simulink model "ABB_1010"  (R2024a)
settings: Solver=VariableStepAuto  StartTime=0.0  StopTime=200  RelTol=1e-3
model workspace: external: MATLAB File C:\Users\lucas\OneDrive\Documents\MATLAB\projeto final\ABB_1010_DataFile.m (data not in the file)
values from neighbouring files (symbols this model uses):
  g = 9.81    [inicializacaoAntropomorfico.m]
  I1 = [ 0.00243841  0.00000307  0.00007261    [inicializacaoAntropomorfico.m]
  I2 = [ 0.01633569  0.00000387 -0.00034405    [inicializacaoAntropomorfico.m]
  I3 = [ 0.00244760 -0.00000208  0.00000538    [inicializacaoAntropomorfico.m]
  I4 = [ 0.00245792 -0.00000008  0.00003121    [inicializacaoAntropomorfico.m]
  I5 = [ 0.00062165 -0.00000206 -0.00000303    [inicializacaoAntropomorfico.m]
  I6 = [ 0.00000357  0.00000000  0.00000000    [inicializacaoAntropomorfico.m]
  I7 = [(m7*L7^2)/12 0.00000000  0.00000000    [inicializacaoAntropomorfico.m]
  L = [L1, L2, L3, L4, L5, L6, L7]    [inicializacaoAntropomorfico.m]
  Lcm1 = [-0.00258308  0.00024508 -0.01434968]    [inicializacaoAntropomorfico.m]
  Lcm2 = [-0.02078894  0.00020016 -0.10516734]    [inicializacaoAntropomorfico.m]
  Lcm3 = [ 0.00021912  0.00015355 -0.06228290]    [inicializacaoAntropomorfico.m]
  Lcm4 = [-0.00172658 -0.00124140 -0.07369196]    [inicializacaoAntropomorfico.m]
  Lcm5 = [-0.00014110  0.00085992 -0.03825278]    [inicializacaoAntropomorfico.m]
  Lcm6 = [ 0.00002478  0.00000000 -0.00042157]    [inicializacaoAntropomorfico.m]
  Lcm7 = [ 0           0          -0.05000000]    [inicializacaoAntropomorfico.m]
  m = [m1, m2, m3, m4, m5, m6, m7]    [inicializacaoAntropomorfico.m]
  Pf = [  0.05    [inicializacaoAntropomorfico.m]
  Pi = [  0.2    [inicializacaoAntropomorfico.m]
  Raio = [0]    [inicializacaoAntropomorfico.m]
  Sentido = [0]    [inicializacaoAntropomorfico.m]
  Tipo = [1]    [inicializacaoAntropomorfico.m]
undefined symbols (not defined in the file or in its folder): smiData, X, Y, Z
libraries: sm_lib x35, nesl_utility x7
(part 8 of 16)

== matlab function ABB_1010/Dinamica/MATLAB Function3 ==
  data: Q input; I1 parameter; I2 parameter; L parameter; dQ input; Lcm1 parameter; Lcm2 parameter; Lcm3 parameter; Lcm4 parameter; Lcm5 parameter; Lcm6 parameter; I5 parameter; I4 parameter; I3 parameter; C output; I6 parameter; m parameter
function C = func_C(Q, I1, I2, L, dQ, Lcm1, Lcm2, Lcm3, Lcm4, Lcm5, Lcm6, I5, I4, I3, I6, m)
%func_C
%    OUT1 = func_C(Ixx2,Ixx3,Ixx4,Ixx5,Ixx6,Ixy3,Ixy4,Ixy5,Ixy6,Ixz2,Ixz3,Ixz4,Ixz5,Ixz6,Iyx3,Iyx4,Iyx5,Iyx6,Iyy4,Iyy5,Iyy6,Iyz3,Iyz4,Iyz5,Iyz6,Izx2,Izx3,Izx4,Izx5,Izx6,Izy3,Izy4,Izy5,Izy6,Izz2,Izz3,Izz4,Izz5,Izz6,Lx2,Lx3,Lxcm2,Lxcm3,Lxcm4,Lxcm5,Lxcm6,Lycm3,Lycm4,Lycm5,Lycm6,Lz4,Lz5,Lzcm2,Lzcm3,Lzcm4,Lzcm5,Lzcm6,Q2,Q3,Q4,Q5,Q6,dQ1,dQ2,dQ3,dQ4,dQ5,dQ6,M2,M3,M4,M5,M6)

%    This function was generated by the Symbolic Math Toolbox version 24.1.
%    30-Apr-2025 06:24:11

m1  = m(1);
m2  = m(2);
m3  = m(3);
m4  = m(4);
m5  = m(5);
m6  = m(6);

Q1  = Q(1);
Q2  = Q(2);
Q3  = Q(3);
Q4  = Q(4);
Q5  = Q(5);
Q6  = Q(6);

dQ1 = dQ(1);
dQ2 = dQ(2);
dQ3 = dQ(3);
dQ4 = dQ(4);
dQ5 = dQ(5);
dQ6 = dQ(6);

Lz1 = L(1);
Lx2 = L(2);
Lx3 = L(3);
Lz4 = L(4);
Lz5 = L(5);
Lz6 = L(6);

Lxcm1 = Lcm1(1);
Lycm1 = Lcm1(2);
Lzcm1 = Lcm1(3);

Lxcm2 = Lcm2(1);
Lycm2 = Lcm2(2);
Lzcm2 = Lcm2(3);

Lxcm3 = Lcm3(1);
Lycm3 = Lcm3(2);
Lzcm3 = Lcm3(3);

Lxcm4 = Lcm4(1);
Lycm4 = Lcm4(2);
Lzcm4 = Lcm4(3);

Lxcm5 = Lcm5(1);
Lycm5 = Lcm5(2);
Lzcm5 = Lcm5(3);

Lxcm6 = Lcm6(1);
Lycm6 = Lcm6(2);
Lzcm6 = Lcm6(3);

Ixx1 = I1(1,1);
Ixy1 = I1(1,2);
Ixz1 = I1(1,3);
Iyx1 = I1(2,1);
Iyy1 = I1(2,2);
Iyz1 = I1(2,3);
Izx1 = I1(3,1);
Izy1 = I1(3,2);
Izz1 = I1(3,3);

Ixx2 = I2(1,1);
Ixy2 = I2(1,2);
Ixz2 = I2(1,3);
Iyx2 = I2(2,1);
Iyy2 = I2(2,2);
Iyz2 = I2(2,3);
Izx2 = I2(3,1);
Izy2 = I2(3,2);
Izz2 = I2(3,3);

Ixx3 = I3(1,1);
Ixy3 = I3(1,2);
Ixz3 = I3(1,3);
Iyx3 = I3(2,1);
Iyy3 = I3(2,2);
Iyz3 = I3(2,3);
Izx3 = I3(3,1);
Izy3 = I3(3,2);
Izz3 = I3(3,3);

Ixx4 = I4(1,1);
Ixy4 = I4(1,2);
Ixz4 = I4(1,3);
Iyx4 = I4(2,1);
Iyy4 = I4(2,2);
Iyz4 = I4(2,3);
Izx4 = I4(3,1);
Izy4 = I4(3,2);
Izz4 = I4(3,3);

Ixx5 = I5(1,1);
Ixy5 = I5(1,2);
Ixz5 = I5(1,3);
Iyx5 = I5(2,1);
Iyy5 = I5(2,2);
Iyz5 = I5(2,3);
Izx5 = I5(3,1);
Izy5 = I5(3,2);
Izz5 = I5(3,3);

Ixx6 = I6(1,1);
Ixy6 = I6(1,2);
Ixz6 = I6(1,3);
Iyx6 = I6(2,1);
Iyy6 = I6(2,2);
Iyz6 = I6(2,3);
Izx6 = I6(3,1);
Izy6 = I6(3,2);
Izz6 = I6(3,3);

t2 = cos(Q2);
t3 = cos(Q3);
t4 = cos(Q4);
t5 = cos(Q5);
t6 = cos(Q6);
t7 = sin(Q2);
t8 = sin(Q3);
t9 = sin(Q4);
t10 = sin(Q5);
t11 = sin(Q6);
t12 = Lx2.^2;
t13 = Lx3.^2;
t14 = Lxcm3.^2;
t15 = Lxcm4.^2;
t16 = Lxcm5.^2;
t17 = Lxcm6.^2;
t18 = Lycm4.^2;
t19 = Lycm5.^2;
t20 = Lycm6.^2;
t21 = Lz4.^2;
t22 = Lz5.^2;
t23 = Lzcm3.^2;
t24 = Lzcm4.^2;
t25 = Lzcm5.^2;
t26 = Lzcm6.^2;
t27 = Q2.*2.0;
t28 = Q3.*2.0;
t29 = Q4.*2.0;
t30 = Q5.*2.0;
t31 = Q6.*2.0;
t42 = Ixy4.*dQ2.*dQ4;
t43 = Ixy4.*dQ3.*dQ4;
t44 = Ixz5.*dQ2.*dQ5;
t45 = Ixz5.*dQ3.*dQ5;
t46 = Iyx4.*dQ2.*dQ4;
t47 = Iyx4.*dQ3.*dQ4;
t48 = Izx5.*dQ2.*dQ5;
t49 = Izx5.*dQ3.*dQ5;
t78 = Lxcm4.*Lycm4.*dQ2.*dQ4.*m4.*2.0;
t79 = Lxcm4.*Lycm4.*dQ3.*dQ4.*m4.*2.0;
t80 = Lxcm5.*Lzcm5.*dQ2.*dQ5.*m5.*2.0;
t81 = Lxcm5.*Lzcm5.*dQ3.*dQ5.*m5.*2.0;
t32 = t2.^2;
t33 = t3.^2;
t34 = t4.^2;
t35 = t5.^2;
t36 = t6.^2;
t37 = sin(t27);
t38 = sin(t28);
t39 = sin(t29);
t40 = sin(t30);
t41 = sin(t31);
t50 = Ixy5.*dQ2.*dQ4.*t5;
t51 = Ixy5.*dQ3.*dQ4.*t5;
t52 = Ixy6.*dQ2.*dQ4.*t5;
t53 = Ixy6.*dQ3.*dQ4.*t5;
t54 = Ixy6.*dQ5.*dQ6.*t4;
t55 = Ixz6.*dQ2.*dQ5.*t6;
t56 = Ixz6.*dQ3.*dQ5.*t6;
t57 = Iyx5.*dQ2.*dQ4.*t5;
t58 = Iyx5.*dQ3.*dQ4.*t5;
t59 = Iyx6.*dQ2.*dQ4.*t5;
t60 = Iyx6.*dQ3.*dQ4.*t5;
t61 = Iyx6.*dQ5.*dQ6.*t4;
t62 = Izx6.*dQ2.*dQ5.*t6;
t63 = Izx6.*dQ3.*dQ5.*t6;
t64 = Ixx5.*dQ4.*dQ5.*t9;
t65 = Ixx6.*dQ4.*dQ5.*t9;
t66 = Iyy5.*dQ4.*dQ5.*t9;
t67 = Iyy6.*dQ4.*dQ5.*t9;
t68 = Iyz5.*dQ2.*dQ4.*t10;
t69 = Iyz5.*dQ3.*dQ4.*t10;
t70 = Iyz6.*dQ2.*dQ5.*t11;
t71 = Iyz6.*dQ3.*dQ5.*t11;
t72 = Izy5.*dQ2.*dQ4.*t10;
t73 = Izy5.*dQ3.*dQ4.*t10;
t74 = Izy6.*dQ2.*dQ5.*t11;
t75 = Izy6.*dQ3.*dQ5.*t11;
t76 = Izz5.*dQ4.*dQ5.*t9;
t77 = Izz6.*dQ4.*dQ5.*t9;
t126 = Ixx4.*dQ1.*dQ4.*t2.*t8;
t127 = Ixx4.*dQ1.*dQ4.*t3.*t7;
t128 = Ixx5.*dQ1.*dQ4.*t2.*t8;
t129 = Ixx5.*dQ1.*dQ4.*t3.*t7;
t130 = Ixx6.*dQ1.*dQ4.*t2.*t8;
t131 = Ixx6.*dQ1.*dQ4.*t3.*t7;
t132 = Ixx6.*dQ4.*dQ6.*t4.*t10;
t133 = Ixx6.*dQ5.*dQ6.*t5.*t9;
t134 = Iyy4.*dQ1.*dQ4.*t2.*t8;
t135 = Iyy4.*dQ1.*dQ4.*t3.*t7;
t136 = Iyy5.*dQ1.*dQ4.*t2.*t8;
t137 = Iyy5.*dQ1.*dQ4.*t3.*t7;
t138 = Iyy6.*dQ1.*dQ4.*t2.*t8;
t139 = Iyy6.*dQ1.*dQ4.*t3.*t7;
t140 = Iyy6.*dQ4.*dQ6.*t4.*t10;
t141 = Iyy6.*dQ5.*dQ6.*t5.*t9;
t142 = Iyz6.*dQ2.*dQ4.*t6.*t10;
t143 = Iyz6.*dQ3.*dQ4.*t6.*t10;
t144 = Izy6.*dQ2.*dQ4.*t6.*t10;
t145 = Izy6.*dQ3.*dQ4.*t6.*t10;
t146 = Izz4.*dQ1.*dQ4.*t2.*t8;
t147 = Izz4.*dQ1.*dQ4.*t3.*t7;
t148 = Izz5.*dQ1.*dQ4.*t2.*t8;
t149 = Izz5.*dQ1.*dQ4.*t3.*t7;
t150 = Izz6.*dQ1.*dQ4.*t2.*t8;
t151 = Izz6.*dQ1.*dQ4.*t3.*t7;
t152 = Izz6.*dQ4.*dQ6.*t4.*t10;
t153 = Izz6.*dQ5.*dQ6.*t5.*t9;
t154 = Ixz6.*dQ2.*dQ4.*t10.*t11;
t155 = Ixz6.*dQ3.*dQ4.*t10.*t11;
t156 = Izx6.*dQ2.*dQ4.*t10.*t11;
t157 = Izx6.*dQ3.*dQ4.*t10.*t11;
t166 = Lx3.*Lycm4.*dQ2.*dQ4.*m4.*t4.*2.0;
t167 = Lx3.*Lycm4.*dQ3.*dQ4.*m4.*t4.*2.0;
t168 = Lx3.*Lycm5.*dQ2.*dQ4.*m5.*t4.*2.0;
t169 = Lx3.*Lycm5.*dQ3.*dQ4.*m5.*t4.*2.0;
t170 = Lxcm5.*Lycm5.*dQ2.*dQ4.*m5.*t5.*2.0;
t171 = Lxcm5.*Lycm5.*dQ3.*dQ4.*m5.*t5.*2.0;
t172 = Lxcm6.*Lycm6.*dQ2.*dQ4.*m6.*t5.*2.0;
t173 = Lxcm6.*Lycm6.*dQ3.*dQ4.*m6.*t5.*2.0;
t174 = Lxcm6.*Lycm6.*dQ5.*dQ6.*m6.*t4.*2.0;
t175 = Lxcm5.*Lz4.*dQ2.*dQ5.*m5.*t5.*2.0;
t176 = Lxcm5.*Lz4.*dQ3.*dQ5.*m5.*t5.*2.0;
t177 = Lxcm6.*Lz5.*dQ2.*dQ5.*m6.*t6.*2.0;
t178 = Lxcm6.*Lz5.*dQ3.*dQ5.*m6.*t6.*2.0;
t179 = Lxcm6.*Lzcm6.*dQ2.*dQ5.*m6.*t6.*2.0;
t180 = Lxcm6.*Lzcm6.*dQ3.*dQ5.*m6.*t6.*2.0;
t181 = Lx3.*Lxcm4.*dQ2.*dQ4.*m4.*t9.*2.0;
t182 = Lx3.*Lxcm4.*dQ3.*dQ4.*m4.*t9.*2.0;
t183 = Lycm6.*Lz5.*dQ2.*dQ5.*m6.*t11.*2.0;
t184 = Lycm6.*Lz5.*dQ3.*dQ5.*m6.*t11.*2.0;
t185 = Lycm5.*Lzcm5.*dQ2.*dQ4.*m5.*t10.*2.0;
t186 = Lycm5.*Lzcm5.*dQ3.*dQ4.*m5.*t10.*2.0;
t187 = Lycm6.*Lzcm6.*dQ2.*dQ5.*m6.*t11.*2.0;
t188 = Lycm6.*Lzcm6.*dQ3.*dQ5.*m6.*t11.*2.0;
t189 = Lz4.*Lz5.*dQ2.*dQ5.*m6.*t10.*2.0;
t190 = Lz4.*Lz5.*dQ3.*dQ5.*m6.*t10.*2.0;
t191 = Lz4.*Lzcm5.*dQ2.*dQ5.*m5.*t10.*2.0;
t192 = Lz4.*Lzcm5.*dQ3.*dQ5.*m5.*t10.*2.0;
t193 = Lz4.*Lzcm6.*dQ2.*dQ5.*m6.*t10.*2.0;
t194 = Lz4.*Lzcm6.*dQ3.*dQ5.*m6.*t10.*2.0;
t195 = dQ4.*dQ5.*m5.*t9.*t16.*2.0;
t196 = dQ4.*dQ5.*m6.*t9.*t20.*2.0;
t221 = Ixz4.*dQ1.*dQ4.*t2.*t3.*t4;
t222 = Ixz5.*dQ1.*dQ4.*t2.*t3.*t4;
t223 = Ixz6.*dQ4.*dQ6.*t4.*t5.*t6;
t224 = Izx4.*dQ1.*dQ4.*t2.*t3.*t4;
t225 = Izx5.*dQ1.*dQ4.*t2.*t3.*t4;
t226 = Izx6.*dQ4.*dQ6.*t4.*t5.*t6;
t237 = Ixx5.*dQ1.*dQ5.*t2.*t3.*t9;
t238 = Ixx6.*dQ1.*dQ5.*t2.*t3.*t9;
t239 = Ixx6.*dQ1.*dQ6.*t2.*t5.*t8;
t240 = Ixx6.*dQ1.*dQ6.*t3.*t5.*t7;
t241 = Iyy5.*dQ1.*dQ5.*t2.*t3.*t9;
t242 = Iyy6.*dQ1.*dQ5.*t2.*t3.*t9;
t243 = Iyy6.*dQ1.*dQ6.*t2.*t5.*t8;
t244 = Iyy6.*dQ1.*dQ6.*t3.*t5.*t7;
t245 = Iyz4.*dQ1.*dQ4.*t2.*t3.*t9;
t246 = Iyz5.*dQ1.*dQ5.*t2.*t5.*t8;
t247 = Iyz5.*dQ1.*dQ5.*t3.*t5.*t7;
t248 = Iyz5.*dQ2.*dQ5.*t4.*t5.*t9;
t249 = Iyz5.*dQ3.*dQ5.*t4.*t5.*t9;
t250 = Iyz6.*dQ2.*dQ6.*t5.*t6.*t10;
t251 = Iyz6.*dQ3.*dQ6.*t5.*t6.*t10;
t252 = Iyz6.*dQ4.*dQ6.*t4.*t5.*t11;
t253 = Izy4.*dQ1.*dQ4.*t2.*t3.*t9;
t254 = Izy5.*dQ1.*dQ5.*t2.*t5.*t8;
t255 = Izy5.*dQ1.*dQ5.*t3.*t5.*t7;
t256 = Izy5.*dQ2.*dQ5.*t4.*t5.*t9;
t257 = Izy5.*dQ3.*dQ5.*t4.*t5.*t9;
t258 = Izy6.*dQ2.*dQ6.*t5.*t6.*t10;
t259 = Izy6.*dQ3.*dQ6.*t5.*t6.*t10;
t260 = Izy6.*dQ4.*dQ6.*t4.*t5.*t11;
t261 = Izz5.*dQ1.*dQ5.*t2.*t3.*t9;
t262 = Izz6.*dQ1.*dQ5.*t2.*t3.*t9;
t263 = Izz6.*dQ1.*dQ6.*t2.*t5.*t8;
t264 = Izz6.*dQ1.*dQ6.*t3.*t5.*t7;
t265 = Ixy5.*dQ1.*dQ5.*t2.*t8.*t10;
t266 = Ixy5.*dQ1.*dQ5.*t3.*t7.*t10;
t267 = Ixy6.*dQ1.*dQ5.*t2.*t8.*t10;
t268 = Ixy6.*dQ1.*dQ5.*t3.*t7.*t10;
t269 = Ixy5.*dQ2.*dQ5.*t4.*t9.*t10;
t270 = Ixy5.*dQ3.*dQ5.*t4.*t9.*t10;
t271 = Ixy6.*dQ2.*dQ5.*t4.*t9.*t10;
t272 = Ixy6.*dQ3.*dQ5.*t4.*t9.*t10;
t273 = Ixy6.*dQ4.*dQ6.*t5.*t9.*t10;
t274 = Ixz4.*dQ1.*dQ4.*t4.*t7.*t8;
t275 = Ixz5.*dQ1.*dQ4.*t4.*t7.*t8;
t276 = Ixz6.*dQ2.*dQ6.*t5.*t10.*t11;
t277 = Ixz6.*dQ3.*dQ6.*t5.*t10.*t11;
t278 = Iyx5.*dQ1.*dQ5.*t2.*t8.*t10;
t279 = Iyx5.*dQ1.*dQ5.*t3.*t7.*t10;
t280 = Iyx6.*dQ1.*dQ5.*t2.*t8.*t10;
t281 = Iyx6.*dQ1.*dQ5.*t3.*t7.*t10;
t282 = Iyx5.*dQ2.*dQ5.*t4.*t9.*t10;
t283 = Iyx5.*dQ3.*dQ5.*t4.*t9.*t10;
t284 = Iyx6.*dQ2.*dQ5.*t4.*t9.*t10;
t285 = Iyx6.*dQ3.*dQ5.*t4.*t9.*t10;
t286 = Iyx6.*dQ4.*dQ6.*t5.*t9.*t10;
t287 = Izx4.*dQ1.*dQ4.*t4.*t7.*t8;
t288 = Izx5.*dQ1.*dQ4.*t4.*t7.*t8;
t289 = Izx6.*dQ2.*dQ6.*t5.*t10.*t11;
t290 = Izx6.*dQ3.*dQ6.*t5.*t10.*t11;
t291 = Ixx5.*dQ1.*dQ5.*t7.*t8.*t9;
t292 = Ixx6.*dQ1.*dQ5.*t7.*t8.*t9;
t293 = Iyy5.*dQ1.*dQ5.*t7.*t8.*t9;
t294 = Iyy6.*dQ1.*dQ5.*t7.*t8.*t9;
t295 = Iyz4.*dQ1.*dQ4.*t7.*t8.*t9;
t296 = Izy4.*dQ1.*dQ4.*t7.*t8.*t9;
t297 = Izz5.*dQ1.*dQ5.*t7.*t8.*t9;
t298 = Izz6.*dQ1.*dQ5.*t7.*t8.*t9;
t399 = Lx3.*Lycm6.*dQ2.*dQ4.*m6.*t4.*t6.*2.0;
t400 = Lx3.*Lycm6.*dQ3.*dQ4.*m6.*t4.*t6.*2.0;
t401 = Lx3.*Lycm6.*dQ5.*dQ6.*m6.*t5.*t6.*2.0;
t402 = Lx3.*Lz5.*dQ2.*dQ5.*m6.*t4.*t5.*2.0;
t403 = Lx3.*Lz5.*dQ3.*dQ5.*m6.*t4.*t5.*2.0;
t404 = Lx3.*Lzcm5.*dQ2.*dQ5.*m5.*t4.*t5.*2.0;
t405 = Lx3.*Lzcm5.*dQ3.*dQ5.*m5.*t4.*t5.*2.0;
t406 = Lx3.*Lzcm6.*dQ2.*dQ5.*m6.*t4.*t5.*2.0;
t407 = Lx3.*Lzcm6.*dQ3.*dQ5.*m6.*t4.*t5.*2.0;
t408 = Lxcm6.*Lz4.*dQ2.*dQ5.*m6.*t5.*t6.*2.0;
t409 = Lxcm6.*Lz4.*dQ3.*dQ5.*m6.*t5.*t6.*2.0;
t410 = Lxcm6.*Lz4.*dQ4.*dQ6.*m6.*t4.*t6.*2.0;
t411 = Ixx6.*dQ2.*dQ6.*t4.*t5.*t9.*2.0;
t412 = Ixx6.*dQ3.*dQ6.*t4.*t5.*t9.*2.0;
t413 = Ixx6.*dQ2.*dQ4.*t5.*t6.*t11.*2.0;
t414 = Ixx6.*dQ3.*dQ4.*t5.*t6.*t11.*2.0;
t415 = Ixx6.*dQ5.*dQ6.*t4.*t6.*t11.*2.0;
t416 = Iyy6.*dQ2.*dQ6.*t4.*t5.*t9.*2.0;
t417 = Iyy6.*dQ3.*dQ6.*t4.*t5.*t9.*2.0;
t418 = Iyy6.*dQ2.*dQ4.*t5.*t6.*t11.*2.0;
t419 = Iyy6.*dQ3.*dQ4.*t5.*t6.*t11.*2.0;
t420 = Iyy6.*dQ5.*dQ6.*t4.*t6.*t11.*2.0;
t421 = Lx3.*Lxcm5.*dQ2.*dQ4.*m5.*t5.*t9.*2.0;
t422 = Lx3.*Lxcm5.*dQ2.*dQ5.*m5.*t4.*t10.*2.0;
t423 = Lx3.*Lxcm5.*dQ3.*dQ4.*m5.*t5.*t9.*2.0;
t424 = Lx3.*Lxcm5.*dQ3.*dQ5.*m5.*t4.*t10.*2.0;
t425 = Lx3.*Lxcm6.*dQ2.*dQ4.*m6.*t4.*t11.*2.0;
t426 = Lx3.*Lxcm6.*dQ3.*dQ4.*m6.*t4.*t11.*2.0;
t427 = Lx3.*Lxcm6.*dQ2.*dQ6.*m6.*t6.*t9.*2.0;
t428 = Lx3.*Lxcm6.*dQ3.*dQ6.*m6.*t6.*t9.*2.0;
t429 = Lx3.*Lxcm6.*dQ5.*dQ6.*m6.*t5.*t11.*2.0;
t430 = Lycm6.*Lz4.*dQ2.*dQ5.*m6.*t5.*t11.*2.0;
t431 = Lycm6.*Lz5.*dQ2.*dQ4.*m6.*t6.*t10.*2.0;
t432 = Lycm6.*Lz4.*dQ2.*dQ6.*m6.*t6.*t10.*2.0;
t433 = Lycm6.*Lz4.*dQ3.*dQ5.*m6.*t5.*t11.*2.0;
t434 = Lycm6.*Lz5.*dQ3.*dQ4.*m6.*t6.*t10.*2.0;
t435 = Lycm6.*Lz4.*dQ3.*dQ6.*m6.*t6.*t10.*2.0;
t436 = Lycm6.*Lz4.*dQ4.*dQ6.*m6.*t4.*t11.*2.0;
t437 = Lycm6.*Lzcm6.*dQ2.*dQ4.*m6.*t6.*t10.*2.0;
t438 = Lycm6.*Lzcm6.*dQ3.*dQ4.*m6.*t6.*t10.*2.0;
t439 = Lz4.*Lz5.*dQ4.*dQ5.*m6.*t5.*t9.*2.0;
t440 = Lz4.*Lzcm5.*dQ4.*dQ5.*m5.*t5.*t9.*2.0;
t441 = Lz4.*Lzcm6.*dQ4.*dQ5.*m6.*t5.*t9.*2.0;
t442 = Ixy6.*dQ4.*dQ5.*t6.*t9.*t11.*2.0;
t443 = Ixz5.*dQ4.*dQ5.*t5.*t9.*t10.*2.0;
t444 = Iyx6.*dQ4.*dQ5.*t6.*t9.*t11.*2.0;
t445 = Izx5.*dQ4.*dQ5.*t5.*t9.*t10.*2.0;
t446 = Lx3.*Lycm6.*dQ2.*dQ6.*m6.*t9.*t11.*2.0;
t447 = Lx3.*Lycm6.*dQ3.*dQ6.*m6.*t9.*t11.*2.0;
t448 = Lx3.*Lz5.*dQ2.*dQ4.*m6.*t9.*t10.*2.0;
t449 = Lx3.*Lz5.*dQ3.*dQ4.*m6.*t9.*t10.*2.0;
t450 = Lx3.*Lzcm5.*dQ2.*dQ4.*m5.*t9.*t10.*2.0;
t451 = Lx3.*Lzcm5.*dQ3.*dQ4.*m5.*t9.*t10.*2.0;
t452 = Lx3.*Lzcm6.*dQ2.*dQ4.*m6.*t9.*t10.*2.0;
t453 = Lx3.*Lzcm6.*dQ3.*dQ4.*m6.*t9.*t10.*2.0;
t454 = Lxcm5.*Lz4.*dQ4.*dQ5.*m5.*t9.*t10.*2.0;
t455 = Lxcm6.*Lz5.*dQ2.*dQ4.*m6.*t10.*t11.*2.0;
t456 = Lxcm6.*Lz4.*dQ2.*dQ6.*m6.*t10.*t11.*2.0;
t457 = Lxcm6.*Lz5.*dQ3.*dQ4.*m6.*t10.*t11.*2.0;
t458 = Lxcm6.*Lz4.*dQ3.*dQ6.*m6.*t10.*t11.*2.0;
t459 = Lxcm6.*Lzcm6.*dQ2.*dQ4.*m6.*t10.*t11.*2.0;
t460 = Lxcm6.*Lzcm6.*dQ3.*dQ4.*m6.*t10.*t11.*2.0;
t485 = Ixz6.*dQ1.*dQ4.*t2.*t3.*t4.*t6;
t486 = Izx6.*dQ1.*dQ4.*t2.*t3.*t4.*t6;
t498 = Ixx6.*dQ1.*dQ6.*t2.*t3.*t4.*t10;
t499 = Iyy6.*dQ1.*dQ6.*t2.*t3.*t4.*t10;
t500 = Iyz5.*dQ1.*dQ4.*t2.*t3.*t5.*t9;
t501 = Iyz6.*dQ1.*dQ4.*t2.*t3.*t4.*t11;
t502 = Iyz6.*dQ1.*dQ5.*t2.*t5.*t6.*t8;
t503 = Iyz6.*dQ1.*dQ5.*t3.*t5.*t6.*t7;
t504 = Iyz6.*dQ2.*dQ5.*t4.*t5.*t6.*t9;
t505 = Iyz6.*dQ3.*dQ5.*t4.*t5.*t6.*t9;
t506 = Izy5.*dQ1.*dQ4.*t2.*t3.*t5.*t9;
t507 = Izy6.*dQ1.*dQ4.*t2.*t3.*t4.*t11;
t508 = Izy6.*dQ1.*dQ5.*t2.*t5.*t6.*t8;
t509 = Izy6.*dQ1.*dQ5.*t3.*t5.*t6.*t7;
t510 = Izy6.*dQ2.*dQ5.*t4.*t5.*t6.*t9;
t511 = Izy6.*dQ3.*dQ5.*t4.*t5.*t6.*t9;
t512 = Izz6.*dQ1.*dQ6.*t2.*t3.*t4.*t10;
t513 = Ixy5.*dQ1.*dQ4.*t2.*t3.*t9.*t10;
t514 = Ixy6.*dQ1.*dQ4.*t2.*t3.*t9.*t10;
t515 = Ixy6.*dQ1.*dQ6.*t2.*t4.*t8.*t9;
t516 = Ixy6.*dQ1.*dQ6.*t3.*t4.*t7.*t9;
t517 = Ixz5.*dQ1.*dQ5.*t2.*t4.*t8.*t9;
t518 = Ixz5.*dQ1.*dQ5.*t3.*t4.*t7.*t9;
t519 = Ixz6.*dQ1.*dQ4.*t4.*t6.*t7.*t8;
t520 = Ixz6.*dQ1.*dQ5.*t2.*t5.*t8.*t11;
t521 = Ixz6.*dQ1.*dQ5.*t3.*t5.*t7.*t11;
t522 = Ixz6.*dQ2.*dQ5.*t4.*t5.*t9.*t11;
t523 = Ixz6.*dQ2.*dQ6.*t4.*t6.*t9.*t10;
t524 = Ixz6.*dQ3.*dQ5.*t4.*t5.*t9.*t11;
t525 = Ixz6.*dQ3.*dQ6.*t4.*t6.*t9.*t10;
t526 = Iyx5.*dQ1.*dQ4.*t2.*t3.*t9.*t10;
t527 = Iyx6.*dQ1.*dQ4.*t2.*t3.*t9.*t10;
t528 = Iyx6.*dQ1.*dQ6.*t2.*t4.*t8.*t9;
t529 = Iyx6.*dQ1.*dQ6.*t3.*t4.*t7.*t9;
t530 = Izx5.*dQ1.*dQ5.*t2.*t4.*t8.*t9;
t531 = Izx5.*dQ1.*dQ5.*t3.*t4.*t7.*t9;
t532 = Izx6.*dQ1.*dQ4.*t4.*t6.*t7.*t8;
t533 = Izx6.*dQ1.*dQ5.*t2.*t5.*t8.*t11;
t534 = Izx6.*dQ1.*dQ5.*t3.*t5.*t7.*t11;
t535 = Izx6.*dQ2.*dQ5.*t4.*t5.*t9.*t11;
t536 = Izx6.*dQ2.*dQ6.*t4.*t6.*t9.*t10;
t537 = Izx6.*dQ3.*dQ5.*t4.*t5.*t9.*t11;
t538 = Izx6.*dQ3.*dQ6.*t4.*t6.*t9.*t10;
t539 = Ixx6.*dQ1.*dQ6.*t4.*t7.*t8.*t10;
t540 = Iyy6.*dQ1.*dQ6.*t4.*t7.*t8.*t10;
t541 = Iyz5.*dQ1.*dQ4.*t5.*t7.*t8.*t9;
t542 = Iyz6.*dQ1.*dQ4.*t4.*t7.*t8.*t11;
t543 = Iyz6.*dQ2.*dQ6.*t4.*t9.*t10.*t11;
t544 = Iyz6.*dQ3.*dQ6.*t4.*t9.*t10.*t11;
t545 = Izy5.*dQ1.*dQ4.*t5.*t7.*t8.*t9;
t546 = Izy6.*dQ1.*dQ4.*t4.*t7.*t8.*t11;
t547 = Izy6.*dQ2.*dQ6.*t4.*t9.*t10.*t11;
t548 = Izy6.*dQ3.*dQ6.*t4.*t9.*t10.*t11;
t549 = Izz6.*dQ1.*dQ6.*t4.*t7.*t8.*t10;
t550 = Ixy5.*dQ1.*dQ4.*t7.*t8.*t9.*t10;
t551 = Ixy6.*dQ1.*dQ4.*t7.*t8.*t9.*t10;
t552 = Iyx5.*dQ1.*dQ4.*t7.*t8.*t9.*t10;
t553 = Iyx6.*dQ1.*dQ4.*t7.*t8.*t9.*t10;
t615 = dQ1.*dQ4.*m6.*t2.*t8.*t17.*2.0;
t616 = dQ1.*dQ4.*m6.*t3.*t7.*t17.*2.0;
t617 = dQ5.*dQ6.*m6.*t5.*t9.*t17.*2.0;
t618 = dQ1.*dQ4.*m4.*t2.*t8.*t18.*2.0;
t619 = dQ1.*dQ4.*m4.*t3.*t7.*t18.*2.0;
t620 = dQ1.*dQ4.*m5.*t2.*t8.*t19.*2.0;
t621 = dQ1.*dQ4.*m5.*t3.*t7.*t19.*2.0;
t622 = dQ4.*dQ6.*m6.*t4.*t10.*t20.*2.0;
t644 = Lx3.*Lycm6.*dQ2.*dQ6.*m6.*t4.*t5.*t6.*2.0;
t645 = Lx3.*Lycm6.*dQ3.*dQ6.*m6.*t4.*t5.*t6.*2.0;
t646 = Lxcm6.*Lz5.*dQ4.*dQ6.*m6.*t4.*t5.*t6.*2.0;
t647 = Lxcm4.*Lzcm4.*dQ1.*dQ4.*m4.*t2.*t3.*t4.*2.0;
t648 = Lxcm5.*Lzcm5.*dQ1.*dQ4.*m5.*t2.*t3.*t4.*2.0;
t649 = Lxcm6.*Lzcm6.*dQ4.*dQ6.*m6.*t4.*t5.*t6.*2.0;
t650 = Lx3.*Lxcm4.*dQ1.*dQ4.*m4.*t2.*t4.*t8.*2.0;
t651 = Lx3.*Lxcm4.*dQ1.*dQ4.*m4.*t3.*t4.*t7.*2.0;
t652 = Lx3.*Lxcm6.*dQ2.*dQ4.*m6.*t5.*t6.*t9.*2.0;
t653 = Lx3.*Lxcm6.*dQ2.*dQ5.*m6.*t4.*t6.*t10.*2.0;
t654 = Lx3.*Lxcm6.*dQ3.*dQ4.*m6.*t5.*t6.*t9.*2.0;
t655 = Lx3.*Lxcm6.*dQ2.*dQ6.*m6.*t4.*t5.*t11.*2.0;
t656 = Lx3.*Lxcm6.*dQ3.*dQ5.*m6.*t4.*t6.*t10.*2.0;
t657 = Lx3.*Lxcm6.*dQ3.*dQ6.*m6.*t4.*t5.*t11.*2.0;
t658 = Lycm5.*Lz4.*dQ1.*dQ4.*m5.*t2.*t3.*t9.*2.0;
t659 = Lycm6.*Lz4.*dQ4.*dQ6.*m6.*t5.*t6.*t9.*2.0;
t660 = Lycm6.*Lz5.*dQ2.*dQ6.*m6.*t5.*t6.*t10.*2.0;
t661 = Lycm6.*Lz4.*dQ5.*dQ6.*m6.*t4.*t6.*t10.*2.0;
t662 = Lycm6.*Lz5.*dQ3.*dQ6.*m6.*t5.*t6.*t10.*2.0;
t663 = Lycm6.*Lz5.*dQ4.*dQ6.*m6.*t4.*t5.*t11.*2.0;
t664 = Lycm4.*Lzcm4.*dQ1.*dQ4.*m4.*t2.*t3.*t9.*2.0;
t665 = Lycm5.*Lzcm5.*dQ1.*dQ5.*m5.*t2.*t5.*t8.*2.0;
t666 = Lycm5.*Lzcm5.*dQ1.*dQ5.*m5.*t3.*t5.*t7.*2.0;
t667 = Lycm5.*Lzcm5.*dQ2.*dQ5.*m5.*t4.*t5.*t9.*2.0;
t668 = Lycm5.*Lzcm5.*dQ3.*dQ5.*m5.*t4.*t5.*t9.*2.0;
t669 = Lycm6.*Lzcm6.*dQ2.*dQ6.*m6.*t5.*t6.*t10.*2.0;
t670 = Lycm6.*Lzcm6.*dQ3.*dQ6.*m6.*t5.*t6.*t10.*2.0;
t671 = Lycm6.*Lzcm6.*dQ4.*dQ6.*m6.*t4.*t5.*t11.*2.0;
t672 = Ixy4.*dQ1.*dQ4.*t2.*t4.*t8.*t9.*2.0;
t673 = Ixy4.*dQ1.*dQ4.*t3.*t4.*t7.*t9.*2.0;
t674 = Ixy6.*dQ1.*dQ4.*t2.*t6.*t8.*t11.*2.0;
t675 = Ixy6.*dQ1.*dQ4.*t3.*t6.*t7.*t11.*2.0;
t676 = Ixy6.*dQ2.*dQ4.*t4.*t6.*t9.*t11.*2.0;
t677 = Ixy6.*dQ3.*dQ4.*t4.*t6.*t9.*t11.*2.0;
t678 = Ixy6.*dQ2.*dQ5.*t5.*t6.*t10.*t11.*2.0;
t679 = Ixy6.*dQ3.*dQ5.*t5.*t6.*t10.*t11.*2.0;
t680 = Ixy6.*dQ4.*dQ6.*t4.*t6.*t10.*t11.*2.0;
t681 = Ixy6.*dQ5.*dQ6.*t5.*t6.*t9.*t11.*2.0;
t682 = Ixz5.*dQ2.*dQ4.*t4.*t5.*t9.*t10.*2.0;
t683 = Ixz5.*dQ3.*dQ4.*t4.*t5.*t9.*t10.*2.0;
t684 = Ixz6.*dQ4.*dQ5.*t5.*t6.*t9.*t10.*2.0;
t685 = Iyx4.*dQ1.*dQ4.*t2.*t4.*t8.*t9.*2.0;
t686 = Iyx4.*dQ1.*dQ4.*t3.*t4.*t7.*t9.*2.0;
t687 = Iyx6.*dQ1.*dQ4.*t2.*t6.*t8.*t11.*2.0;
t688 = Iyx6.*dQ1.*dQ4.*t3.*t6.*t7.*t11.*2.0;
t689 = Iyx6.*dQ2.*dQ4.*t4.*t6.*t9.*t11.*2.0;
t690 = Iyx6.*dQ3.*dQ4.*t4.*t6.*t9.*t11.*2.0;
t691 = Iyx6.*dQ2.*dQ5.*t5.*t6.*t10.*t11.*2.0;
t692 = Iyx6.*dQ3.*dQ5.*t5.*t6.*t10.*t11.*2.0;
t693 = Iyx6.*dQ4.*dQ6.*t4.*t6.*t10.*t11.*2.0;
t694 = Iyx6.*dQ5.*dQ6.*t5.*t6.*t9.*t11.*2.0;
t695 = Izx5.*dQ2.*dQ4.*t4.*t5.*t9.*t10.*2.0;
t696 = Izx5.*dQ3.*dQ4.*t4.*t5.*t9.*t10.*2.0;
t697 = Izx6.*dQ4.*dQ5.*t5.*t6.*t9.*t10.*2.0;
t712 = Lx3.*Lycm4.*dQ1.*dQ4.*m4.*t2.*t8.*t9.*2.0;
t713 = Lx3.*Lycm4.*dQ1.*dQ4.*m4.*t3.*t7.*t9.*2.0;
t714 = Lx3.*Lycm5.*dQ1.*dQ4.*m5.*t2.*t8.*t9.*2.0;
t715 = Lx3.*Lycm5.*dQ1.*dQ4.*m5.*t3.*t7.*t9.*2.0;
t716 = Lx3.*Lycm6.*dQ2.*dQ4.*m6.*t5.*t9.*t11.*2.0;
t717 = Lx3.*Lycm6.*dQ2.*dQ5.*m6.*t4.*t10.*t11.*2.0;
t718 = Lx3.*Lycm6.*dQ3.*dQ4.*m6.*t5.*t9.*t11.*2.0;
t719 = Lx3.*Lycm6.*dQ3.*dQ5.*m6.*t4.*t10.*t11.*2.0;
t720 = Lxcm5.*Lycm5.*dQ1.*dQ5.*m5.*t2.*t8.*t10.*2.0;
t721 = Lxcm5.*Lycm5.*dQ1.*dQ5.*m5.*t3.*t7.*t10.*2.0;
t722 = Lxcm6.*Lycm6.*dQ1.*dQ5.*m6.*t2.*t8.*t10.*2.0;
t723 = Lxcm6.*Lycm6.*dQ1.*dQ5.*m6.*t3.*t7.*t10.*2.0;
t724 = Lxcm5.*Lycm5.*dQ2.*dQ5.*m5.*t4.*t9.*t10.*2.0;
t725 = Lxcm5.*Lycm5.*dQ3.*dQ5.*m5.*t4.*t9.*t10.*2.0;
t726 = Lxcm6.*Lycm6.*dQ2.*dQ5.*m6.*t4.*t9.*t10.*2.0;
t727 = Lxcm6.*Lycm6.*dQ3.*dQ5.*m6.*t4.*t9.*t10.*2.0;
t728 = Lxcm6.*Lycm6.*dQ4.*dQ6.*m6.*t5.*t9.*t10.*2.0;
t729 = Lxcm6.*Lycm6.*dQ4.*dQ5.*m6.*t6.*t9.*t11.*4.0;
t730 = Lxcm6.*Lz4.*dQ4.*dQ5.*m6.*t6.*t9.*t10.*2.0;
t731 = Lxcm6.*Lz4.*dQ4.*dQ6.*m6.*t5.*t9.*t11.*2.0;
t732 = Lxcm6.*Lz5.*dQ2.*dQ6.*m6.*t5.*t10.*t11.*2.0;
t733 = Lxcm6.*Lz4.*dQ5.*dQ6.*m6.*t4.*t10.*t11.*2.0;
t734 = Lxcm6.*Lz5.*dQ3.*dQ6.*m6.*t5.*t10.*t11.*2.0;
t735 = Lxcm4.*Lzcm4.*dQ1.*dQ4.*m4.*t4.*t7.*t8.*2.0;
t736 = Lxcm5.*Lzcm5.*dQ1.*dQ4.*m5.*t4.*t7.*t8.*2.0;
t737 = Lxcm5.*Lzcm5.*dQ4.*dQ5.*m5.*t5.*t9.*t10.*4.0;
t738 = Lxcm6.*Lzcm6.*dQ2.*dQ6.*m6.*t5.*t10.*t11.*2.0;
t739 = Lxcm6.*Lzcm6.*dQ3.*dQ6.*m6.*t5.*t10.*t11.*2.0;
t740 = Iyz6.*dQ4.*dQ5.*t5.*t9.*t10.*t11.*2.0;
t741 = Izy6.*dQ4.*dQ5.*t5.*t9.*t10.*t11.*2.0;
t742 = Lycm5.*Lz4.*dQ1.*dQ4.*m5.*t7.*t8.*t9.*2.0;
t743 = Lycm6.*Lz4.*dQ4.*dQ5.*m6.*t9.*t10.*t11.*2.0;
t744 = Lycm4.*Lzcm4.*dQ1.*dQ4.*m4.*t7.*t8.*t9.*2.0;
t831 = Iyz6.*dQ1.*dQ4.*t2.*t3.*t5.*t6.*t9;
t832 = Iyz6.*dQ1.*dQ6.*t2.*t3.*t4.*t5.*t11;
t833 = Izy6.*dQ1.*dQ4.*t2.*t3.*t5.*t6.*t9;
t834 = Izy6.*dQ1.*dQ6.*t2.*t3.*t4.*t5.*t11;
t839 = Ixy6.*dQ1.*dQ6.*t2.*t3.*t5.*t9.*t10;
t840 = Ixz6.*dQ1.*dQ4.*t2.*t3.*t5.*t9.*t11;
t841 = Ixz6.*dQ1.*dQ5.*t2.*t4.*t6.*t8.*t9;
t842 = Ixz6.*dQ1.*dQ5.*t3.*t4.*t6.*t7.*t9;
t843 = Ixz6.*dQ1.*dQ6.*t4.*t5.*t6.*t7.*t8;
t844 = Iyx6.*dQ1.*dQ6.*t2.*t3.*t5.*t9.*t10;
t845 = Izx6.*dQ1.*dQ4.*t2.*t3.*t5.*t9.*t11;
t846 = Izx6.*dQ1.*dQ5.*t2.*t4.*t6.*t8.*t9;
t847 = Izx6.*dQ1.*dQ5.*t3.*t4.*t6.*t7.*t9;
t848 = Izx6.*dQ1.*dQ6.*t4.*t5.*t6.*t7.*t8;
t856 = Iyz6.*dQ1.*dQ4.*t5.*t6.*t7.*t8.*t9;
t857 = Iyz6.*dQ1.*dQ5.*t2.*t4.*t8.*t9.*t11;
t858 = Iyz6.*dQ1.*dQ5.*t3.*t4.*t7.*t9.*t11;
t859 = Iyz6.*dQ1.*dQ6.*t4.*t5.*t7.*t8.*t11;
t860 = Izy6.*dQ1.*dQ4.*t5.*t6.*t7.*t8.*t9;
t861 = Izy6.*dQ1.*dQ5.*t2.*t4.*t8.*t9.*t11;
t862 = Izy6.*dQ1.*dQ5.*t3.*t4.*t7.*t9.*t11;
t863 = Izy6.*dQ1.*dQ6.*t4.*t5.*t7.*t8.*t11;
t864 = Ixy6.*dQ1.*dQ6.*t5.*t7.*t8.*t9.*t10;
t865 = Ixz6.*dQ1.*dQ4.*t5.*t7.*t8.*t9.*t11;
t866 = Iyx6.*dQ1.*dQ6.*t5.*t7.*t8.*t9.*t10;
t867 = Izx6.*dQ1.*dQ4.*t5.*t7.*t8.*t9.*t11;
t937 = dQ1.*dQ5.*m5.*t2.*t3.*t9.*t16.*2.0;
t938 = dQ1.*dQ6.*m6.*t2.*t5.*t8.*t17.*2.0;
t939 = dQ1.*dQ6.*m6.*t3.*t5.*t7.*t17.*2.0;
t940 = dQ2.*dQ6.*m6.*t4.*t5.*t9.*t17.*2.0;
t941 = dQ3.*dQ6.*m6.*t4.*t5.*t9.*t17.*2.0;
t942 = dQ2.*dQ4.*m6.*t5.*t6.*t11.*t17.*2.0;
t943 = dQ3.*dQ4.*m6.*t5.*t6.*t11.*t17.*2.0;
t944 = dQ5.*dQ6.*m6.*t4.*t6.*t11.*t17.*2.0;
t945 = dQ1.*dQ5.*m6.*t2.*t3.*t9.*t20.*2.0;
t946 = dQ2.*dQ6.*m6.*t4.*t5.*t9.*t20.*2.0;
t947 = dQ3.*dQ6.*m6.*t4.*t5.*t9.*t20.*2.0;
t948 = dQ2.*dQ4.*m6.*t5.*t6.*t11.*t20.*2.0;
t949 = dQ3.*dQ4.*m6.*t5.*t6.*t11.*t20.*2.0;
t950 = dQ5.*dQ6.*m6.*t4.*t6.*t11.*t20.*2.0;
t962 = dQ1.*dQ5.*m5.*t7.*t8.*t9.*t16.*2.0;
t963 = dQ1.*dQ5.*m6.*t7.*t8.*t9.*t20.*2.0;
t999 = Ixz6.*dQ1.*dQ6.*t2.*t3.*t4.*t5.*t6;
t1000 = Izx6.*dQ1.*dQ6.*t2.*t3.*t4.*t5.*t6;
t1031 = Ixx5.*dQ1.*dQ4.*t2.*t3.*t4.*t5.*t10.*2.0;
t1032 = Iyy6.*dQ1.*dQ4.*t2.*t3.*t4.*t5.*t10.*2.0;
t1033 = Izz5.*dQ1.*dQ4.*t2.*t3.*t4.*t5.*t10.*2.0;
t1034 = Izz6.*dQ1.*dQ4.*t2.*t3.*t4.*t5.*t10.*2.0;
t1035 = Lx3.*Lxcm5.*dQ1.*dQ4.*m5.*t2.*t4.*t5.*t8.*2.0;
t1036 = Lx3.*Lxcm5.*dQ1.*dQ4.*m5.*t3.*t4.*t5.*t7.*2.0;
t1037 = Lx3.*Lxcm6.*dQ1.*dQ6.*m6.*t2.*t4.*t6.*t8.*2.0;
t1038 = Lx3.*Lxcm6.*dQ1.*dQ6.*m6.*t3.*t4.*t6.*t7.*2.0;
t1039 = Lycm6.*Lz4.*dQ1.*dQ4.*m6.*t2.*t3.*t6.*t9.*2.0;
t1040 = Lycm6.*Lz5.*dQ1.*dQ4.*m6.*t2.*t3.*t4.*t11.*2.0;
t1041 = Lycm6.*Lz4.*dQ1.*dQ6.*m6.*t2.*t3.*t4.*t11.*2.0;
t1042 = Lycm6.*Lz5.*dQ1.*dQ5.*m6.*t2.*t5.*t6.*t8.*2.0;
t1043 = Lycm6.*Lz5.*dQ1.*dQ5.*m6.*t3.*t5.*t6.*t7.*2.0;
t1044 = Lycm6.*Lz5.*dQ2.*dQ5.*m6.*t4.*t5.*t6.*t9.*2.0;
t1045 = Lycm6.*Lz5.*dQ3.*dQ5.*m6.*t4.*t5.*t6.*t9.*2.0;
t1046 = Lycm5.*Lzcm5.*dQ1.*dQ4.*m5.*t2.*t3.*t5.*t9.*2.0;
t1047 = Lycm6.*Lzcm6.*dQ1.*dQ4.*m6.*t2.*t3.*t4.*t11.*2.0;
t1048 = Lycm6.*Lzcm6.*dQ1.*dQ5.*m6.*t2.*t5.*t6.*t8.*2.0;
t1049 = Lycm6.*Lzcm6.*dQ1.*dQ5.*m6.*t3.*t5.*t6.*t7.*2.0;
t1050 = Lycm6.*Lzcm6.*dQ2.*dQ5.*m6.*t4.*t5.*t6.*t9.*2.0;
t1051 = Lycm6.*Lzcm6.*dQ3.*dQ5.*m6.*t4.*t5.*t6.*t9.*2.0;
t1052 = Lz4.*Lz5.*dQ1.*dQ4.*m6.*t2.*t3.*t4.*t10.*2.0;
t1053 = Lz4.*Lz5.*dQ1.*dQ5.*m6.*t2.*t3.*t5.*t9.*2.0;
t1054 = Lz4.*Lzcm5.*dQ1.*dQ4.*m5.*t2.*t3.*t4.*t10.*2.0;
t1055 = Lz4.*Lzcm5.*dQ1.*dQ5.*m5.*t2.*t3.*t5.*t9.*2.0;
t1056 = Lz4.*Lzcm6.*dQ1.*dQ4.*m6.*t2.*t3.*t4.*t10.*2.0;
t1057 = Lz4.*Lzcm6.*dQ1.*dQ5.*m6.*t2.*t3.*t5.*t9.*2.0;
t1058 = Ixy5.*dQ1.*dQ4.*t2.*t4.*t5.*t8.*t9.*2.0;
t1059 = Ixy5.*dQ1.*dQ4.*t3.*t4.*t5.*t7.*t9.*2.0;
t1060 = Ixy6.*dQ1.*dQ4.*t2.*t4.*t5.*t8.*t9.*2.0;
C = ft_1({Ixx2,Ixx3,Ixx4,Ixx5,Ixx6,Ixy3,Ixy4,Ixy5,Ixy6,Ixz2,Ixz3,Ixz4,Ixz5,Ixz6,Iyx3,Iyx4,Iyx5,Iyx6,Iyy4,Iyy5,Iyy6,Iyz3,Iyz4,Iyz5,Iyz6,Izx2,Izx3,Izx4,Izx5,Izx6,Izy3,Izy4,Izy5,Izy6,Izz2,Izz3,Izz4,Izz5,Izz6,Lx2,Lx3,Lxcm2,Lxcm3,Lxcm4,Lxcm5,Lxcm6,Lycm3,Lycm4,Lycm5,Lycm6,Lz4,Lz5,Lzcm2,Lzcm3,Lzcm4,Lzcm5,Lzcm6,dQ1,dQ2,dQ3,dQ4,dQ5,dQ6,m2,m3,m4,m5,m6,t10,t1000,t1031,t1032,t1033,t1034,t1035,t1036,t1037,t1038,t1039,t1040,t1041,t1042,t1043,t1044,t1045,t1046,t1047,t1048,t1049,t1050,t1051,t1052,t1053,t1054,t1055,t1056,t1057,t1058,t1059,t1060,t11,t12,t126,t127,t128,t129,t13,t130,t131,t132,t133,t134,t135,t136,t137,t138,t139,t14,t140,t141,t142,t143,t144,t145,t146,t147,t148,t149,t15,t150,t151,t152,t153,t154,t155,t156,t157,t16,t166,t167,t168,t169,t17,t170,t171,t172,t173,t174,t175,t176,t177,t178,t179,t18,t180,t181,t182,t183,t184,t185,t186,t187,t188,t189,t19,t190,t191,t192,t193,t194,t195,t196,t2,t20,t21,t22,t221,t222,t223,t224,t225,t226,t23,t237,t238,t239,t24,t240,t241,t242,t243,t244,t245,t246,t247,t248,t249,t25,t250,t251,t252,t253,t254,t255,t256,t257,t258,t259,t26,t260,t261,t262,t263,t264,t265,t266,t267,t268,t269,t270,t271,t272,t273,t274,t275,t276,t277,t278,t279,t280,t281,t282,t283,t284,t285,t286,t287,t288,t289,t290,t291,t292,t293,t294,t295,t296,t297,t298,t3,t32,t33,t34,t35,t36,t37,t38,t39,t399,t4,t40,t400,t401,t402,t403,t404,t405,t406,t407,t408,t409,t41,t410,t411,t412,t413,t414,t415,t416,t417,t418,t419,t42,t420,t421,t422,t423,t424,t425,t426,t427,t428,t429,t43,t430,t431,t432,t433,t434,t435,t436,t437,t438,t439,t44,t440,t441,t442,t443,t444,t445,t446,t447,t448,t449,t45,t450,t451,t452,t453,t454,t455,t456,t457,t458,t459,t46,t460,t47,t48,t485,t486,t49,t498,t499,t5,t50,t500,t501,t502,t503,t504,t505,t506,t507,t508,t509,t51,t510,t511,t512,t513,t514,t515,t516,t517,t518,t519,t52,t520,t521,t522,t523,t524,t525,t526,t527,t528,t529,t53,t530,t531,t532,t533,t534,t535,t536,t537,t538,t539,t54,t540,t541,t542,t543,t544,t545,t546,t547,t548,t549,t55,t550,t551,t552,t553,t56,t57,t58,t59,t6,t60,t61,t615,t616,t617,t618,t619,t62,t620,t621,t622,t63,t64,t644,t645,t646,t647,t648,t649,t65,t650,t651,t652,t653,t654,t655,t656,t657,t658,t659,t66,t660,t661,t662,t663,t664,t665,t666,t667,t668,t669,t67,t670,t671,t672,t673,t674,t675,t676,t677,t678,t679,t68,t680,t681,t682,t683,t684,t685,t686,t687,t688,t689,t69,t690,t691,t692,t693,t694,t695,t696,t697,t7,t70,t71,t712,t713,t714,t715,t716,t717,t718,t719,t72,t720,t721,t722,t723,t724,t725,t726,t727,t728,t729,t73,t730,t731,t732,t733,t734,t735,t736,t737,t738,t739,t74,t740,t741,t742,t743,t744,t75,t76,t77,t78,t79,t8,t80,t81,t831,t832,t833,t834,t839,t840,t841,t842,t843,t844,t845,t846,t847,t848,t856,t857,t858,t859,t860,t861,t862,t863,t864,t865,t866,t867,t9,t937,t938,t939,t940,t941,t942,t943,t944,t945,t946,t947,t948,t949,t950,t962,t963,t999});
end
function out1 = ft_1(ct)
[Ixx2,Ixx3,Ixx4,Ixx5,Ixx6,Ixy3,Ixy4,Ixy5,Ixy6,Ixz2,Ixz3,Ixz4,Ixz5,Ixz6,Iyx3,Iyx4,Iyx5,Iyx6,Iyy4,Iyy5,Iyy6,Iyz3,Iyz4,Iyz5,Iyz6,Izx2,Izx3,Izx4,Izx5,Izx6,Izy3,Izy4,Izy5,Izy6,Izz2,Izz3,Izz4,Izz5,Izz6,Lx2,Lx3,Lxcm2,Lxcm3,Lxcm4,Lxcm5,Lxcm6,Lycm3,Lycm4,Lycm5,Lycm6,Lz4,Lz5,Lzcm2,Lzcm3,Lzcm4,Lzcm5,Lzcm6,dQ1,dQ2,dQ3,dQ4,dQ5,dQ6,m2,m3,m4,m5,m6,t10,t1000,t1031,t1032,t1033,t1034,t1035,t1036,t1037,t1038,t1039,t1040,t1041,t1042,t1043,t1044,t1045,t1046,t1047,t1048,t1049,t1050,t1051,t1052,t1053,t1054,t1055,t1056,t1057,t1058,t1059,t1060,t11,t12,t126,t127,t128,t129,t13,t130,t131,t132,t133,t134,t135,t136,t137,t138,t139,t14,t140,t141,t142,t143,t144,t145,t146,t147,t148,t149,t15,t150,t151,t152,t153,t154,t155,t156,t157,t16,t166,t167,t168,t169,t17,t170,t171,t172,t173,t174,t175,t176,t177,t178,t179,t18,t180,t181,t182,t183,t184,t185,t186,t187,t188,t189,t19,t190,t191,t192,t193,t194,t195,t196,t2,t20,t21,t22,t221,t222,t223,t224,t225,t226,t23,t237,t238,t239,t24,t240,t241,t242,t243,t244,t245,t246,t247,t248,t249,t25,t250,t251,t252,t253,t254,t255,t256,t257,t258,t259,t26,t260,t261,t262,t263,t264,t265,t266,t267,t268,t269,t270,t271,t272,t273,t274,t275,t276,t277,t278,t279,t280,t281,t282,t283,t284,t285,t286,t287,t288,t289,t290,t291,t292,t293,t294,t295,t296,t297,t298,t3,t32,t33,t34,t35,t36,t37,t38,t39,t399,t4,t40,t400,t401,t402,t403,t404,t405,t406,t407,t408,t409,t41,t410,t411,t412,t413,t414,t415,t416,t417,t418,t419,t42,t420,t421,t422,t423,t424,t425,t426,t427,t428,t429,t43,t430,t431,t432,t433,t434,t435,t436,t437,t438,t439,t44,t440,t441,t442,t443,t444,t445,t446,t447,t448,t449,t45,t450,t451,t452,t453,t454,t455,t456,t457,t458,t459,t46,t460,t47,t48,t485,t486,t49,t498,t499,t5,t50,t500,t501,t502,t503,t504,t505,t506,t507,t508,t509,t51,t510,t511,t512,t513,t514,t515,t516,t517,t518,t519,t52,t520,t521,t522,t523,t524,t525,t526,t527,t528,t529,t53,t530,t531,t532,t533,t534,t535,t536,t537,t538,t539,t54,t540,t541,t542,t543,t544,t545,t546,t547,t548,t549,t55,t550,t551,t552,t553,t56,t57,t58,t59,t6,t60,t61,t615,t616,t617,t618,t619,t62,t620,t621,t622,t63,t64,t644,t645,t646,t647,t648,t649,t65,t650,t651,t652,t653,t654,t655,t656,t657,t658,t659,t66,t660,t661,t662,t663,t664,t665,t666,t667,t668,t669,t67,t670,t671,t672,t673,t674,t675,t676,t677,t678,t679,t68,t680,t681,t682,t683,t684,t685,t686,t687,t688,t689,t69,t690,t691,t692,t693,t694,t695,t696,t697,t7,t70,t71,t712,t713,t714,t715,t716,t717,t718,t719,t72,t720,t721,t722,t723,t724,t725,t726,t727,t728,t729,t73,t730,t731,t732,t733,t734,t735,t736,t737,t738,t739,t74,t740,t741,t742,t743,t744,t75,t76,t77,t78,t79,t8,t80,t81,t831,t832,t833,t834,t839,t840,t841,t842,t843,t844,t845,t846,t847,t848,t856,t857,t858,t859,t860,t861,t862,t863,t864,t865,t866,t867,t9,t937,t938,t939,t940,t941,t942,t943,t944,t945,t946,t947,t948,t949,t950,t962,t963,t999] = ct{:};
t1061 = Ixy6.*dQ1.*dQ4.*t3.*t4.*t5.*t7.*t9.*2.0;
t1062 = Ixy6.*dQ1.*dQ5.*t2.*t3.*t6.*t9.*t11.*2.0;
t1063 = Ixy6.*dQ1.*dQ6.*t2.*t5.*t6.*t8.*t11.*2.0;
t1064 = Ixy6.*dQ1.*dQ6.*t3.*t5.*t6.*t7.*t11.*2.0;
t1065 = Ixy6.*dQ2.*dQ6.*t4.*t5.*t6.*t9.*t11.*4.0;
t1066 = Ixy6.*dQ3.*dQ6.*t4.*t5.*t6.*t9.*t11.*4.0;
t1067 = Ixz5.*dQ1.*dQ5.*t2.*t3.*t5.*t9.*t10.*2.0;
t1068 = Ixz6.*dQ2.*dQ4.*t4.*t5.*t6.*t9.*t10.*2.0;
t1069 = Ixz6.*dQ3.*dQ4.*t4.*t5.*t6.*t9.*t10.*2.0;
t1070 = Iyx5.*dQ1.*dQ4.*t2.*t4.*t5.*t8.*t9.*2.0;
t1071 = Iyx5.*dQ1.*dQ4.*t3.*t4.*t5.*t7.*t9.*2.0;
t1072 = Iyx6.*dQ1.*dQ4.*t2.*t4.*t5.*t8.*t9.*2.0;
t1073 = Iyx6.*dQ1.*dQ4.*t3.*t4.*t5.*t7.*t9.*2.0;
t1074 = Iyx6.*dQ1.*dQ5.*t2.*t3.*t6.*t9.*t11.*2.0;
t1075 = Iyx6.*dQ1.*dQ6.*t2.*t5.*t6.*t8.*t11.*2.0;
t1076 = Iyx6.*dQ1.*dQ6.*t3.*t5.*t6.*t7.*t11.*2.0;
t1077 = Iyx6.*dQ2.*dQ6.*t4.*t5.*t6.*t9.*t11.*4.0;
t1078 = Iyx6.*dQ3.*dQ6.*t4.*t5.*t6.*t9.*t11.*4.0;
t1079 = Izx5.*dQ1.*dQ5.*t2.*t3.*t5.*t9.*t10.*2.0;
t1080 = Izx6.*dQ2.*dQ4.*t4.*t5.*t6.*t9.*t10.*2.0;
t1081 = Izx6.*dQ3.*dQ4.*t4.*t5.*t6.*t9.*t10.*2.0;
t1086 = Lx3.*Lycm6.*dQ1.*dQ4.*m6.*t2.*t6.*t8.*t9.*2.0;
t1087 = Lx3.*Lycm6.*dQ1.*dQ4.*m6.*t3.*t6.*t7.*t9.*2.0;
t1088 = Lx3.*Lycm6.*dQ1.*dQ6.*m6.*t2.*t4.*t8.*t11.*2.0;
t1089 = Lx3.*Lycm6.*dQ1.*dQ6.*m6.*t3.*t4.*t7.*t11.*2.0;
t1090 = Lxcm4.*Lycm4.*dQ1.*dQ4.*m4.*t2.*t4.*t8.*t9.*4.0;
t1091 = Lxcm4.*Lycm4.*dQ1.*dQ4.*m4.*t3.*t4.*t7.*t9.*4.0;
t1092 = Lxcm5.*Lycm5.*dQ1.*dQ4.*m5.*t2.*t3.*t9.*t10.*2.0;
t1093 = Lxcm6.*Lycm6.*dQ1.*dQ4.*m6.*t2.*t3.*t9.*t10.*2.0;
t1094 = Lxcm6.*Lycm6.*dQ1.*dQ6.*m6.*t2.*t4.*t8.*t9.*2.0;
t1095 = Lxcm6.*Lycm6.*dQ1.*dQ6.*m6.*t3.*t4.*t7.*t9.*2.0;
t1096 = Lxcm6.*Lycm6.*dQ1.*dQ4.*m6.*t2.*t6.*t8.*t11.*4.0;
t1097 = Lxcm6.*Lycm6.*dQ1.*dQ4.*m6.*t3.*t6.*t7.*t11.*4.0;
t1098 = Lxcm6.*Lycm6.*dQ2.*dQ4.*m6.*t4.*t6.*t9.*t11.*4.0;
t1099 = Lxcm6.*Lycm6.*dQ3.*dQ4.*m6.*t4.*t6.*t9.*t11.*4.0;
t1100 = Lxcm6.*Lycm6.*dQ2.*dQ5.*m6.*t5.*t6.*t10.*t11.*4.0;
t1101 = Lxcm6.*Lycm6.*dQ3.*dQ5.*m6.*t5.*t6.*t10.*t11.*4.0;
t1102 = Lxcm6.*Lycm6.*dQ4.*dQ6.*m6.*t4.*t6.*t10.*t11.*4.0;
t1103 = Lxcm6.*Lycm6.*dQ5.*dQ6.*m6.*t5.*t6.*t9.*t11.*4.0;
t1104 = Lx3.*Lz5.*dQ1.*dQ4.*m6.*t2.*t4.*t8.*t10.*2.0;
t1105 = Lx3.*Lz5.*dQ1.*dQ4.*m6.*t3.*t4.*t7.*t10.*2.0;
t1106 = Lx3.*Lz5.*dQ1.*dQ5.*m6.*t2.*t5.*t8.*t9.*2.0;
t1107 = Lx3.*Lz5.*dQ1.*dQ5.*m6.*t3.*t5.*t7.*t9.*2.0;
t1108 = Lx3.*Lzcm5.*dQ1.*dQ4.*m5.*t2.*t4.*t8.*t10.*2.0;
t1109 = Lx3.*Lzcm5.*dQ1.*dQ4.*m5.*t3.*t4.*t7.*t10.*2.0;
t1110 = Lx3.*Lzcm5.*dQ1.*dQ5.*m5.*t2.*t5.*t8.*t9.*2.0;
t1111 = Lx3.*Lzcm5.*dQ1.*dQ5.*m5.*t3.*t5.*t7.*t9.*2.0;
t1112 = Lxcm5.*Lz4.*dQ1.*dQ4.*m5.*t4.*t5.*t7.*t8.*2.0;
t1113 = Lx3.*Lzcm6.*dQ1.*dQ4.*m6.*t2.*t4.*t8.*t10.*2.0;
t1114 = Lx3.*Lzcm6.*dQ1.*dQ4.*m6.*t3.*t4.*t7.*t10.*2.0;
t1115 = Lxcm5.*Lz4.*dQ1.*dQ5.*m5.*t2.*t3.*t9.*t10.*2.0;
t1116 = Lx3.*Lzcm6.*dQ1.*dQ5.*m6.*t2.*t5.*t8.*t9.*2.0;
t1117 = Lx3.*Lzcm6.*dQ1.*dQ5.*m6.*t3.*t5.*t7.*t9.*2.0;
t1118 = Lxcm6.*Lz4.*dQ1.*dQ4.*m6.*t2.*t3.*t9.*t11.*2.0;
t1119 = Lxcm6.*Lz5.*dQ1.*dQ4.*m6.*t4.*t6.*t7.*t8.*2.0;
t1120 = Lxcm6.*Lz4.*dQ1.*dQ6.*m6.*t4.*t6.*t7.*t8.*2.0;
t1121 = Lxcm6.*Lz5.*dQ1.*dQ5.*m6.*t2.*t5.*t8.*t11.*2.0;
t1122 = Lxcm6.*Lz5.*dQ1.*dQ5.*m6.*t3.*t5.*t7.*t11.*2.0;
t1123 = Lxcm6.*Lz5.*dQ2.*dQ5.*m6.*t4.*t5.*t9.*t11.*2.0;
t1124 = Lxcm6.*Lz5.*dQ2.*dQ6.*m6.*t4.*t6.*t9.*t10.*2.0;
t1125 = Lxcm6.*Lz5.*dQ3.*dQ5.*m6.*t4.*t5.*t9.*t11.*2.0;
t1126 = Lxcm6.*Lz5.*dQ3.*dQ6.*m6.*t4.*t6.*t9.*t10.*2.0;
t1127 = Lxcm6.*Lz5.*dQ4.*dQ5.*m6.*t5.*t6.*t9.*t10.*4.0;
t1128 = Lxcm5.*Lzcm5.*dQ1.*dQ5.*m5.*t2.*t4.*t8.*t9.*2.0;
t1129 = Lxcm5.*Lzcm5.*dQ1.*dQ5.*m5.*t3.*t4.*t7.*t9.*2.0;
t1130 = Lxcm6.*Lzcm6.*dQ1.*dQ4.*m6.*t4.*t6.*t7.*t8.*2.0;
t1131 = Lxcm6.*Lzcm6.*dQ1.*dQ5.*m6.*t2.*t5.*t8.*t11.*2.0;
t1132 = Lxcm6.*Lzcm6.*dQ1.*dQ5.*m6.*t3.*t5.*t7.*t11.*2.0;
t1133 = Lxcm5.*Lzcm5.*dQ2.*dQ4.*m5.*t4.*t5.*t9.*t10.*4.0;
t1134 = Lxcm5.*Lzcm5.*dQ3.*dQ4.*m5.*t4.*t5.*t9.*t10.*4.0;
t1135 = Lxcm6.*Lzcm6.*dQ2.*dQ5.*m6.*t4.*t5.*t9.*t11.*2.0;
t1136 = Lxcm6.*Lzcm6.*dQ2.*dQ6.*m6.*t4.*t6.*t9.*t10.*2.0;
t1137 = Lxcm6.*Lzcm6.*dQ3.*dQ5.*m6.*t4.*t5.*t9.*t11.*2.0;
t1138 = Lxcm6.*Lzcm6.*dQ3.*dQ6.*m6.*t4.*t6.*t9.*t10.*2.0;
t1139 = Lxcm6.*Lzcm6.*dQ4.*dQ5.*m6.*t5.*t6.*t9.*t10.*4.0;
t1140 = Ixx5.*dQ1.*dQ4.*t4.*t5.*t7.*t8.*t10.*2.0;
t1141 = Ixx6.*dQ1.*dQ5.*t2.*t6.*t8.*t10.*t11.*2.0;
t1142 = Ixx6.*dQ1.*dQ5.*t3.*t6.*t7.*t10.*t11.*2.0;
t1143 = Ixx6.*dQ2.*dQ5.*t4.*t6.*t9.*t10.*t11.*2.0;
t1144 = Ixx6.*dQ3.*dQ5.*t4.*t6.*t9.*t10.*t11.*2.0;
t1145 = Ixx6.*dQ4.*dQ6.*t5.*t6.*t9.*t10.*t11.*2.0;
t1146 = Iyy6.*dQ1.*dQ4.*t4.*t5.*t7.*t8.*t10.*2.0;
t1147 = Iyy6.*dQ1.*dQ5.*t2.*t6.*t8.*t10.*t11.*2.0;
t1148 = Iyy6.*dQ1.*dQ5.*t3.*t6.*t7.*t10.*t11.*2.0;
t1149 = Iyy6.*dQ2.*dQ5.*t4.*t6.*t9.*t10.*t11.*2.0;
t1150 = Iyy6.*dQ3.*dQ5.*t4.*t6.*t9.*t10.*t11.*2.0;
t1151 = Iyy6.*dQ4.*dQ6.*t5.*t6.*t9.*t10.*t11.*2.0;
t1152 = Iyz5.*dQ1.*dQ4.*t2.*t4.*t8.*t9.*t10.*2.0;
t1153 = Iyz5.*dQ1.*dQ4.*t3.*t4.*t7.*t9.*t10.*2.0;
t1154 = Iyz6.*dQ2.*dQ4.*t4.*t5.*t9.*t10.*t11.*2.0;
t1155 = Iyz6.*dQ3.*dQ4.*t4.*t5.*t9.*t10.*t11.*2.0;
t1156 = Izy5.*dQ1.*dQ4.*t2.*t4.*t8.*t9.*t10.*2.0;
t1157 = Izy5.*dQ1.*dQ4.*t3.*t4.*t7.*t9.*t10.*2.0;
t1158 = Izy6.*dQ2.*dQ4.*t4.*t5.*t9.*t10.*t11.*2.0;
t1159 = Izy6.*dQ3.*dQ4.*t4.*t5.*t9.*t10.*t11.*2.0;
t1160 = Izz5.*dQ1.*dQ4.*t4.*t5.*t7.*t8.*t10.*2.0;
t1161 = Izz6.*dQ1.*dQ4.*t4.*t5.*t7.*t8.*t10.*2.0;
t1162 = Lx3.*Lxcm5.*dQ1.*dQ5.*m5.*t2.*t8.*t9.*t10.*2.0;
t1163 = Lx3.*Lxcm5.*dQ1.*dQ5.*m5.*t3.*t7.*t9.*t10.*2.0;
t1164 = Lx3.*Lxcm6.*dQ1.*dQ4.*m6.*t2.*t8.*t9.*t11.*2.0;
t1165 = Lx3.*Lxcm6.*dQ1.*dQ4.*m6.*t3.*t7.*t9.*t11.*2.0;
t1166 = Lycm6.*Lz4.*dQ1.*dQ4.*m6.*t6.*t7.*t8.*t9.*2.0;
t1167 = Lycm6.*Lz5.*dQ1.*dQ4.*m6.*t4.*t7.*t8.*t11.*2.0;
t1168 = Lycm6.*Lz4.*dQ1.*dQ6.*m6.*t4.*t7.*t8.*t11.*2.0;
t1169 = Lycm6.*Lz5.*dQ2.*dQ6.*m6.*t4.*t9.*t10.*t11.*2.0;
t1170 = Lycm6.*Lz5.*dQ3.*dQ6.*m6.*t4.*t9.*t10.*t11.*2.0;
t1171 = Lycm6.*Lz5.*dQ4.*dQ5.*m6.*t5.*t9.*t10.*t11.*4.0;
t1172 = Lycm5.*Lzcm5.*dQ1.*dQ4.*m5.*t5.*t7.*t8.*t9.*2.0;
t1173 = Lycm6.*Lzcm6.*dQ1.*dQ4.*m6.*t4.*t7.*t8.*t11.*2.0;
t1174 = Lycm6.*Lzcm6.*dQ2.*dQ6.*m6.*t4.*t9.*t10.*t11.*2.0;
t1175 = Lycm6.*Lzcm6.*dQ3.*dQ6.*m6.*t4.*t9.*t10.*t11.*2.0;
t1176 = Lycm6.*Lzcm6.*dQ4.*dQ5.*m6.*t5.*t9.*t10.*t11.*4.0;
t1177 = Lz4.*Lz5.*dQ1.*dQ4.*m6.*t4.*t7.*t8.*t10.*2.0;
t1178 = Lz4.*Lz5.*dQ1.*dQ5.*m6.*t5.*t7.*t8.*t9.*2.0;
t1179 = Lz4.*Lzcm5.*dQ1.*dQ4.*m5.*t4.*t7.*t8.*t10.*2.0;
t1180 = Lz4.*Lzcm5.*dQ1.*dQ5.*m5.*t5.*t7.*t8.*t9.*2.0;
t1181 = Lz4.*Lzcm6.*dQ1.*dQ4.*m6.*t4.*t7.*t8.*t10.*2.0;
t1182 = Lz4.*Lzcm6.*dQ1.*dQ5.*m6.*t5.*t7.*t8.*t9.*2.0;
t1183 = Ixy6.*dQ1.*dQ5.*t6.*t7.*t8.*t9.*t11.*2.0;
t1184 = Ixz5.*dQ1.*dQ5.*t5.*t7.*t8.*t9.*t10.*2.0;
t1185 = Iyx6.*dQ1.*dQ5.*t6.*t7.*t8.*t9.*t11.*2.0;
t1186 = Izx5.*dQ1.*dQ5.*t5.*t7.*t8.*t9.*t10.*2.0;
t1187 = Lxcm5.*Lycm5.*dQ1.*dQ4.*m5.*t7.*t8.*t9.*t10.*2.0;
t1188 = Lxcm6.*Lycm6.*dQ1.*dQ4.*m6.*t7.*t8.*t9.*t10.*2.0;
t1189 = Lxcm5.*Lz4.*dQ1.*dQ5.*m5.*t7.*t8.*t9.*t10.*2.0;
t1190 = Lxcm6.*Lz4.*dQ1.*dQ4.*m6.*t7.*t8.*t9.*t11.*2.0;
t1282 = Lxcm5.*Lz4.*dQ1.*dQ4.*m5.*t2.*t3.*t4.*t5.*2.0;
t1283 = Lxcm6.*Lz5.*dQ1.*dQ4.*m6.*t2.*t3.*t4.*t6.*2.0;
t1284 = Lxcm6.*Lz4.*dQ1.*dQ6.*m6.*t2.*t3.*t4.*t6.*2.0;
t1285 = Lxcm6.*Lzcm6.*dQ1.*dQ4.*m6.*t2.*t3.*t4.*t6.*2.0;
t1344 = dQ1.*dQ6.*m6.*t2.*t3.*t4.*t10.*t20.*2.0;
t1380 = dQ1.*dQ6.*m6.*t4.*t7.*t8.*t10.*t20.*2.0;
t1522 = Lycm6.*Lz4.*dQ1.*dQ5.*m6.*t7.*t8.*t9.*t10.*t11.*2.0;
t1624 = Lxcm6.*Lz4.*dQ1.*dQ4.*m6.*t2.*t3.*t4.*t5.*t6.*2.0;
t1625 = Lxcm6.*Lz5.*dQ1.*dQ6.*m6.*t2.*t3.*t4.*t5.*t6.*2.0;
t1626 = Lxcm6.*Lzcm6.*dQ1.*dQ6.*m6.*t2.*t3.*t4.*t5.*t6.*2.0;
t1627 = Lx3.*Lxcm6.*dQ1.*dQ4.*m6.*t2.*t4.*t5.*t6.*t8.*2.0;
t1628 = Lx3.*Lxcm6.*dQ1.*dQ4.*m6.*t3.*t4.*t5.*t6.*t7.*2.0;
t1629 = Lycm6.*Lz4.*dQ1.*dQ4.*m6.*t2.*t3.*t4.*t5.*t11.*2.0;
t1630 = Lycm6.*Lz5.*dQ1.*dQ4.*m6.*t2.*t3.*t5.*t6.*t9.*2.0;
t1631 = Lycm6.*Lz4.*dQ1.*dQ6.*m6.*t2.*t3.*t5.*t6.*t9.*2.0;
t1632 = Lycm6.*Lz5.*dQ1.*dQ6.*m6.*t2.*t3.*t4.*t5.*t11.*2.0;
t1633 = Lycm6.*Lzcm6.*dQ1.*dQ4.*m6.*t2.*t3.*t5.*t6.*t9.*2.0;
t1634 = Lycm6.*Lzcm6.*dQ1.*dQ6.*m6.*t2.*t3.*t4.*t5.*t11.*2.0;
t1635 = Lz5.*Lzcm6.*dQ1.*dQ4.*m6.*t2.*t3.*t4.*t5.*t10.*4.0;
t1636 = Ixy6.*dQ1.*dQ6.*t2.*t3.*t4.*t6.*t10.*t11.*2.0;
t1637 = Ixz6.*dQ1.*dQ5.*t2.*t3.*t5.*t6.*t9.*t10.*2.0;
t1638 = Iyx6.*dQ1.*dQ6.*t2.*t3.*t4.*t6.*t10.*t11.*2.0;
t1639 = Izx6.*dQ1.*dQ5.*t2.*t3.*t5.*t6.*t9.*t10.*2.0;
t1666 = Lx3.*Lycm6.*dQ1.*dQ4.*m6.*t2.*t4.*t5.*t8.*t11.*2.0;
t1667 = Lx3.*Lycm6.*dQ1.*dQ4.*m6.*t3.*t4.*t5.*t7.*t11.*2.0;
t1668 = Lx3.*Lycm6.*dQ1.*dQ6.*m6.*t2.*t5.*t6.*t8.*t9.*2.0;
t1669 = Lx3.*Lycm6.*dQ1.*dQ6.*m6.*t3.*t5.*t6.*t7.*t9.*2.0;
t1670 = Lxcm5.*Lycm5.*dQ1.*dQ4.*m5.*t2.*t4.*t5.*t8.*t9.*4.0;
t1671 = Lxcm5.*Lycm5.*dQ1.*dQ4.*m5.*t3.*t4.*t5.*t7.*t9.*4.0;
t1672 = Lxcm6.*Lycm6.*dQ1.*dQ4.*m6.*t2.*t4.*t5.*t8.*t9.*4.0;
t1673 = Lxcm6.*Lycm6.*dQ1.*dQ4.*m6.*t3.*t4.*t5.*t7.*t9.*4.0;
t1674 = Lxcm6.*Lycm6.*dQ1.*dQ6.*m6.*t2.*t3.*t5.*t9.*t10.*2.0;
t1675 = Lxcm6.*Lycm6.*dQ1.*dQ5.*m6.*t2.*t3.*t6.*t9.*t11.*4.0;
t1676 = Lxcm6.*Lycm6.*dQ1.*dQ6.*m6.*t2.*t5.*t6.*t8.*t11.*4.0;
t1677 = Lxcm6.*Lycm6.*dQ1.*dQ6.*m6.*t3.*t5.*t6.*t7.*t11.*4.0;
t1678 = Lxcm6.*Lz4.*dQ1.*dQ4.*m6.*t4.*t5.*t6.*t7.*t8.*2.0;
t1679 = Lxcm6.*Lz4.*dQ1.*dQ5.*m6.*t2.*t3.*t6.*t9.*t10.*2.0;
t1680 = Lxcm6.*Lz5.*dQ1.*dQ4.*m6.*t2.*t3.*t5.*t9.*t11.*2.0;
t1681 = Lxcm6.*Lz5.*dQ1.*dQ5.*m6.*t2.*t4.*t6.*t8.*t9.*2.0;
t1682 = Lxcm6.*Lz5.*dQ1.*dQ5.*m6.*t3.*t4.*t6.*t7.*t9.*2.0;
t1683 = Lxcm6.*Lz4.*dQ1.*dQ6.*m6.*t2.*t3.*t5.*t9.*t11.*2.0;
t1684 = Lxcm6.*Lz5.*dQ1.*dQ6.*m6.*t4.*t5.*t6.*t7.*t8.*2.0;
t1685 = Lxcm6.*Lz5.*dQ2.*dQ4.*m6.*t4.*t5.*t6.*t9.*t10.*4.0;
t1686 = Lxcm6.*Lz5.*dQ3.*dQ4.*m6.*t4.*t5.*t6.*t9.*t10.*4.0;
t1687 = Lxcm5.*Lzcm5.*dQ1.*dQ5.*m5.*t2.*t3.*t5.*t9.*t10.*4.0;
t1688 = Lxcm6.*Lzcm6.*dQ1.*dQ4.*m6.*t2.*t3.*t5.*t9.*t11.*2.0;
t1689 = Lxcm6.*Lzcm6.*dQ1.*dQ5.*m6.*t2.*t4.*t6.*t8.*t9.*2.0;
t1690 = Lxcm6.*Lzcm6.*dQ1.*dQ5.*m6.*t3.*t4.*t6.*t7.*t9.*2.0;
t1691 = Lxcm6.*Lzcm6.*dQ1.*dQ6.*m6.*t4.*t5.*t6.*t7.*t8.*2.0;
t1692 = Lxcm6.*Lzcm6.*dQ2.*dQ4.*m6.*t4.*t5.*t6.*t9.*t10.*4.0;
t1693 = Lxcm6.*Lzcm6.*dQ3.*dQ4.*m6.*t4.*t5.*t6.*t9.*t10.*4.0;
t1694 = Ixx5.*dQ1.*dQ5.*t2.*t4.*t5.*t8.*t9.*t10.*2.0;
t1695 = Ixx5.*dQ1.*dQ5.*t3.*t4.*t5.*t7.*t9.*t10.*2.0;
t1696 = Ixx6.*dQ1.*dQ4.*t2.*t3.*t6.*t9.*t10.*t11.*2.0;
t1697 = Ixx6.*dQ1.*dQ6.*t2.*t4.*t6.*t8.*t9.*t11.*2.0;
t1698 = Ixx6.*dQ1.*dQ6.*t3.*t4.*t6.*t7.*t9.*t11.*2.0;
t1699 = Iyy6.*dQ1.*dQ5.*t2.*t4.*t5.*t8.*t9.*t10.*2.0;
t1700 = Iyy6.*dQ1.*dQ5.*t3.*t4.*t5.*t7.*t9.*t10.*2.0;
t1701 = Iyy6.*dQ1.*dQ4.*t2.*t3.*t6.*t9.*t10.*t11.*2.0;
t1702 = Iyy6.*dQ1.*dQ6.*t2.*t4.*t6.*t8.*t9.*t11.*2.0;
t1703 = Iyy6.*dQ1.*dQ6.*t3.*t4.*t6.*t7.*t9.*t11.*2.0;
t1704 = Iyz6.*dQ1.*dQ4.*t2.*t4.*t6.*t8.*t9.*t10.*2.0;
t1705 = Iyz6.*dQ1.*dQ4.*t3.*t4.*t6.*t7.*t9.*t10.*2.0;
t1706 = Iyz6.*dQ1.*dQ5.*t2.*t3.*t5.*t9.*t10.*t11.*2.0;
t1707 = Izy6.*dQ1.*dQ4.*t2.*t4.*t6.*t8.*t9.*t10.*2.0;
t1708 = Izy6.*dQ1.*dQ4.*t3.*t4.*t6.*t7.*t9.*t10.*2.0;
t1709 = Izy6.*dQ1.*dQ5.*t2.*t3.*t5.*t9.*t10.*t11.*2.0;
t1710 = Izz5.*dQ1.*dQ5.*t2.*t4.*t5.*t8.*t9.*t10.*2.0;
t1711 = Izz5.*dQ1.*dQ5.*t3.*t4.*t5.*t7.*t9.*t10.*2.0;
t1712 = Izz6.*dQ1.*dQ5.*t2.*t4.*t5.*t8.*t9.*t10.*2.0;
t1713 = Izz6.*dQ1.*dQ5.*t3.*t4.*t5.*t7.*t9.*t10.*2.0;
t1714 = Lx3.*Lxcm6.*dQ1.*dQ5.*m6.*t2.*t6.*t8.*t9.*t10.*2.0;
t1715 = Lx3.*Lxcm6.*dQ1.*dQ5.*m6.*t3.*t6.*t7.*t9.*t10.*2.0;
t1716 = Lx3.*Lxcm6.*dQ1.*dQ6.*m6.*t2.*t5.*t8.*t9.*t11.*2.0;
t1717 = Lx3.*Lxcm6.*dQ1.*dQ6.*m6.*t3.*t5.*t7.*t9.*t11.*2.0;
t1718 = Lycm6.*Lz4.*dQ1.*dQ4.*m6.*t4.*t5.*t7.*t8.*t11.*2.0;
t1719 = Lycm6.*Lz4.*dQ1.*dQ5.*m6.*t2.*t3.*t9.*t10.*t11.*2.0;
t1720 = Lycm6.*Lz5.*dQ1.*dQ4.*m6.*t5.*t6.*t7.*t8.*t9.*2.0;
t1721 = Lycm6.*Lz5.*dQ1.*dQ5.*m6.*t2.*t4.*t8.*t9.*t11.*2.0;
t1722 = Lycm6.*Lz5.*dQ1.*dQ5.*m6.*t3.*t4.*t7.*t9.*t11.*2.0;
t1723 = Lycm6.*Lz4.*dQ1.*dQ6.*m6.*t5.*t6.*t7.*t8.*t9.*2.0;
t1724 = Lycm6.*Lz5.*dQ1.*dQ6.*m6.*t4.*t5.*t7.*t8.*t11.*2.0;
t1725 = Lycm6.*Lz5.*dQ2.*dQ4.*m6.*t4.*t5.*t9.*t10.*t11.*4.0;
t1726 = Lycm6.*Lz5.*dQ3.*dQ4.*m6.*t4.*t5.*t9.*t10.*t11.*4.0;
t1727 = Lycm5.*Lzcm5.*dQ1.*dQ4.*m5.*t2.*t4.*t8.*t9.*t10.*4.0;
t1728 = Lycm5.*Lzcm5.*dQ1.*dQ4.*m5.*t3.*t4.*t7.*t9.*t10.*4.0;
t1729 = Lycm6.*Lzcm6.*dQ1.*dQ4.*m6.*t5.*t6.*t7.*t8.*t9.*2.0;
t1730 = Lycm6.*Lzcm6.*dQ1.*dQ5.*m6.*t2.*t4.*t8.*t9.*t11.*2.0;
t1731 = Lycm6.*Lzcm6.*dQ1.*dQ5.*m6.*t3.*t4.*t7.*t9.*t11.*2.0;
t1732 = Lycm6.*Lzcm6.*dQ1.*dQ6.*m6.*t4.*t5.*t7.*t8.*t11.*2.0;
t1733 = Lycm6.*Lzcm6.*dQ2.*dQ4.*m6.*t4.*t5.*t9.*t10.*t11.*4.0;
t1734 = Lycm6.*Lzcm6.*dQ3.*dQ4.*m6.*t4.*t5.*t9.*t10.*t11.*4.0;
t1735 = Lz5.*Lzcm6.*dQ1.*dQ4.*m6.*t4.*t5.*t7.*t8.*t10.*4.0;
t1736 = Ixy6.*dQ1.*dQ6.*t4.*t6.*t7.*t8.*t10.*t11.*2.0;
t1737 = Ixz6.*dQ1.*dQ4.*t2.*t4.*t8.*t9.*t10.*t11.*2.0;
t1738 = Ixz6.*dQ1.*dQ4.*t3.*t4.*t7.*t9.*t10.*t11.*2.0;
t1739 = Ixz6.*dQ1.*dQ5.*t5.*t6.*t7.*t8.*t9.*t10.*2.0;
t1740 = Iyx6.*dQ1.*dQ6.*t4.*t6.*t7.*t8.*t10.*t11.*2.0;
t1741 = Izx6.*dQ1.*dQ4.*t2.*t4.*t8.*t9.*t10.*t11.*2.0;
t1742 = Izx6.*dQ1.*dQ4.*t3.*t4.*t7.*t9.*t10.*t11.*2.0;
t1743 = Izx6.*dQ1.*dQ5.*t5.*t6.*t7.*t8.*t9.*t10.*2.0;
t1744 = Lx3.*Lycm6.*dQ1.*dQ5.*m6.*t2.*t8.*t9.*t10.*t11.*2.0;
t1745 = Lx3.*Lycm6.*dQ1.*dQ5.*m6.*t3.*t7.*t9.*t10.*t11.*2.0;
t1746 = Lxcm6.*Lycm6.*dQ1.*dQ6.*m6.*t5.*t7.*t8.*t9.*t10.*2.0;
t1747 = Lxcm6.*Lycm6.*dQ1.*dQ5.*m6.*t6.*t7.*t8.*t9.*t11.*4.0;
t1748 = Lxcm6.*Lz4.*dQ1.*dQ5.*m6.*t6.*t7.*t8.*t9.*t10.*2.0;
t1749 = Lxcm6.*Lz5.*dQ1.*dQ4.*m6.*t5.*t7.*t8.*t9.*t11.*2.0;
t1750 = Lxcm6.*Lz4.*dQ1.*dQ6.*m6.*t5.*t7.*t8.*t9.*t11.*2.0;
t1751 = Lxcm5.*Lzcm5.*dQ1.*dQ5.*m5.*t5.*t7.*t8.*t9.*t10.*4.0;
t1752 = Lxcm6.*Lzcm6.*dQ1.*dQ4.*m6.*t5.*t7.*t8.*t9.*t11.*2.0;
t1753 = Ixx6.*dQ1.*dQ4.*t6.*t7.*t8.*t9.*t10.*t11.*2.0;
t1754 = Iyy6.*dQ1.*dQ4.*t6.*t7.*t8.*t9.*t10.*t11.*2.0;
t1755 = Iyz6.*dQ1.*dQ5.*t5.*t7.*t8.*t9.*t10.*t11.*2.0;
t1756 = Izy6.*dQ1.*dQ5.*t5.*t7.*t8.*t9.*t10.*t11.*2.0;
t1836 = Iyz6.*dQ1.*dQ6.*t2.*t4.*t5.*t6.*t8.*t9.*t10;
t1837 = Iyz6.*dQ1.*dQ6.*t3.*t4.*t5.*t6.*t7.*t9.*t10;
t1838 = Izy6.*dQ1.*dQ6.*t2.*t4.*t5.*t6.*t8.*t9.*t10;
t1839 = Izy6.*dQ1.*dQ6.*t3.*t4.*t5.*t6.*t7.*t9.*t10;
t1842 = Ixz6.*dQ1.*dQ6.*t2.*t4.*t5.*t8.*t9.*t10.*t11;
t1843 = Ixz6.*dQ1.*dQ6.*t3.*t4.*t5.*t7.*t9.*t10.*t11;
t1844 = Izx6.*dQ1.*dQ6.*t2.*t4.*t5.*t8.*t9.*t10.*t11;
t1845 = Izx6.*dQ1.*dQ6.*t3.*t4.*t5.*t7.*t9.*t10.*t11;
t1869 = Lxcm6.*Lycm6.*dQ2.*dQ6.*m6.*t4.*t5.*t6.*t9.*t11.*8.0;
t1870 = Lxcm6.*Lycm6.*dQ3.*dQ6.*m6.*t4.*t5.*t6.*t9.*t11.*8.0;
t1879 = dQ1.*dQ4.*m5.*t2.*t3.*t4.*t5.*t10.*t16.*2.0;
t1880 = dQ1.*dQ4.*m6.*t2.*t3.*t4.*t5.*t10.*t20.*2.0;
t1881 = dQ1.*dQ4.*m6.*t2.*t3.*t4.*t5.*t10.*t22.*2.0;
t1882 = dQ1.*dQ4.*m5.*t2.*t3.*t4.*t5.*t10.*t25.*2.0;
t1883 = dQ1.*dQ4.*m6.*t2.*t3.*t4.*t5.*t10.*t26.*2.0;
t1923 = dQ1.*dQ4.*m5.*t4.*t5.*t7.*t8.*t10.*t16.*2.0;
t1924 = dQ1.*dQ5.*m6.*t2.*t6.*t8.*t10.*t11.*t17.*2.0;
t1925 = dQ1.*dQ5.*m6.*t3.*t6.*t7.*t10.*t11.*t17.*2.0;
t1926 = dQ2.*dQ5.*m6.*t4.*t6.*t9.*t10.*t11.*t17.*2.0;
t1927 = dQ3.*dQ5.*m6.*t4.*t6.*t9.*t10.*t11.*t17.*2.0;
t1928 = dQ4.*dQ6.*m6.*t5.*t6.*t9.*t10.*t11.*t17.*2.0;
t1929 = dQ1.*dQ4.*m6.*t4.*t5.*t7.*t8.*t10.*t20.*2.0;
t1930 = dQ1.*dQ5.*m6.*t2.*t6.*t8.*t10.*t11.*t20.*2.0;
t1931 = dQ1.*dQ5.*m6.*t3.*t6.*t7.*t10.*t11.*t20.*2.0;
t1932 = dQ2.*dQ5.*m6.*t4.*t6.*t9.*t10.*t11.*t20.*2.0;
t1933 = dQ3.*dQ5.*m6.*t4.*t6.*t9.*t10.*t11.*t20.*2.0;
t1934 = dQ4.*dQ6.*m6.*t5.*t6.*t9.*t10.*t11.*t20.*2.0;
t1935 = dQ1.*dQ4.*m6.*t4.*t5.*t7.*t8.*t10.*t22.*2.0;
t1936 = dQ1.*dQ4.*m5.*t4.*t5.*t7.*t8.*t10.*t25.*2.0;
t1937 = dQ1.*dQ4.*m6.*t4.*t5.*t7.*t8.*t10.*t26.*2.0;
t2032 = Ixy6.*dQ1.*dQ4.*t2.*t3.*t4.*t5.*t6.*t10.*t11.*2.0;
t2033 = Iyx6.*dQ1.*dQ4.*t2.*t3.*t4.*t5.*t6.*t10.*t11.*2.0;
t2046 = Lxcm6.*Lycm6.*dQ1.*dQ6.*m6.*t2.*t3.*t4.*t6.*t10.*t11.*4.0;
t2047 = Lxcm6.*Lz5.*dQ1.*dQ5.*m6.*t2.*t3.*t5.*t6.*t9.*t10.*4.0;
t2048 = Lxcm6.*Lzcm6.*dQ1.*dQ5.*m6.*t2.*t3.*t5.*t6.*t9.*t10.*4.0;
t2051 = Ixx6.*dQ1.*dQ6.*t2.*t3.*t5.*t6.*t9.*t10.*t11.*2.0;
t2054 = Iyy6.*dQ1.*dQ6.*t2.*t3.*t5.*t6.*t9.*t10.*t11.*2.0;
t2055 = Lycm6.*Lz5.*dQ1.*dQ4.*m6.*t2.*t4.*t6.*t8.*t9.*t10.*4.0;
t2056 = Lycm6.*Lz5.*dQ1.*dQ4.*m6.*t3.*t4.*t6.*t7.*t9.*t10.*4.0;
t2057 = Lycm6.*Lz5.*dQ1.*dQ5.*m6.*t2.*t3.*t5.*t9.*t10.*t11.*4.0;
t2058 = Lycm6.*Lzcm6.*dQ1.*dQ4.*m6.*t2.*t4.*t6.*t8.*t9.*t10.*4.0;
t2059 = Lycm6.*Lzcm6.*dQ1.*dQ4.*m6.*t3.*t4.*t6.*t7.*t9.*t10.*4.0;
t2060 = Lycm6.*Lzcm6.*dQ1.*dQ5.*m6.*t2.*t3.*t5.*t9.*t10.*t11.*4.0;
t2061 = Lz5.*Lzcm6.*dQ1.*dQ5.*m6.*t2.*t4.*t5.*t8.*t9.*t10.*4.0;
t2062 = Lz5.*Lzcm6.*dQ1.*dQ5.*m6.*t3.*t4.*t5.*t7.*t9.*t10.*4.0;
t2063 = Ixy6.*dQ1.*dQ4.*t4.*t5.*t6.*t7.*t8.*t10.*t11.*2.0;
t2064 = Iyx6.*dQ1.*dQ4.*t4.*t5.*t6.*t7.*t8.*t10.*t11.*2.0;
t2068 = Lxcm6.*Lycm6.*dQ1.*dQ6.*m6.*t4.*t6.*t7.*t8.*t10.*t11.*4.0;
t2069 = Lxcm6.*Lz5.*dQ1.*dQ4.*m6.*t2.*t4.*t8.*t9.*t10.*t11.*4.0;
t2070 = Lxcm6.*Lz5.*dQ1.*dQ4.*m6.*t3.*t4.*t7.*t9.*t10.*t11.*4.0;
t2071 = Lxcm6.*Lz5.*dQ1.*dQ5.*m6.*t5.*t6.*t7.*t8.*t9.*t10.*4.0;
t2072 = Lxcm6.*Lzcm6.*dQ1.*dQ4.*m6.*t2.*t4.*t8.*t9.*t10.*t11.*4.0;
t2073 = Lxcm6.*Lzcm6.*dQ1.*dQ4.*m6.*t3.*t4.*t7.*t9.*t10.*t11.*4.0;
t2074 = Lxcm6.*Lzcm6.*dQ1.*dQ5.*m6.*t5.*t6.*t7.*t8.*t9.*t10.*4.0;
t2075 = Ixx6.*dQ1.*dQ6.*t5.*t6.*t7.*t8.*t9.*t10.*t11.*2.0;
t2076 = Iyy6.*dQ1.*dQ6.*t5.*t6.*t7.*t8.*t9.*t10.*t11.*2.0;
t2077 = Lycm6.*Lz5.*dQ1.*dQ5.*m6.*t5.*t7.*t8.*t9.*t10.*t11.*4.0;
t2078 = Lycm6.*Lzcm6.*dQ1.*dQ5.*m6.*t5.*t7.*t8.*t9.*t10.*t11.*4.0;
t2176 = dQ1.*dQ5.*m5.*t2.*t4.*t5.*t8.*t9.*t10.*t16.*2.0;
t2177 = dQ1.*dQ5.*m5.*t3.*t4.*t5.*t7.*t9.*t10.*t16.*2.0;
t2178 = dQ1.*dQ4.*m6.*t2.*t3.*t6.*t9.*t10.*t11.*t17.*2.0;
t2179 = dQ1.*dQ6.*m6.*t2.*t4.*t6.*t8.*t9.*t11.*t17.*2.0;
t2180 = dQ1.*dQ6.*m6.*t3.*t4.*t6.*t7.*t9.*t11.*t17.*2.0;
t2181 = dQ1.*dQ5.*m6.*t2.*t4.*t5.*t8.*t9.*t10.*t20.*2.0;
t2182 = dQ1.*dQ5.*m6.*t3.*t4.*t5.*t7.*t9.*t10.*t20.*2.0;
t2183 = dQ1.*dQ4.*m6.*t2.*t3.*t6.*t9.*t10.*t11.*t20.*2.0;
t2184 = dQ1.*dQ6.*m6.*t2.*t4.*t6.*t8.*t9.*t11.*t20.*2.0;
t2185 = dQ1.*dQ6.*m6.*t3.*t4.*t6.*t7.*t9.*t11.*t20.*2.0;
t2186 = dQ1.*dQ5.*m6.*t2.*t4.*t5.*t8.*t9.*t10.*t22.*2.0;
t2187 = dQ1.*dQ5.*m6.*t3.*t4.*t5.*t7.*t9.*t10.*t22.*2.0;
t2188 = dQ1.*dQ5.*m5.*t2.*t4.*t5.*t8.*t9.*t10.*t25.*2.0;
t2189 = dQ1.*dQ5.*m5.*t3.*t4.*t5.*t7.*t9.*t10.*t25.*2.0;
t2190 = dQ1.*dQ5.*m6.*t2.*t4.*t5.*t8.*t9.*t10.*t26.*2.0;
t2191 = dQ1.*dQ5.*m6.*t3.*t4.*t5.*t7.*t9.*t10.*t26.*2.0;
t2196 = dQ1.*dQ4.*m6.*t6.*t7.*t8.*t9.*t10.*t11.*t17.*2.0;
t2197 = dQ1.*dQ4.*m6.*t6.*t7.*t8.*t9.*t10.*t11.*t20.*2.0;
t2238 = Lxcm6.*Lycm6.*dQ1.*dQ4.*m6.*t2.*t3.*t4.*t5.*t6.*t10.*t11.*4.0;
t2239 = Lycm6.*Lz5.*dQ1.*dQ6.*m6.*t2.*t4.*t5.*t6.*t8.*t9.*t10.*2.0;
t2240 = Lycm6.*Lz5.*dQ1.*dQ6.*m6.*t3.*t4.*t5.*t6.*t7.*t9.*t10.*2.0;
t2241 = Lycm6.*Lzcm6.*dQ1.*dQ6.*m6.*t2.*t4.*t5.*t6.*t8.*t9.*t10.*2.0;
t2242 = Lycm6.*Lzcm6.*dQ1.*dQ6.*m6.*t3.*t4.*t5.*t6.*t7.*t9.*t10.*2.0;
t2248 = Lxcm6.*Lycm6.*dQ1.*dQ4.*m6.*t4.*t5.*t6.*t7.*t8.*t10.*t11.*4.0;
t2249 = Lxcm6.*Lz5.*dQ1.*dQ6.*m6.*t2.*t4.*t5.*t8.*t9.*t10.*t11.*2.0;
t2250 = Lxcm6.*Lz5.*dQ1.*dQ6.*m6.*t3.*t4.*t5.*t7.*t9.*t10.*t11.*2.0;
t2251 = Lxcm6.*Lzcm6.*dQ1.*dQ6.*m6.*t2.*t4.*t5.*t8.*t9.*t10.*t11.*2.0;
t2252 = Lxcm6.*Lzcm6.*dQ1.*dQ6.*m6.*t3.*t4.*t5.*t7.*t9.*t10.*t11.*2.0;
t2328 = dQ1.*dQ4.*m6.*t2.*t4.*t5.*t6.*t8.*t9.*t11.*t17.*4.0;
t2329 = dQ1.*dQ4.*m6.*t3.*t4.*t5.*t6.*t7.*t9.*t11.*t17.*4.0;
t2330 = dQ1.*dQ6.*m6.*t2.*t3.*t5.*t6.*t9.*t10.*t11.*t17.*2.0;
t2331 = dQ1.*dQ4.*m6.*t2.*t4.*t5.*t6.*t8.*t9.*t11.*t20.*4.0;
t2332 = dQ1.*dQ4.*m6.*t3.*t4.*t5.*t6.*t7.*t9.*t11.*t20.*4.0;
t2333 = dQ1.*dQ6.*m6.*t2.*t3.*t5.*t6.*t9.*t10.*t11.*t20.*2.0;
t2334 = dQ1.*dQ6.*m6.*t5.*t6.*t7.*t8.*t9.*t10.*t11.*t17.*2.0;
t2335 = dQ1.*dQ6.*m6.*t5.*t6.*t7.*t8.*t9.*t10.*t11.*t20.*2.0;
t2377 = Lxcm6.*Lycm6.*dQ1.*dQ5.*m6.*t2.*t4.*t5.*t6.*t8.*t9.*t10.*t11.*4.0;
t2378 = Lxcm6.*Lycm6.*dQ1.*dQ5.*m6.*t3.*t4.*t5.*t6.*t7.*t9.*t10.*t11.*4.0;
t82 = -t52;
t83 = -t53;
t84 = -t59;
t85 = -t60;
t86 = -t65;
t87 = -t66;
t88 = -t70;
t89 = -t71;
t90 = -t74;
t91 = -t75;
t92 = -t76;
t93 = -t77;
t94 = Ixy6.*dQ2.*dQ6.*t34;
t95 = Ixy6.*dQ2.*dQ6.*t35;
t96 = Ixy6.*dQ3.*dQ6.*t34;
t97 = Ixy6.*dQ3.*dQ6.*t35;
t98 = t34.*t44;
t99 = t34.*t45;
t100 = Iyx6.*dQ2.*dQ6.*t34;
t101 = Iyx6.*dQ2.*dQ6.*t35;
t102 = Iyx6.*dQ3.*dQ6.*t34;
t103 = Iyx6.*dQ3.*dQ6.*t35;
t104 = t34.*t48;
t105 = t34.*t49;
t106 = Ixx4.*dQ2.*dQ4.*t39;
t107 = Ixx4.*dQ3.*dQ4.*t39;
t108 = Ixx6.*dQ2.*dQ4.*t39;
t109 = Ixx5.*dQ2.*dQ5.*t40;
t110 = Ixx6.*dQ3.*dQ4.*t39;
t111 = Ixx5.*dQ3.*dQ5.*t40;
t112 = Iyy4.*dQ2.*dQ4.*t39;
t113 = Iyy4.*dQ3.*dQ4.*t39;
t114 = Iyy5.*dQ2.*dQ4.*t39;
t115 = Iyy5.*dQ3.*dQ4.*t39;
t116 = Iyy6.*dQ2.*dQ5.*t40;
t117 = Iyy6.*dQ3.*dQ5.*t40;
t118 = Izz5.*dQ2.*dQ4.*t39;
t119 = Izz5.*dQ3.*dQ4.*t39;
t120 = Izz6.*dQ2.*dQ4.*t39;
t121 = Izz5.*dQ2.*dQ5.*t40;
t122 = Izz6.*dQ3.*dQ4.*t39;
t123 = Izz5.*dQ3.*dQ5.*t40;
t124 = Izz6.*dQ2.*dQ5.*t40;
t125 = Izz6.*dQ3.*dQ5.*t40;
t158 = t34.*t42.*2.0;
t159 = t34.*t43.*2.0;
t160 = t35.*t44.*2.0;
t161 = t35.*t45.*2.0;
t162 = t34.*t46.*2.0;
t163 = t34.*t47.*2.0;
t164 = t35.*t48.*2.0;
t165 = t35.*t49.*2.0;
t197 = t34.*t55;
t198 = t34.*t56;
t199 = t34.*t62;
t200 = t34.*t63;
t201 = t34.*t70;
t202 = t34.*t71;
t203 = t34.*t74;
t204 = t34.*t75;
t299 = -t166;
t300 = -t167;
t301 = -t168;
t302 = -t169;
t303 = -t172;
t304 = -t173;
t305 = -t175;
t306 = -t176;
t307 = -t130;
t308 = -t131;
t309 = -t133;
t310 = -t134;
t311 = -t135;
t312 = -t136;
t313 = -t137;
t314 = -t140;
t315 = -t181;
t316 = -t182;
t317 = -t183;
t318 = -t184;
t319 = -t187;
t320 = -t188;
t321 = -t189;
t322 = -t190;
t323 = -t191;
t324 = -t192;
t325 = -t193;
t326 = -t194;
t327 = -t195;
t328 = -t196;
t329 = t34.*t50.*2.0;
t330 = t34.*t51.*2.0;
t331 = t34.*t52.*2.0;
t332 = t34.*t53.*2.0;
t333 = t36.*t52.*2.0;
t334 = t36.*t53.*2.0;
t335 = t36.*t54.*2.0;
t336 = t35.*t55.*2.0;
t337 = t35.*t56.*2.0;
t338 = t34.*t57.*2.0;
t339 = t34.*t58.*2.0;
t340 = t34.*t59.*2.0;
t341 = t34.*t60.*2.0;
t342 = t36.*t59.*2.0;
t343 = t36.*t60.*2.0;
t344 = t36.*t61.*2.0;
t345 = t35.*t62.*2.0;
t346 = t35.*t63.*2.0;
t347 = Lxcm4.*Lycm4.*dQ2.*dQ4.*m4.*t34.*4.0;
t348 = Lxcm4.*Lycm4.*dQ3.*dQ4.*m4.*t34.*4.0;
t349 = Lxcm6.*Lycm6.*dQ2.*dQ6.*m6.*t34.*2.0;
t350 = Lxcm6.*Lycm6.*dQ2.*dQ6.*m6.*t35.*2.0;
t351 = Lxcm6.*Lycm6.*dQ3.*dQ6.*m6.*t34.*2.0;
t352 = Lxcm6.*Lycm6.*dQ3.*dQ6.*m6.*t35.*2.0;
t355 = Lxcm5.*Lzcm5.*dQ2.*dQ5.*m5.*t35.*4.0;
t356 = Lxcm5.*Lzcm5.*dQ3.*dQ5.*m5.*t35.*4.0;
t357 = t35.*t64.*2.0;
t358 = t36.*t65.*2.0;
t359 = t35.*t67.*2.0;
t360 = t36.*t67.*2.0;
t361 = t34.*t68.*2.0;
t362 = t34.*t69.*2.0;
t363 = t35.*t70.*2.0;
t364 = t35.*t71.*2.0;
t365 = t34.*t72.*2.0;
t366 = t34.*t73.*2.0;
t367 = t35.*t74.*2.0;
t368 = t35.*t75.*2.0;
t369 = t35.*t76.*2.0;
t370 = t35.*t77.*2.0;
t371 = Lz5.*Lzcm6.*dQ2.*dQ4.*m6.*t39.*2.0;
t372 = Lz5.*Lzcm6.*dQ3.*dQ4.*m6.*t39.*2.0;
t373 = Lz5.*Lzcm6.*dQ2.*dQ5.*m6.*t40.*2.0;
t374 = Lz5.*Lzcm6.*dQ3.*dQ5.*m6.*t40.*2.0;
t375 = dQ2.*dQ4.*m4.*t15.*t39;
t376 = dQ3.*dQ4.*m4.*t15.*t39;
t377 = dQ2.*dQ5.*m5.*t16.*t40;
t378 = dQ2.*dQ4.*m6.*t17.*t39;
t379 = dQ3.*dQ5.*m5.*t16.*t40;
t380 = dQ3.*dQ4.*m6.*t17.*t39;
t381 = dQ2.*dQ4.*m4.*t18.*t39;
t382 = dQ3.*dQ4.*m4.*t18.*t39;
t383 = dQ2.*dQ4.*m5.*t19.*t39;
t384 = dQ3.*dQ4.*m5.*t19.*t39;
t385 = dQ2.*dQ5.*m6.*t20.*t40;
t386 = dQ3.*dQ5.*m6.*t20.*t40;
t387 = dQ2.*dQ4.*m6.*t22.*t39;
t388 = dQ3.*dQ4.*m6.*t22.*t39;
t389 = dQ2.*dQ5.*m6.*t22.*t40;
t390 = dQ3.*dQ5.*m6.*t22.*t40;
t391 = dQ2.*dQ4.*m5.*t25.*t39;
t392 = dQ3.*dQ4.*m5.*t25.*t39;
t393 = dQ2.*dQ5.*m5.*t25.*t40;
t394 = dQ2.*dQ4.*m6.*t26.*t39;
t395 = dQ3.*dQ5.*m5.*t25.*t40;
t396 = dQ3.*dQ4.*m6.*t26.*t39;
t397 = dQ2.*dQ5.*m6.*t26.*t40;
t398 = dQ3.*dQ5.*m6.*t26.*t40;
t461 = Ixz6.*dQ4.*dQ6.*t9.*t11.*t35;
t462 = Izx6.*dQ4.*dQ6.*t9.*t11.*t35;
t481 = Lxcm5.*Lzcm5.*dQ2.*dQ5.*m5.*t34.*-2.0;
t482 = Lxcm5.*Lzcm5.*dQ3.*dQ5.*m5.*t34.*-2.0;
t554 = -t221;
t555 = -t223;
out1 = ft_2({Ixx2,Ixx3,Ixx4,Ixx5,Ixx6,Ixy3,Ixy4,Ixy5,Ixy6,Ixz2,Ixz3,Ixz4,Ixz5,Ixz6,Iyx3,Iyx4,Iyx5,Iyx6,Iyy4,Iyy5,Iyy6,Iyz3,Iyz4,Iyz5,Iyz6,Izx2,Izx3,Izx4,Izx5,Izx6,Izy3,Izy4,Izy5,Izy6,Izz2,Izz3,Izz4,Izz5,Izz6,Lx2,Lx3,Lxcm2,Lxcm3,Lxcm4,Lxcm5,Lxcm6,Lycm3,Lycm4,Lycm5,Lycm6,Lz4,Lz5,Lzcm2,Lzcm3,Lzcm4,Lzcm5,Lzcm6,dQ1,dQ2,dQ3,dQ4,dQ5,dQ6,m2,m3,m4,m5,m6,t10,t100,t1000,t101,t102,t103,t1031,t1032,t1033,t1034,t1035,t1036,t1037,t1038,t1039,t104,t1040,t1041,t1042,t1043,t1044,t1045,t1046,t1047,t1048,t1049,t105,t1050,t1051,t1052,t1053,t1054,t1055,t1056,t1057,t1058,t1059,t106,t1060,t1061,t1062,t1063,t1064,t1065,t1066,t1067,t1068,t1069,t107,t1070,t1071,t1072,t1073,t1074,t1075,t1076,t1077,t1078,t1079,t108,t1080,t1081,t1086,t1087,t1088,t1089,t109,t1090,t1091,t1092,t1093,t1094,t1095,t1096,t1097,t1098,t1099,t11,t110,t1100,t1101,t1102,t1103,t1104,t1105,t1106,t1107,t1108,t1109,t111,t1110,t1111,t1112,t1113,t1114,t1115,t1116,t1117,t1118,t1119,t112,t1120,t1121,t1122,t1123,t1124,t1125,t1126,t1127,t1128,t1129,t113,t1130,t1131,t1132,t1133,t1134,t1135,t1136,t1137,t1138,t1139,t114,t1140,t1141,t1142,t1143,t1144,t1145,t1146,t1147,t1148,t1149,t115,t1150,t1151,t1152,t1153,t1154,t1155,t1156,t1157,t1158,t1159,t116,t1160,t1161,t1162,t1163,t1164,t1165,t1166,t1167,t1168,t1169,t117,t1170,t1171,t1172,t1173,t1174,t1175,t1176,t1177,t1178,t1179,t118,t1180,t1181,t1182,t1183,t1184,t1185,t1186,t1187,t1188,t1189,t119,t1190,t12,t120,t121,t122,t123,t124,t125,t126,t127,t128,t1282,t1283,t1284,t1285,t129,t13,t130,t131,t132,t133,t134,t1344,t135,t136,t137,t138,t1380,t139,t14,t140,t141,t142,t143,t144,t145,t146,t147,t148,t149,t15,t150,t151,t152,t1522,t153,t154,t155,t156,t157,t158,t159,t16,t160,t161,t162,t1624,t1625,t1626,t1627,t1628,t1629,t163,t1630,t1631,t1632,t1633,t1634,t1635,t1636,t1637,t1638,t1639,t164,t165,t1666,t1667,t1668,t1669,t1670,t1671,t1672,t1673,t1674,t1675,t1676,t1677,t1678,t1679,t1680,t1681,t1682,t1683,t1684,t1685,t1686,t1687,t1688,t1689,t1690,t1691,t1692,t1693,t1694,t1695,t1696,t1697,t1698,t1699,t17,t170,t1700,t1701,t1702,t1703,t1704,t1705,t1706,t1707,t1708,t1709,t171,t1710,t1711,t1712,t1713,t1714,t1715,t1716,t1717,t1718,t1719,t172,t1720,t1721,t1722,t1723,t1724,t1725,t1726,t1727,t1728,t1729,t173,t1730,t1731,t1732,t1733,t1734,t1735,t1736,t1737,t1738,t1739,t174,t1740,t1741,t1742,t1743,t1744,t1745,t1746,t1747,t1748,t1749,t1750,t1751,t1752,t1753,t1754,t1755,t1756,t177,t178,t179,t18,t180,t183,t1836,t1837,t1838,t1839,t184,t1842,t1843,t1844,t1845,t185,t186,t1869,t187,t1870,t1879,t188,t1880,t1881,t1882,t1883,t19,t1923,t1924,t1925,t1926,t1927,t1928,t1929,t1930,t1931,t1932,t1933,t1934,t1935,t1936,t1937,t195,t196,t197,t198,t199,t2,t20,t200,t201,t202,t203,t2032,t2033,t204,t2046,t2047,t2048,t2051,t2054,t2055,t2056,t2057,t2058,t2059,t2060,t2061,t2062,t2063,t2064,t2068,t2069,t2070,t2071,t2072,t2073,t2074,t2075,t2076,t2077,t2078,t21,t2176,t2177,t2178,t2179,t2180,t2181,t2182,t2183,t2184,t2185,t2186,t2187,t2188,t2189,t2190,t2191,t2196,t2197,t22,t222,t2238,t2239,t224,t2240,t2241,t2242,t2248,t2249,t225,t2250,t2251,t2252,t226,t23,t2328,t2329,t2330,t2331,t2332,t2333,t2334,t2335,t237,t2377,t2378,t238,t239,t24,t240,t241,t242,t243,t244,t245,t246,t247,t248,t249,t25,t250,t251,t252,t253,t254,t255,t256,t257,t258,t259,t26,t260,t261,t262,t263,t264,t265,t266,t267,t268,t269,t270,t271,t272,t273,t274,t275,t276,t277,t278,t279,t280,t281,t282,t283,t284,t285,t286,t287,t288,t289,t290,t291,t292,t293,t294,t295,t296,t297,t298,t299,t3,t300,t301,t302,t303,t304,t305,t306,t307,t308,t309,t310,t311,t312,t313,t314,t315,t316,t317,t318,t319,t32,t320,t321,t322,t323,t324,t325,t326,t327,t328,t329,t33,t330,t331,t332,t333,t334,t335,t336,t337,t338,t339,t34,t340,t341,t342,t343,t344,t345,t346,t347,t348,t349,t35,t350,t351,t352,t355,t356,t357,t358,t359,t36,t360,t361,t362,t363,t364,t365,t366,t367,t368,t369,t37,t370,t371,t372,t373,t374,t375,t376,t377,t378,t379,t38,t380,t381,t382,t383,t384,t385,t386,t387,t388,t389,t39,t390,t391,t392,t393,t394,t395,t396,t397,t398,t399,t4,t40,t400,t401,t402,t403,t404,t405,t406,t407,t408,t409,t41,t410,t411,t412,t413,t414,t415,t416,t417,t418,t419,t42,t420,t421,t422,t423,t424,t425,t426,t427,t428,t429,t43,t430,t431,t432,t433,t434,t435,t436,t437,t438,t439,t44,t440,t441,t442,t443,t444,t445,t446,t447,t448,t449,t45,t450,t451,t452,t453,t454,t455,t456,t457,t458,t459,t46,t460,t461,t462,t47,t48,t481,t482,t485,t486,t49,t498,t499,t5,t50,t500,t501,t502,t503,t504,t505,t506,t507,t508,t509,t51,t510,t511,t512,t513,t514,t515,t516,t517,t518,t519,t52,t520,t521,t522,t523,t524,t525,t526,t527,t528,t529,t53,t530,t531,t532,t533,t534,t535,t536,t537,t538,t539,t54,t540,t541,t542,t543,t544,t545,t546,t547,t548,t549,t55,t550,t551,t552,t553,t554,t555,t56,t57,t58,t59,t6,t60,t61,t615,t616,t617,t618,t619,t62,t620,t621,t622,t63,t64,t644,t645,t646,t647,t648,t649,t65,t650,t651,t652,t653,t654,t655,t656,t657,t658,t659,t660,t661,t662,t663,t664,t665,t666,t667,t668,t669,t67,t670,t671,t672,t673,t674,t675,t676,t677,t678,t679,t68,t680,t681,t682,t683,t684,t685,t686,t687,t688,t689,t69,t690,t691,t692,t693,t694,t695,t696,t697,t7,t70,t71,t712,t713,t714,t715,t716,t717,t718,t719,t72,t720,t721,t722,t723,t724,t725,t726,t727,t728,t729,t73,t730,t731,t732,t733,t734,t735,t736,t737,t738,t739,t74,t740,t741,t742,t743,t744,t75,t78,t79,t8,t80,t81,t82,t83,t831,t832,t833,t834,t839,t84,t840,t841,t842,t843,t844,t845,t846,t847,t848,t85,t856,t857,t858,t859,t86,t860,t861,t862,t863,t864,t865,t866,t867,t87,t88,t89,t9,t90,t91,t92,t93,t937,t938,t939,t94,t940,t941,t942,t943,t944,t945,t946,t947,t948,t949,t95,t950,t96,t962,t963,t97,t98,t99,t999});
end
function out1 = ft_2(ct)
[Ixx2,Ixx3,Ixx4,Ixx5,Ixx6,Ixy3,Ixy4,Ixy5,Ixy6,Ixz2,Ixz3,Ixz4,Ixz5,Ixz6,Iyx3,Iyx4,Iyx5,Iyx6,Iyy4,Iyy5,Iyy6,Iyz3,Iyz4,Iyz5,Iyz6,Izx2,Izx3,Izx4,Izx5,Izx6,Izy3,Izy4,Izy5,Izy6,Izz2,Izz3,Izz4,Izz5,Izz6,Lx2,Lx3,Lxcm2,Lxcm3,Lxcm4,Lxcm5,Lxcm6,Lycm3,Lycm4,Lycm5,Lycm6,Lz4,Lz5,Lzcm2,Lzcm3,Lzcm4,Lzcm5,Lzcm6,dQ1,dQ2,dQ3,dQ4,dQ5,dQ6,m2,m3,m4,m5,m6,t10,t100,t1000,t101,t102,t103,t1031,t1032,t1033,t1034,t1035,t1036,t1037,t1038,t1039,t104,t1040,t1041,t1042,t1043,t1044,t1045,t1046,t1047,t1048,t1049,t105,t1050,t1051,t1052,t1053,t1054,t1055,t1056,t1057,t1058,t1059,t106,t1060,t1061,t1062,t1063,t1064,t1065,t1066,t1067,t1068,t1069,t107,t1070,t1071,t1072,t1073,t1074,t1075,t1076,t1077,t1078,t1079,t108,t1080,t1081,t1086,t1087,t1088,t1089,t109,t1090,t1091,t1092,t1093,t1094,t1095,t1096,t1097,t1098,t1099,t11,t110,t1100,t1101,t1102,t1103,t1104,t1105,t1106,t1107,t1108,t1109,t111,t1110,t1111,t1112,t1113,t1114,t1115,t1116,t1117,t1118,t1119,t112,t1120,t1121,t1122,t1123,t1124,t1125,t1126,t1127,t1128,t1129,t113,t1130,t1131,t1132,t1133,t1134,t1135,t1136,t1137,t1138,t1139,t114,t1140,t1141,t1142,t1143,t1144,t1145,t1146,t1147,t1148,t1149,t115,t1150,t1151,t1152,t1153,t1154,t1155,t1156,t1157,t1158,t1159,t116,t1160,t1161,t1162,t1163,t1164,t1165,t1166,t1167,t1168,t1169,t117,t1170,t1171,t1172,t1173,t1174,t1175,t1176,t1177,t1178,t1179,t118,t1180,t1181,t1182,t1183,t1184,t1185,t1186,t1187,t1188,t1189,t119,t1190,t12,t120,t121,t122,t123,t124,t125,t126,t127,t128,t1282,t1283,t1284,t1285,t129,t13,t130,t131,t132,t133,t134,t1344,t135,t136,t137,t138,t1380,t139,t14,t140,t141,t142,t143,t144,t145,t146,t147,t148,t149,t15,t150,t151,t152,t1522,t153,t154,t155,t156,t157,t158,t159,t16,t160,t161,t162,t1624,t1625,t1626,t1627,t1628,t1629,t163,t1630,t1631,t1632,t1633,t1634,t1635,t1636,t1637,t1638,t1639,t164,t165,t1666,t1667,t1668,t1669,t1670,t1671,t1672,t1673,t1674,t1675,t1676,t1677,t1678,t1679,t1680,t1681,t1682,t1683,t1684,t1685,t1686,t1687,t1688,t1689,t1690,t1691,t1692,t1693,t1694,t1695,t1696,t1697,t1698,t1699,t17,t170,t1700,t1701,t1702,t1703,t1704,t1705,t1706,t1707,t1708,t1709,t171,t1710,t1711,t1712,t1713,t1714,t1715,t1716,t1717,t1718,t1719,t172,t1720,t1721,t1722,t1723,t1724,t1725,t1726,t1727,t1728,t1729,t173,t1730,t1731,t1732,t1733,t1734,t1735,t1736,t1737,t1738,t1739,t174,t1740,t1741,t1742,t1743,t1744,t1745,t1746,t1747,t1748,t1749,t1750,t1751,t1752,t1753,t1754,t1755,t1756,t177,t178,t179,t18,t180,t183,t1836,t1837,t1838,t1839,t184,t1842,t1843,t1844,t1845,t185,t186,t1869,t187,t1870,t1879,t188,t1880,t1881,t1882,t1883,t19,t1923,t1924,t1925,t1926,t1927,t1928,t1929,t1930,t1931,t1932,t1933,t1934,t1935,t1936,t1937,t195,t196,t197,t198,t199,t2,t20,t200,t201,t202,t203,t2032,t2033,t204,t2046,t2047,t2048,t2051,t2054,t2055,t2056,t2057,t2058,t2059,t2060,t2061,t2062,t2063,t2064,t2068,t2069,t2070,t2071,t2072,t2073,t2074,t2075,t2076,t2077,t2078,t21,t2176,t2177,t2178,t2179,t2180,t2181,t2182,t2183,t2184,t2185,t2186,t2187,t2188,t2189,t2190,t2191,t2196,t2197,t22,t222,t2238,t2239,t224,t2240,t2241,t2242,t2248,t2249,t225,t2250,t2251,t2252,t226,t23,t2328,t2329,t2330,t2331,t2332,t2333,t2334,t2335,t237,t2377,t2378,t238,t239,t24,t240,t241,t242,t243,t244,t245,t246,t247,t248,t249,t25,t250,t251,t252,t253,t254,t255,t256,t257,t258,t259,t26,t260,t261,t262,t263,t264,t265,t266,t267,t268,t269,t270,t271,t272,t273,t274,t275,t276,t277,t278,t279,t280,t281,t282,t283,t284,t285,t286,t287,t288,t289,t290,t291,t292,t293,t294,t295,t296,t297,t298,t299,t3,t300,t301,t302,t303,t304,t305,t306,t307,t308,t309,t310,t311,t312,t313,t314,t315,t316,t317,t318,t319,t32,t320,t321,t322,t323,t324,t325,t326,t327,t328,t329,t33,t330,t331,t332,t333,t334,t335,t336,t337,t338,t339,t34,t340,t341,t342,t343,t344,t345,t346,t347,t348,t349,t35,t350,t351,t352,t355,t356,t357,t358,t359,t36,t360,t361,t362,t363,t364,t365,t366,t367,t368,t369,t37,t370,t371,t372,t373,t374,t375,t376,t377,t378,t379,t38,t380,t381,t382,t383,t384,t385,t386,t387,t388,t389,t39,t390,t391,t392,t393,t394,t395,t396,t397,t398,t399,t4,t40,t400,t401,t402,t403,t404,t405,t406,t407,t408,t409,t41,t410,t411,t412,t413,t414,t415,t416,t417,t418,t419,t42,t420,t421,t422,t423,t424,t425,t426,t427,t428,t429,t43,t430,t431,t432,t433,t434,t435,t436,t437,t438,t439,t44,t440,t441,t442,t443,t444,t445,t446,t447,t448,t449,t45,t450,t451,t452,t453,t454,t455,t456,t457,t458,t459,t46,t460,t461,t462,t47,t48,t481,t482,t485,t486,t49,t498,t499,t5,t50,t500,t501,t502,t503,t504,t505,t506,t507,t508,t509,t51,t510,t511,t512,t513,t514,t515,t516,t517,t518,t519,t52,t520,t521,t522,t523,t524,t525,t526,t527,t528,t529,t53,t530,t531,t532,t533,t534,t535,t536,t537,t538,t539,t54,t540,t541,t542,t543,t544,t545,t546,t547,t548,t549,t55,t550,t551,t552,t553,t554,t555,t56,t57,t58,t59,t6,t60,t61,t615,t616,t617,t618,t619,t62,t620,t621,t622,t63,t64,t644,t645,t646,t647,t648,t649,t65,t650,t651,t652,t653,t654,t655,t656,t657,t658,t659,t660,t661,t662,t663,t664,t665,t666,t667,t668,t669,t67,t670,t671,t672,t673,t674,t675,t676,t677,t678,t679,t68,t680,t681,t682,t683,t684,t685,t686,t687,t688,t689,t69,t690,t691,t692,t693,t694,t695,t696,t697,t7,t70,t71,t712,t713,t714,t715,t716,t717,t718,t719,t72,t720,t721,t722,t723,t724,t725,t726,t727,t728,t729,t73,t730,t731,t732,t733,t734,t735,t736,t737,t738,t739,t74,t740,t741,t742,t743,t744,t75,t78,t79,t8,t80,t81,t82,t83,t831,t832,t833,t834,t839,t84,t840,t841,t842,t843,t844,t845,t846,t847,t848,t85,t856,t857,t858,t859,t86,t860,t861,t862,t863,t864,t865,t866,t867,t87,t88,t89,t9,t90,t91,t92,t93,t937,t938,t939,t94,t940,t941,t942,t943,t944,t945,t946,t947,t948,t949,t95,t950,t96,t962,t963,t97,t98,t99,t999] = ct{:};
t556 = -t224;
t557 = -t226;
t558 = -t399;
t559 = -t400;
t560 = -t401;
t561 = -t408;
t562 = -t409;
t563 = -t410;
t568 = -t238;
t569 = -t239;
t570 = -t240;
t571 = -t411;
t572 = -t412;
t573 = -t413;
t574 = -t414;
t575 = -t241;
t576 = -t420;
t577 = -t246;
t578 = -t247;
t579 = -t248;
t580 = -t249;
t581 = -t254;
t582 = -t255;
t583 = -t256;
t584 = -t257;
t585 = -t261;
t586 = -t262;
t587 = -t421;
t588 = -t422;
t589 = -t423;
t590 = -t424;
t591 = -t425;
t592 = -t426;
t593 = -t427;
t594 = -t428;
t595 = -t429;
t596 = -t439;
t597 = -t440;
t598 = -t441;
t599 = -t267;
t600 = -t268;
t601 = -t271;
t602 = -t272;
t603 = -t275;
t604 = -t280;
t605 = -t281;
t606 = -t284;
t607 = -t285;
t608 = -t288;
t609 = -t448;
t610 = -t449;
t611 = -t450;
t612 = -t451;
t613 = -t452;
t614 = -t453;
t623 = -t291;
t624 = -t294;
t625 = -t295;
t626 = -t296;
t627 = Iyz6.*dQ4.*dQ6.*t6.*t9.*t35;
t628 = Izy6.*dQ4.*dQ6.*t6.*t9.*t35;
t629 = t34.*t183;
t630 = t34.*t184;
t631 = Lycm6.*Lz5.*dQ2.*dQ5.*m6.*t11.*t35.*4.0;
t632 = Lycm6.*Lz5.*dQ3.*dQ5.*m6.*t11.*t35.*4.0;
t633 = Lycm5.*Lzcm5.*dQ2.*dQ4.*m5.*t10.*t34.*4.0;
t634 = Lycm5.*Lzcm5.*dQ3.*dQ4.*m5.*t10.*t34.*4.0;
t635 = t34.*t187;
t636 = t34.*t188;
t637 = Lycm6.*Lzcm6.*dQ2.*dQ5.*m6.*t11.*t35.*4.0;
t638 = Lycm6.*Lzcm6.*dQ3.*dQ5.*m6.*t11.*t35.*4.0;
t639 = Lz5.*Lzcm6.*dQ4.*dQ5.*m6.*t9.*t35.*4.0;
t640 = t34.*t154.*2.0;
t641 = t34.*t155.*2.0;
t642 = t34.*t156.*2.0;
t643 = t34.*t157.*2.0;
t757 = Lxcm5.*Lycm5.*dQ2.*dQ4.*m5.*t5.*t34.*4.0;
t758 = Lxcm5.*Lycm5.*dQ3.*dQ4.*m5.*t5.*t34.*4.0;
t759 = Lxcm6.*Lycm6.*dQ2.*dQ4.*m6.*t5.*t34.*4.0;
t760 = Lxcm6.*Lycm6.*dQ3.*dQ4.*m6.*t5.*t34.*4.0;
t761 = Lxcm6.*Lycm6.*dQ2.*dQ4.*m6.*t5.*t36.*4.0;
t762 = Lxcm6.*Lycm6.*dQ3.*dQ4.*m6.*t5.*t36.*4.0;
t763 = Lxcm6.*Lycm6.*dQ5.*dQ6.*m6.*t4.*t36.*4.0;
t766 = Lxcm6.*Lz5.*dQ2.*dQ5.*m6.*t6.*t35.*4.0;
t767 = Lxcm6.*Lz5.*dQ3.*dQ5.*m6.*t6.*t35.*4.0;
t770 = Lxcm6.*Lzcm6.*dQ2.*dQ5.*m6.*t6.*t35.*4.0;
t771 = Lxcm6.*Lzcm6.*dQ3.*dQ5.*m6.*t6.*t35.*4.0;
t772 = t34.*t126.*2.0;
t773 = t34.*t127.*2.0;
t774 = t34.*t130.*2.0;
t775 = t34.*t131.*2.0;
t776 = t36.*t130.*2.0;
t777 = t36.*t131.*2.0;
t778 = Ixx5.*dQ2.*dQ4.*t4.*t9.*t35.*2.0;
t779 = Ixx5.*dQ3.*dQ4.*t4.*t9.*t35.*2.0;
t780 = Ixx5.*dQ2.*dQ5.*t5.*t10.*t34.*2.0;
t781 = Ixx6.*dQ2.*dQ4.*t4.*t9.*t36.*2.0;
t782 = Ixx5.*dQ3.*dQ5.*t5.*t10.*t34.*2.0;
t783 = Ixx6.*dQ3.*dQ4.*t4.*t9.*t36.*2.0;
t784 = Ixx6.*dQ2.*dQ5.*t5.*t10.*t36.*2.0;
t785 = Ixx6.*dQ2.*dQ6.*t6.*t11.*t34.*2.0;
t786 = Ixx6.*dQ3.*dQ5.*t5.*t10.*t36.*2.0;
t787 = Ixx6.*dQ2.*dQ6.*t6.*t11.*t35.*2.0;
t788 = Ixx6.*dQ3.*dQ6.*t6.*t11.*t34.*2.0;
t789 = t36.*t132.*2.0;
t790 = Ixx6.*dQ3.*dQ6.*t6.*t11.*t35.*2.0;
t791 = t36.*t133.*2.0;
t792 = t34.*t134.*2.0;
t793 = t34.*t135.*2.0;
t794 = t34.*t136.*2.0;
t795 = t34.*t137.*2.0;
t796 = t36.*t138.*2.0;
t797 = t36.*t139.*2.0;
t798 = Iyy6.*dQ2.*dQ4.*t4.*t9.*t35.*2.0;
t799 = Iyy6.*dQ2.*dQ4.*t4.*t9.*t36.*2.0;
t800 = Iyy6.*dQ3.*dQ4.*t4.*t9.*t35.*2.0;
t801 = Iyy6.*dQ2.*dQ5.*t5.*t10.*t34.*2.0;
t802 = Iyy6.*dQ3.*dQ4.*t4.*t9.*t36.*2.0;
t803 = Iyy6.*dQ3.*dQ5.*t5.*t10.*t34.*2.0;
t804 = Iyy6.*dQ2.*dQ5.*t5.*t10.*t36.*2.0;
t805 = Iyy6.*dQ2.*dQ6.*t6.*t11.*t34.*2.0;
t806 = Iyy6.*dQ3.*dQ5.*t5.*t10.*t36.*2.0;
t807 = Iyy6.*dQ2.*dQ6.*t6.*t11.*t35.*2.0;
t808 = Iyy6.*dQ3.*dQ6.*t6.*t11.*t34.*2.0;
t809 = t36.*t140.*2.0;
t810 = Iyy6.*dQ3.*dQ6.*t6.*t11.*t35.*2.0;
t811 = t36.*t141.*2.0;
t812 = t34.*t142.*2.0;
t813 = t34.*t143.*2.0;
t814 = t34.*t144.*2.0;
t815 = t34.*t145.*2.0;
t816 = t34.*t148.*2.0;
t817 = t34.*t149.*2.0;
t818 = t34.*t150.*2.0;
t819 = t34.*t151.*2.0;
t820 = Izz5.*dQ2.*dQ4.*t4.*t9.*t35.*2.0;
t821 = Izz5.*dQ3.*dQ4.*t4.*t9.*t35.*2.0;
t822 = Izz6.*dQ2.*dQ4.*t4.*t9.*t35.*2.0;
t823 = Izz5.*dQ2.*dQ5.*t5.*t10.*t34.*2.0;
t824 = Izz6.*dQ3.*dQ4.*t4.*t9.*t35.*2.0;
t825 = Izz5.*dQ3.*dQ5.*t5.*t10.*t34.*2.0;
t826 = Izz6.*dQ2.*dQ5.*t5.*t10.*t34.*2.0;
t827 = Izz6.*dQ3.*dQ5.*t5.*t10.*t34.*2.0;
t849 = t35.*t195;
t850 = dQ4.*dQ5.*m6.*t9.*t17.*t36.*2.0;
t851 = t35.*t196;
t852 = t36.*t196;
t853 = dQ4.*dQ5.*m6.*t9.*t22.*t35.*2.0;
t854 = dQ4.*dQ5.*m5.*t9.*t25.*t35.*2.0;
t855 = dQ4.*dQ5.*m6.*t9.*t26.*t35.*2.0;
t868 = -t644;
t869 = -t645;
t870 = -t646;
t871 = -t647;
t872 = -t649;
t873 = -t499;
t874 = -t501;
t875 = -t502;
t876 = -t503;
t877 = -t504;
t878 = -t505;
t879 = -t507;
t880 = -t508;
t881 = -t509;
t882 = -t510;
t883 = -t511;
t884 = -t652;
t885 = -t653;
t886 = -t654;
t887 = -t655;
t888 = -t656;
t889 = -t657;
t890 = -t665;
t891 = -t666;
t892 = -t667;
t893 = -t668;
t894 = -t672;
t895 = -t673;
t896 = -t513;
t897 = -t678;
t898 = -t679;
t899 = -t680;
t900 = -t517;
t901 = -t518;
t902 = -t519;
t903 = -t520;
t904 = -t521;
t905 = -t682;
t906 = -t683;
t907 = -t522;
t908 = -t523;
t909 = -t524;
t910 = -t525;
t911 = -t685;
t912 = -t686;
t913 = -t526;
t914 = -t691;
t915 = -t692;
t916 = -t693;
t917 = -t530;
t918 = -t531;
t919 = -t532;
t920 = -t533;
t921 = -t534;
t922 = -t695;
t923 = -t696;
t924 = -t535;
t925 = -t536;
t926 = -t537;
t927 = -t538;
t928 = -t712;
t929 = -t713;
t930 = -t714;
t931 = -t715;
t932 = -t722;
t933 = -t723;
t934 = -t726;
t935 = -t727;
t936 = -t736;
t951 = -t539;
t952 = -t541;
t953 = -t740;
t954 = -t545;
t955 = -t741;
t956 = -t549;
t957 = -t742;
t958 = -t743;
t959 = -t744;
t960 = -t551;
t961 = -t553;
t968 = t34.*t246;
t969 = t34.*t247;
t970 = t34.*t250;
t971 = t34.*t251;
t972 = t34.*t254;
t973 = t34.*t255;
t974 = t34.*t258;
t975 = t34.*t259;
t976 = t34.*t265;
t977 = t34.*t266;
t978 = t34.*t267;
t979 = t34.*t268;
t980 = t34.*t276;
t981 = t34.*t277;
t982 = t34.*t278;
t983 = t34.*t279;
t984 = t34.*t280;
t985 = t34.*t281;
t986 = t34.*t289;
t987 = t34.*t290;
t991 = Lxcm6.*Lz5.*dQ2.*dQ5.*m6.*t6.*t34.*-2.0;
t992 = Lxcm6.*Lz5.*dQ3.*dQ5.*m6.*t6.*t34.*-2.0;
t995 = Lxcm6.*Lzcm6.*dQ2.*dQ5.*m6.*t6.*t34.*-2.0;
t996 = Lxcm6.*Lzcm6.*dQ3.*dQ5.*m6.*t6.*t34.*-2.0;
t1191 = t34.*t36.*t52.*4.0;
t1192 = t34.*t36.*t53.*4.0;
t1195 = t34.*t36.*t59.*4.0;
t1196 = t34.*t36.*t60.*4.0;
t1201 = Lxcm6.*Lycm6.*dQ2.*dQ6.*m6.*t34.*t36.*4.0;
t1202 = Lxcm6.*Lycm6.*dQ2.*dQ6.*m6.*t35.*t36.*4.0;
t1203 = Lxcm6.*Lycm6.*dQ3.*dQ6.*m6.*t34.*t36.*4.0;
t1204 = Lxcm6.*Lycm6.*dQ3.*dQ6.*m6.*t35.*t36.*4.0;
t1213 = -t937;
t1214 = -t944;
t1215 = -t945;
t1216 = -t946;
t1217 = -t947;
t1218 = -t948;
t1219 = -t949;
t1220 = t35.*t222.*2.0;
t1221 = t35.*t225.*2.0;
t1222 = t35.*t237.*2.0;
t1223 = t36.*t238.*2.0;
t1224 = t34.*t239.*2.0;
t1225 = t34.*t240.*2.0;
t1226 = t36.*t239.*2.0;
t1227 = t36.*t240.*2.0;
t1228 = Ixx6.*dQ2.*dQ4.*t5.*t6.*t11.*t34.*4.0;
t1229 = Ixx6.*dQ2.*dQ6.*t4.*t5.*t9.*t36.*4.0;
t1230 = Ixx6.*dQ3.*dQ4.*t5.*t6.*t11.*t34.*4.0;
t1231 = Ixx6.*dQ3.*dQ6.*t4.*t5.*t9.*t36.*4.0;
t1232 = t35.*t242.*2.0;
t1233 = t36.*t242.*2.0;
t1234 = t34.*t243.*2.0;
t1235 = t34.*t244.*2.0;
t1236 = t36.*t243.*2.0;
t1237 = t36.*t244.*2.0;
t1238 = Iyy6.*dQ2.*dQ4.*t5.*t6.*t11.*t34.*4.0;
t1239 = Iyy6.*dQ2.*dQ6.*t4.*t5.*t9.*t36.*4.0;
t1240 = Iyy6.*dQ3.*dQ4.*t5.*t6.*t11.*t34.*4.0;
t1241 = Iyy6.*dQ3.*dQ6.*t4.*t5.*t9.*t36.*4.0;
t1242 = t35.*t261.*2.0;
t1243 = t35.*t262.*2.0;
t1244 = Lycm6.*Lz5.*dQ2.*dQ4.*m6.*t6.*t10.*t34.*4.0;
t1245 = Lycm6.*Lz5.*dQ3.*dQ4.*m6.*t6.*t10.*t34.*4.0;
t1246 = Lycm6.*Lz5.*dQ4.*dQ6.*m6.*t6.*t9.*t35.*2.0;
t1247 = Lycm6.*Lzcm6.*dQ2.*dQ4.*m6.*t6.*t10.*t34.*4.0;
t1248 = Lycm6.*Lzcm6.*dQ3.*dQ4.*m6.*t6.*t10.*t34.*4.0;
t1249 = Lycm6.*Lzcm6.*dQ4.*dQ6.*m6.*t6.*t9.*t35.*2.0;
t1250 = Lz5.*Lzcm6.*dQ1.*dQ4.*m6.*t2.*t8.*t34.*4.0;
t1251 = Lz5.*Lzcm6.*dQ1.*dQ4.*m6.*t3.*t7.*t34.*4.0;
t1252 = Lz5.*Lzcm6.*dQ2.*dQ4.*m6.*t4.*t9.*t35.*4.0;
t1253 = Lz5.*Lzcm6.*dQ3.*dQ4.*m6.*t4.*t9.*t35.*4.0;
t1254 = Lz5.*Lzcm6.*dQ2.*dQ5.*m6.*t5.*t10.*t34.*4.0;
t1255 = Lz5.*Lzcm6.*dQ3.*dQ5.*m6.*t5.*t10.*t34.*4.0;
t1256 = t36.*t267.*2.0;
t1257 = t36.*t268.*2.0;
t1258 = t36.*t271.*2.0;
t1259 = t36.*t272.*2.0;
t1261 = t36.*t273.*2.0;
t1262 = t35.*t275.*2.0;
t1263 = t36.*t280.*2.0;
t1264 = t36.*t281.*2.0;
t1265 = t36.*t284.*2.0;
t1266 = t36.*t285.*2.0;
t1268 = t36.*t286.*2.0;
t1269 = t35.*t288.*2.0;
t1270 = Lxcm6.*Lz5.*dQ2.*dQ4.*m6.*t10.*t11.*t34.*4.0;
t1271 = Lxcm6.*Lz5.*dQ3.*dQ4.*m6.*t10.*t11.*t34.*4.0;
t1272 = Lxcm6.*Lz5.*dQ4.*dQ6.*m6.*t9.*t11.*t35.*2.0;
t1273 = Lxcm6.*Lzcm6.*dQ2.*dQ4.*m6.*t10.*t11.*t34.*4.0;
t1274 = Lxcm6.*Lzcm6.*dQ3.*dQ4.*m6.*t10.*t11.*t34.*4.0;
t1275 = Lxcm6.*Lzcm6.*dQ4.*dQ6.*m6.*t9.*t11.*t35.*2.0;
t1276 = t35.*t291.*2.0;
t1277 = t36.*t292.*2.0;
t1278 = t35.*t294.*2.0;
t1279 = t36.*t294.*2.0;
t1280 = t35.*t297.*2.0;
t1281 = t35.*t298.*2.0;
t1286 = -t1031;
t1287 = -t1032;
t1288 = -t1040;
t1289 = -t1042;
t1290 = -t1043;
t1291 = -t1044;
t1292 = -t1045;
t1293 = -t1047;
t1294 = -t1048;
t1295 = -t1049;
t1296 = -t1050;
t1297 = -t1051;
t1298 = -t1052;
t1299 = -t1053;
t1300 = -t1054;
t1301 = -t1055;
t1302 = -t1056;
t1303 = -t1057;
t1304 = -t1058;
t1305 = -t1059;
t1306 = -t841;
t1307 = -t842;
t1308 = -t1068;
t1309 = -t1069;
t1310 = -t1070;
t1311 = -t1071;
t1312 = -t846;
t1313 = -t847;
t1314 = -t1080;
t1315 = -t1081;
t1316 = -t1086;
t1317 = -t1087;
t1318 = -t1088;
t1319 = -t1089;
t1320 = -t1090;
t1321 = -t1091;
t1322 = -t1092;
t1323 = -t1100;
t1324 = -t1101;
t1325 = -t1102;
t1326 = -t1119;
t1327 = -t1121;
t1328 = -t1122;
t1329 = -t1123;
t1330 = -t1124;
t1331 = -t1125;
t1332 = -t1126;
t1333 = -t1128;
t1334 = -t1129;
t1335 = -t1130;
t1336 = -t1131;
t1337 = -t1132;
t1338 = -t1133;
t1339 = -t1134;
t1340 = -t1135;
t1341 = -t1136;
t1342 = -t1137;
t1343 = -t1138;
t1345 = -t1141;
t1346 = -t1142;
t1347 = -t1143;
t1348 = -t1144;
t1349 = -t1151;
t1350 = -t1152;
t1351 = -t1153;
t1352 = -t856;
t1353 = -t859;
t1354 = -t1156;
t1355 = -t1157;
t1356 = -t860;
t1357 = -t863;
t1358 = -t1160;
t1359 = -t1161;
t1360 = -t1162;
t1361 = -t1163;
t1362 = -t1164;
t1363 = -t1165;
t1364 = -t1166;
t1365 = -t1168;
t1366 = -t1171;
t1367 = -t1172;
t1368 = -t1176;
t1369 = -t864;
t1370 = -t1183;
t1371 = -t1184;
t1372 = -t865;
t1373 = -t866;
t1374 = -t1185;
t1375 = -t1186;
t1376 = -t867;
t1377 = -t1188;
t1378 = -t1189;
t1379 = -t1190;
t1387 = t35.*t36.*t65.*-2.0;
t1392 = t34.*t502;
t1393 = t34.*t503;
t1394 = Iyz6.*dQ1.*dQ6.*t2.*t3.*t6.*t9.*t35;
t1395 = t34.*t508;
t1396 = t34.*t509;
t1397 = Izy6.*dQ1.*dQ6.*t2.*t3.*t6.*t9.*t35;
t1398 = t35.*t515;
t1399 = t35.*t516;
t1400 = t34.*t520;
t1401 = t34.*t521;
t1402 = Ixz6.*dQ1.*dQ6.*t2.*t3.*t9.*t11.*t35;
t1403 = Ixz6.*dQ1.*dQ6.*t2.*t6.*t8.*t10.*t34;
t1404 = Ixz6.*dQ1.*dQ6.*t3.*t6.*t7.*t10.*t34;
t1405 = t35.*t528;
t1406 = t35.*t529;
t1407 = t34.*t533;
t1408 = t34.*t534;
t1409 = Izx6.*dQ1.*dQ6.*t2.*t3.*t9.*t11.*t35;
t1410 = Izx6.*dQ1.*dQ6.*t2.*t6.*t8.*t10.*t34;
t1411 = Izx6.*dQ1.*dQ6.*t3.*t6.*t7.*t10.*t34;
t1412 = Iyz6.*dQ1.*dQ6.*t2.*t8.*t10.*t11.*t34;
t1413 = Iyz6.*dQ1.*dQ6.*t3.*t7.*t10.*t11.*t34;
t1414 = Iyz6.*dQ1.*dQ6.*t6.*t7.*t8.*t9.*t35;
t1415 = Izy6.*dQ1.*dQ6.*t2.*t8.*t10.*t11.*t34;
t1416 = Izy6.*dQ1.*dQ6.*t3.*t7.*t10.*t11.*t34;
t1417 = Izy6.*dQ1.*dQ6.*t6.*t7.*t8.*t9.*t35;
t1418 = Ixz6.*dQ1.*dQ6.*t7.*t8.*t9.*t11.*t35;
t1419 = Izx6.*dQ1.*dQ6.*t7.*t8.*t9.*t11.*t35;
t1443 = Ixy6.*dQ4.*dQ5.*t6.*t9.*t11.*t35.*-2.0;
t1449 = Iyx6.*dQ4.*dQ5.*t6.*t9.*t11.*t35.*-2.0;
t1457 = dQ1.*dQ4.*m4.*t2.*t8.*t15.*t34.*2.0;
t1458 = dQ1.*dQ4.*m4.*t3.*t7.*t15.*t34.*2.0;
t1459 = t34.*t615;
t1460 = t34.*t616;
t1461 = t36.*t615;
t1462 = t36.*t616;
t1463 = dQ2.*dQ4.*m5.*t4.*t9.*t16.*t35.*2.0;
t1464 = dQ3.*dQ4.*m5.*t4.*t9.*t16.*t35.*2.0;
t1465 = dQ2.*dQ5.*m5.*t5.*t10.*t16.*t34.*2.0;
t1466 = dQ3.*dQ5.*m5.*t5.*t10.*t16.*t34.*2.0;
t1467 = dQ2.*dQ4.*m6.*t4.*t9.*t17.*t36.*2.0;
t1468 = dQ3.*dQ4.*m6.*t4.*t9.*t17.*t36.*2.0;
t1469 = dQ2.*dQ5.*m6.*t5.*t10.*t17.*t36.*2.0;
t1470 = dQ2.*dQ6.*m6.*t6.*t11.*t17.*t34.*2.0;
t1471 = dQ3.*dQ5.*m6.*t5.*t10.*t17.*t36.*2.0;
t1472 = dQ2.*dQ6.*m6.*t6.*t11.*t17.*t35.*2.0;
t1473 = dQ3.*dQ6.*m6.*t6.*t11.*t17.*t34.*2.0;
t1474 = dQ4.*dQ6.*m6.*t4.*t10.*t17.*t36.*2.0;
t1475 = dQ3.*dQ6.*m6.*t6.*t11.*t17.*t35.*2.0;
t1481 = dQ1.*dQ4.*m6.*t2.*t8.*t20.*t36.*2.0;
t1482 = dQ1.*dQ4.*m6.*t3.*t7.*t20.*t36.*2.0;
t1483 = dQ2.*dQ4.*m6.*t4.*t9.*t20.*t35.*2.0;
t1484 = dQ2.*dQ4.*m6.*t4.*t9.*t20.*t36.*2.0;
t1485 = dQ3.*dQ4.*m6.*t4.*t9.*t20.*t35.*2.0;
t1486 = dQ2.*dQ5.*m6.*t5.*t10.*t20.*t34.*2.0;
t1487 = dQ3.*dQ4.*m6.*t4.*t9.*t20.*t36.*2.0;
t1488 = dQ3.*dQ5.*m6.*t5.*t10.*t20.*t34.*2.0;
t1489 = dQ2.*dQ5.*m6.*t5.*t10.*t20.*t36.*2.0;
t1490 = dQ2.*dQ6.*m6.*t6.*t11.*t20.*t34.*2.0;
t1491 = dQ3.*dQ5.*m6.*t5.*t10.*t20.*t36.*2.0;
t1492 = dQ2.*dQ6.*m6.*t6.*t11.*t20.*t35.*2.0;
t1493 = dQ3.*dQ6.*m6.*t6.*t11.*t20.*t34.*2.0;
t1495 = dQ3.*dQ6.*m6.*t6.*t11.*t20.*t35.*2.0;
t1496 = dQ5.*dQ6.*m6.*t5.*t9.*t20.*t36.*2.0;
t1497 = dQ1.*dQ4.*m6.*t2.*t8.*t22.*t34.*2.0;
t1498 = dQ1.*dQ4.*m6.*t3.*t7.*t22.*t34.*2.0;
t1499 = dQ2.*dQ4.*m6.*t4.*t9.*t22.*t35.*2.0;
t1500 = dQ3.*dQ4.*m6.*t4.*t9.*t22.*t35.*2.0;
t1501 = dQ2.*dQ5.*m6.*t5.*t10.*t22.*t34.*2.0;
t1502 = dQ3.*dQ5.*m6.*t5.*t10.*t22.*t34.*2.0;
t1503 = dQ1.*dQ4.*m5.*t2.*t8.*t25.*t34.*2.0;
t1504 = dQ1.*dQ4.*m5.*t3.*t7.*t25.*t34.*2.0;
t1505 = dQ1.*dQ4.*m6.*t2.*t8.*t26.*t34.*2.0;
t1506 = dQ1.*dQ4.*m6.*t3.*t7.*t26.*t34.*2.0;
t1507 = dQ2.*dQ4.*m5.*t4.*t9.*t25.*t35.*2.0;
t1508 = dQ3.*dQ4.*m5.*t4.*t9.*t25.*t35.*2.0;
t1509 = dQ2.*dQ5.*m5.*t5.*t10.*t25.*t34.*2.0;
out1 = ft_3({Ixx2,Ixx3,Ixx4,Ixx5,Ixx6,Ixy3,Ixy4,Ixy5,Ixy6,Ixz2,Ixz3,Ixz4,Ixz5,Ixz6,Iyx3,Iyx4,Iyx5,Iyx6,Iyy4,Iyy5,Iyy6,Iyz3,Iyz4,Iyz5,Iyz6,Izx2,Izx3,Izx4,Izx5,Izx6,Izy3,Izy4,Izy5,Izy6,Izz2,Izz3,Izz4,Izz5,Izz6,Lx2,Lx3,Lxcm2,Lxcm3,Lxcm4,Lxcm5,Lxcm6,Lycm3,Lycm4,Lycm5,Lycm6,Lz4,Lz5,Lzcm2,Lzcm3,Lzcm4,Lzcm5,Lzcm6,dQ1,dQ2,dQ3,dQ4,dQ5,dQ6,m2,m3,m4,m5,m6,t10,t100,t1000,t101,t102,t103,t1032,t1033,t1034,t1035,t1036,t1037,t1038,t1039,t104,t1041,t1042,t1043,t1046,t1048,t1049,t105,t106,t1060,t1061,t1062,t1063,t1064,t1065,t1066,t1067,t107,t1072,t1073,t1074,t1075,t1076,t1077,t1078,t1079,t108,t109,t1093,t1094,t1095,t1096,t1097,t1098,t1099,t11,t110,t1100,t1101,t1103,t1104,t1105,t1106,t1107,t1108,t1109,t111,t1110,t1111,t1112,t1113,t1114,t1115,t1116,t1117,t1118,t112,t1120,t1121,t1122,t1127,t113,t1131,t1132,t1139,t114,t1140,t1141,t1142,t1145,t1146,t1147,t1148,t1149,t115,t1150,t1154,t1155,t1158,t1159,t116,t1167,t1169,t117,t1170,t1173,t1174,t1175,t1177,t1178,t1179,t118,t1180,t1181,t1182,t1183,t1185,t1187,t119,t1191,t1192,t1195,t1196,t12,t120,t1201,t1202,t1203,t1204,t121,t1213,t1214,t1215,t1216,t1217,t1218,t1219,t122,t1220,t1221,t1222,t1223,t1224,t1225,t1226,t1227,t1228,t1229,t123,t1230,t1231,t1232,t1233,t1234,t1235,t1236,t1237,t1238,t1239,t124,t1240,t1241,t1242,t1243,t1244,t1245,t1246,t1247,t1248,t1249,t125,t1250,t1251,t1252,t1253,t1254,t1255,t1256,t1257,t1258,t1259,t126,t1261,t1262,t1263,t1264,t1265,t1266,t1268,t1269,t127,t1270,t1271,t1272,t1273,t1274,t1275,t1276,t1277,t1278,t1279,t128,t1280,t1281,t1282,t1283,t1284,t1285,t1286,t1287,t1288,t1289,t129,t1290,t1291,t1292,t1293,t1294,t1295,t1296,t1297,t1298,t1299,t13,t130,t1300,t1301,t1302,t1303,t1304,t1305,t1306,t1307,t1308,t1309,t131,t1310,t1311,t1312,t1313,t1314,t1315,t1316,t1317,t1318,t1319,t132,t1320,t1321,t1322,t1323,t1324,t1325,t1326,t1327,t1328,t1329,t1330,t1331,t1332,t1333,t1334,t1335,t1336,t1337,t1338,t1339,t134,t1340,t1341,t1342,t1343,t1344,t1345,t1346,t1347,t1348,t1349,t1350,t1351,t1352,t1353,t1354,t1355,t1356,t1357,t1358,t1359,t136,t1360,t1361,t1362,t1363,t1364,t1365,t1366,t1367,t1368,t1369,t137,t1370,t1371,t1372,t1373,t1374,t1375,t1376,t1377,t1378,t1379,t138,t1380,t1387,t139,t1392,t1393,t1394,t1395,t1396,t1397,t1398,t1399,t14,t140,t1400,t1401,t1402,t1403,t1404,t1405,t1406,t1407,t1408,t1409,t141,t1410,t1411,t1412,t1413,t1414,t1415,t1416,t1417,t1418,t1419,t142,t143,t144,t1443,t1449,t145,t1457,t1458,t1459,t146,t1460,t1461,t1462,t1463,t1464,t1465,t1466,t1467,t1468,t1469,t147,t1470,t1471,t1472,t1473,t1474,t1475,t148,t1481,t1482,t1483,t1484,t1485,t1486,t1487,t1488,t1489,t149,t1490,t1491,t1492,t1493,t1495,t1496,t1497,t1498,t1499,t15,t150,t1500,t1501,t1502,t1503,t1504,t1505,t1506,t1507,t1508,t1509,t151,t152,t1522,t153,t154,t155,t156,t157,t158,t159,t16,t160,t161,t162,t1624,t1625,t1626,t1627,t1628,t1629,t163,t1630,t1631,t1632,t1633,t1634,t1635,t1636,t1637,t1638,t1639,t164,t165,t1666,t1667,t1668,t1669,t1670,t1671,t1672,t1673,t1674,t1675,t1676,t1677,t1678,t1679,t1680,t1681,t1682,t1683,t1684,t1685,t1686,t1687,t1688,t1689,t1690,t1691,t1692,t1693,t1694,t1695,t1696,t1697,t1698,t1699,t17,t170,t1700,t1701,t1702,t1703,t1704,t1705,t1706,t1707,t1708,t1709,t171,t1710,t1711,t1712,t1713,t1714,t1715,t1716,t1717,t1718,t1719,t172,t1720,t1721,t1722,t1723,t1724,t1725,t1726,t1727,t1728,t1729,t173,t1730,t1731,t1732,t1733,t1734,t1735,t1736,t1737,t1738,t1739,t174,t1740,t1741,t1742,t1743,t1744,t1745,t1746,t1747,t1748,t1749,t1750,t1751,t1752,t1753,t1754,t1755,t1756,t177,t178,t179,t18,t180,t183,t1836,t1837,t1838,t1839,t184,t1842,t1843,t1844,t1845,t185,t186,t1869,t187,t1870,t1879,t188,t1880,t1881,t1882,t1883,t19,t1923,t1924,t1925,t1926,t1927,t1928,t1929,t1930,t1931,t1932,t1933,t1934,t1935,t1936,t1937,t197,t198,t199,t2,t20,t200,t201,t202,t203,t2032,t2033,t204,t2046,t2047,t2048,t2051,t2054,t2055,t2056,t2057,t2058,t2059,t2060,t2061,t2062,t2063,t2064,t2068,t2069,t2070,t2071,t2072,t2073,t2074,t2075,t2076,t2077,t2078,t21,t2176,t2177,t2178,t2179,t2180,t2181,t2182,t2183,t2184,t2185,t2186,t2187,t2188,t2189,t2190,t2191,t2196,t2197,t22,t222,t2238,t2239,t2240,t2241,t2242,t2248,t2249,t225,t2250,t2251,t2252,t23,t2328,t2329,t2330,t2331,t2332,t2333,t2334,t2335,t237,t2377,t2378,t238,t239,t24,t240,t242,t243,t244,t245,t246,t25,t250,t251,t252,t253,t254,t258,t259,t26,t260,t263,t264,t265,t266,t267,t268,t269,t270,t271,t272,t273,t274,t276,t277,t278,t279,t280,t281,t282,t283,t284,t285,t286,t287,t289,t290,t292,t293,t294,t297,t298,t299,t3,t300,t301,t302,t303,t304,t305,t306,t307,t308,t309,t310,t311,t312,t313,t314,t315,t316,t317,t318,t319,t32,t320,t321,t322,t323,t324,t325,t326,t327,t328,t329,t33,t330,t331,t332,t333,t334,t335,t336,t337,t338,t339,t34,t340,t341,t342,t343,t344,t345,t346,t347,t348,t349,t35,t350,t351,t352,t355,t356,t357,t358,t359,t36,t360,t361,t362,t363,t364,t365,t366,t367,t368,t369,t37,t370,t371,t372,t373,t374,t375,t376,t377,t378,t379,t38,t380,t381,t382,t383,t384,t385,t386,t387,t388,t389,t39,t390,t391,t392,t393,t394,t395,t396,t397,t398,t4,t40,t402,t403,t404,t405,t406,t407,t41,t413,t414,t415,t416,t417,t418,t419,t42,t43,t430,t431,t432,t433,t434,t435,t436,t437,t438,t44,t442,t443,t444,t445,t446,t447,t45,t454,t455,t456,t457,t458,t459,t46,t460,t461,t462,t47,t48,t481,t482,t485,t486,t49,t498,t499,t5,t50,t500,t501,t502,t506,t507,t508,t51,t512,t514,t515,t516,t517,t518,t519,t52,t520,t527,t528,t529,t53,t530,t531,t532,t533,t539,t54,t540,t542,t543,t544,t546,t547,t548,t55,t550,t551,t552,t553,t554,t555,t556,t557,t558,t559,t56,t560,t561,t562,t563,t568,t569,t57,t570,t571,t572,t573,t574,t575,t576,t577,t578,t579,t58,t580,t581,t582,t583,t584,t585,t586,t587,t588,t589,t59,t590,t591,t592,t593,t594,t595,t596,t597,t598,t599,t6,t60,t600,t601,t602,t603,t604,t605,t606,t607,t608,t609,t61,t610,t611,t612,t613,t614,t615,t616,t617,t618,t619,t62,t620,t621,t622,t623,t624,t625,t626,t627,t628,t629,t63,t630,t631,t632,t633,t634,t635,t636,t637,t638,t639,t64,t640,t641,t642,t643,t648,t650,t651,t658,t659,t660,t661,t662,t663,t664,t665,t666,t669,t67,t670,t671,t674,t675,t676,t677,t678,t679,t68,t681,t684,t687,t688,t689,t69,t690,t691,t692,t694,t697,t7,t70,t71,t716,t717,t718,t719,t72,t720,t721,t722,t723,t724,t725,t728,t729,t73,t730,t731,t732,t733,t734,t735,t737,t738,t739,t74,t75,t757,t758,t759,t760,t761,t762,t763,t766,t767,t770,t771,t772,t773,t774,t775,t776,t777,t778,t779,t78,t780,t781,t782,t783,t784,t785,t786,t787,t788,t789,t79,t790,t791,t792,t793,t794,t795,t796,t797,t798,t799,t8,t80,t800,t801,t802,t803,t804,t805,t806,t807,t808,t809,t81,t810,t811,t812,t813,t814,t815,t816,t817,t818,t819,t82,t820,t821,t822,t823,t824,t825,t826,t827,t83,t831,t832,t833,t834,t839,t84,t840,t841,t842,t843,t844,t845,t846,t847,t848,t849,t85,t850,t851,t852,t853,t854,t855,t857,t858,t86,t861,t862,t864,t866,t868,t869,t87,t870,t871,t872,t873,t874,t875,t876,t877,t878,t879,t88,t880,t881,t882,t883,t884,t885,t886,t887,t888,t889,t89,t890,t891,t892,t893,t894,t895,t896,t897,t898,t899,t9,t90,t900,t901,t902,t903,t904,t905,t906,t907,t908,t909,t91,t910,t911,t912,t913,t914,t915,t916,t917,t918,t919,t92,t920,t921,t922,t923,t924,t925,t926,t927,t928,t929,t93,t930,t931,t932,t933,t934,t935,t936,t937,t938,t939,t94,t940,t941,t942,t943,t945,t948,t949,t95,t950,t951,t952,t953,t954,t955,t956,t957,t958,t959,t96,t960,t961,t962,t963,t968,t969,t97,t970,t971,t972,t973,t974,t975,t976,t977,t978,t979,t98,t980,t981,t982,t983,t984,t985,t986,t987,t99,t991,t992,t995,t996,t999});
end
function out1 = ft_3(ct)
[Ixx2,Ixx3,Ixx4,Ixx5,Ixx6,Ixy3,Ixy4,Ixy5,Ixy6,Ixz2,Ixz3,Ixz4,Ixz5,Ixz6,Iyx3,Iyx4,Iyx5,Iyx6,Iyy4,Iyy5,Iyy6,Iyz3,Iyz4,Iyz5,Iyz6,Izx2,Izx3,Izx4,Izx5,Izx6,Izy3,Izy4,Izy5,Izy6,Izz2,Izz3,Izz4,Izz5,Izz6,Lx2,Lx3,Lxcm2,Lxcm3,Lxcm4,Lxcm5,Lxcm6,Lycm3,Lycm4,Lycm5,Lycm6,Lz4,Lz5,Lzcm2,Lzcm3,Lzcm4,Lzcm5,Lzcm6,dQ1,dQ2,dQ3,dQ4,dQ5,dQ6,m2,m3,m4,m5,m6,t10,t100,t1000,t101,t102,t103,t1032,t1033,t1034,t1035,t1036,t1037,t1038,t1039,t104,t1041,t1042,t1043,t1046,t1048,t1049,t105,t106,t1060,t1061,t1062,t1063,t1064,t1065,t1066,t1067,t107,t1072,t1073,t1074,t1075,t1076,t1077,t1078,t1079,t108,t109,t1093,t1094,t1095,t1096,t1097,t1098,t1099,t11,t110,t1100,t1101,t1103,t1104,t1105,t1106,t1107,t1108,t1109,t111,t1110,t1111,t1112,t1113,t1114,t1115,t1116,t1117,t1118,t112,t1120,t1121,t1122,t1127,t113,t1131,t1132,t1139,t114,t1140,t1141,t1142,t1145,t1146,t1147,t1148,t1149,t115,t1150,t1154,t1155,t1158,t1159,t116,t1167,t1169,t117,t1170,t1173,t1174,t1175,t1177,t1178,t1179,t118,t1180,t1181,t1182,t1183,t1185,t1187,t119,t1191,t1192,t1195,t1196,t12,t120,t1201,t1202,t1203,t1204,t121,t1213,t1214,t1215,t1216,t1217,t1218,t1219,t122,t1220,t1221,t1222,t1223,t1224,t1225,t1226,t1227,t1228,t1229,t123,t1230,t1231,t1232,t1233,t1234,t1235,t1236,t1237,t1238,t1239,t124,t1240,t1241,t1242,t1243,t1244,t1245,t1246,t1247,t1248,t1249,t125,t1250,t1251,t1252,t1253,t1254,t1255,t1256,t1257,t1258,t1259,t126,t1261,t1262,t1263,t1264,t1265,t1266,t1268,t1269,t127,t1270,t1271,t1272,t1273,t1274,t1275,t1276,t1277,t1278,t1279,t128,t1280,t1281,t1282,t1283,t1284,t1285,t1286,t1287,t1288,t1289,t129,t1290,t1291,t1292,t1293,t1294,t1295,t1296,t1297,t1298,t1299,t13,t130,t1300,t1301,t1302,t1303,t1304,t1305,t1306,t1307,t1308,t1309,t131,t1310,t1311,t1312,t1313,t1314,t1315,t1316,t1317,t1318,t1319,t132,t1320,t1321,t1322,t1323,t1324,t1325,t1326,t1327,t1328,t1329,t1330,t1331,t1332,t1333,t1334,t1335,t1336,t1337,t1338,t1339,t134,t1340,t1341,t1342,t1343,t1344,t1345,t1346,t1347,t1348,t1349,t1350,t1351,t1352,t1353,t1354,t1355,t1356,t1357,t1358,t1359,t136,t1360,t1361,t1362,t1363,t1364,t1365,t1366,t1367,t1368,t1369,t137,t1370,t1371,t1372,t1373,t1374,t1375,t1376,t1377,t1378,t1379,t138,t1380,t1387,t139,t1392,t1393,t1394,t1395,t1396,t1397,t1398,t1399,t14,t140,t1400,t1401,t1402,t1403,t1404,t1405,t1406,t1407,t1408,t1409,t141,t1410,t1411,t1412,t1413,t1414,t1415,t1416,t1417,t1418,t1419,t142,t143,t144,t1443,t1449,t145,t1457,t1458,t1459,t146,t1460,t1461,t1462,t1463,t1464,t1465,t1466,t1467,t1468,t1469,t147,t1470,t1471,t1472,t1473,t1474,t1475,t148,t1481,t1482,t1483,t1484,t1485,t1486,t1487,t1488,t1489,t149,t1490,t1491,t1492,t1493,t1495,t1496,t1497,t1498,t1499,t15,t150,t1500,t1501,t1502,t1503,t1504,t1505,t1506,t1507,t1508,t1509,t151,t152,t1522,t153,t154,t155,t156,t157,t158,t159,t16,t160,t161,t162,t1624,t1625,t1626,t1627,t1628,t1629,t163,t1630,t1631,t1632,t1633,t1634,t1635,t1636,t1637,t1638,t1639,t164,t165,t1666,t1667,t1668,t1669,t1670,t1671,t1672,t1673,t1674,t1675,t1676,t1677,t1678,t1679,t1680,t1681,t1682,t1683,t1684,t1685,t1686,t1687,t1688,t1689,t1690,t1691,t1692,t1693,t1694,t1695,t1696,t1697,t1698,t1699,t17,t170,t1700,t1701,t1702,t1703,t1704,t1705,t1706,t1707,t1708,t1709,t171,t1710,t1711,t1712,t1713,t1714,t1715,t1716,t1717,t1718,t1719,t172,t1720,t1721,t1722,t1723,t1724,t1725,t1726,t1727,t1728,t1729,t173,t1730,t1731,t1732,t1733,t1734,t1735,t1736,t1737,t1738,t1739,t174,t1740,t1741,t1742,t1743,t1744,t1745,t1746,t1747,t1748,t1749,t1750,t1751,t1752,t1753,t1754,t1755,t1756,t177,t178,t179,t18,t180,t183,t1836,t1837,t1838,t1839,t184,t1842,t1843,t1844,t1845,t185,t186,t1869,t187,t1870,t1879,t188,t1880,t1881,t1882,t1883,t19,t1923,t1924,t1925,t1926,t1927,t1928,t1929,t1930,t1931,t1932,t1933,t1934,t1935,t1936,t1937,t197,t198,t199,t2,t20,t200,t201,t202,t203,t2032,t2033,t204,t2046,t2047,t2048,t2051,t2054,t2055,t2056,t2057,t2058,t2059,t2060,t2061,t2062,t2063,t2064,t2068,t2069,t2070,t2071,t2072,t2073,t2074,t2075,t2076,t2077,t2078,t21,t2176,t2177,t2178,t2179,t2180,t2181,t2182,t2183,t2184,t2185,t2186,t2187,t2188,t2189,t2190,t2191,t2196,t2197,t22,t222,t2238,t2239,t2240,t2241,t2242,t2248,t2249,t225,t2250,t2251,t2252,t23,t2328,t2329,t2330,t2331,t2332,t2333,t2334,t2335,t237,t2377,t2378,t238,t239,t24,t240,t242,t243,t244,t245,t246,t25,t250,t251,t252,t253,t254,t258,t259,t26,t260,t263,t264,t265,t266,t267,t268,t269,t270,t271,t272,t273,t274,t276,t277,t278,t279,t280,t281,t282,t283,t284,t285,t286,t287,t289,t290,t292,t293,t294,t297,t298,t299,t3,t300,t301,t302,t303,t304,t305,t306,t307,t308,t309,t310,t311,t312,t313,t314,t315,t316,t317,t318,t319,t32,t320,t321,t322,t323,t324,t325,t326,t327,t328,t329,t33,t330,t331,t332,t333,t334,t335,t336,t337,t338,t339,t34,t340,t341,t342,t343,t344,t345,t346,t347,t348,t349,t35,t350,t351,t352,t355,t356,t357,t358,t359,t36,t360,t361,t362,t363,t364,t365,t366,t367,t368,t369,t37,t370,t371,t372,t373,t374,t375,t376,t377,t378,t379,t38,t380,t381,t382,t383,t384,t385,t386,t387,t388,t389,t39,t390,t391,t392,t393,t394,t395,t396,t397,t398,t4,t40,t402,t403,t404,t405,t406,t407,t41,t413,t414,t415,t416,t417,t418,t419,t42,t43,t430,t431,t432,t433,t434,t435,t436,t437,t438,t44,t442,t443,t444,t445,t446,t447,t45,t454,t455,t456,t457,t458,t459,t46,t460,t461,t462,t47,t48,t481,t482,t485,t486,t49,t498,t499,t5,t50,t500,t501,t502,t506,t507,t508,t51,t512,t514,t515,t516,t517,t518,t519,t52,t520,t527,t528,t529,t53,t530,t531,t532,t533,t539,t54,t540,t542,t543,t544,t546,t547,t548,t55,t550,t551,t552,t553,t554,t555,t556,t557,t558,t559,t56,t560,t561,t562,t563,t568,t569,t57,t570,t571,t572,t573,t574,t575,t576,t577,t578,t579,t58,t580,t581,t582,t583,t584,t585,t586,t587,t588,t589,t59,t590,t591,t592,t593,t594,t595,t596,t597,t598,t599,t6,t60,t600,t601,t602,t603,t604,t605,t606,t607,t608,t609,t61,t610,t611,t612,t613,t614,t615,t616,t617,t618,t619,t62,t620,t621,t622,t623,t624,t625,t626,t627,t628,t629,t63,t630,t631,t632,t633,t634,t635,t636,t637,t638,t639,t64,t640,t641,t642,t643,t648,t650,t651,t658,t659,t660,t661,t662,t663,t664,t665,t666,t669,t67,t670,t671,t674,t675,t676,t677,t678,t679,t68,t681,t684,t687,t688,t689,t69,t690,t691,t692,t694,t697,t7,t70,t71,t716,t717,t718,t719,t72,t720,t721,t722,t723,t724,t725,t728,t729,t73,t730,t731,t732,t733,t734,t735,t737,t738,t739,t74,t75,t757,t758,t759,t760,t761,t762,t763,t766,t767,t770,t771,t772,t773,t774,t775,t776,t777,t778,t779,t78,t780,t781,t782,t783,t784,t785,t786,t787,t788,t789,t79,t790,t791,t792,t793,t794,t795,t796,t797,t798,t799,t8,t80,t800,t801,t802,t803,t804,t805,t806,t807,t808,t809,t81,t810,t811,t812,t813,t814,t815,t816,t817,t818,t819,t82,t820,t821,t822,t823,t824,t825,t826,t827,t83,t831,t832,t833,t834,t839,t84,t840,t841,t842,t843,t844,t845,t846,t847,t848,t849,t85,t850,t851,t852,t853,t854,t855,t857,t858,t86,t861,t862,t864,t866,t868,t869,t87,t870,t871,t872,t873,t874,t875,t876,t877,t878,t879,t88,t880,t881,t882,t883,t884,t885,t886,t887,t888,t889,t89,t890,t891,t892,t893,t894,t895,t896,t897,t898,t899,t9,t90,t900,t901,t902,t903,t904,t905,t906,t907,t908,t909,t91,t910,t911,t912,t913,t914,t915,t916,t917,t918,t919,t92,t920,t921,t922,t923,t924,t925,t926,t927,t928,t929,t93,t930,t931,t932,t933,t934,t935,t936,t937,t938,t939,t94,t940,t941,t942,t943,t945,t948,t949,t95,t950,t951,t952,t953,t954,t955,t956,t957,t958,t959,t96,t960,t961,t962,t963,t968,t969,t97,t970,t971,t972,t973,t974,t975,t976,t977,t978,t979,t98,t980,t981,t982,t983,t984,t985,t986,t987,t99,t991,t992,t995,t996,t999] = ct{:};
t1510 = dQ2.*dQ4.*m6.*t4.*t9.*t26.*t35.*2.0;
t1511 = dQ3.*dQ5.*m5.*t5.*t10.*t25.*t34.*2.0;
t1512 = dQ3.*dQ4.*m6.*t4.*t9.*t26.*t35.*2.0;
t1513 = dQ2.*dQ5.*m6.*t5.*t10.*t26.*t34.*2.0;
t1514 = dQ3.*dQ5.*m6.*t5.*t10.*t26.*t34.*2.0;
t1518 = -t999;
t1519 = -t1000;
t1520 = -t1282;
t1521 = -t1284;
t1527 = t34.*t35.*t128.*2.0;
t1528 = t34.*t35.*t129.*2.0;
t1537 = t34.*t35.*t138.*2.0;
t1538 = t34.*t35.*t139.*2.0;
t1555 = -t1380;
t1556 = t35.*t485.*2.0;
t1557 = t35.*t486.*2.0;
t1558 = Lxcm5.*Lzcm5.*dQ1.*dQ4.*m5.*t2.*t3.*t4.*t35.*4.0;
t1559 = t36.*t498.*2.0;
t1560 = t36.*t499.*2.0;
t1561 = t35.*t501.*2.0;
t1562 = t35.*t507.*2.0;
t1565 = t34.*t665;
t1566 = t34.*t666;
t1569 = Lz5.*Lzcm6.*dQ1.*dQ5.*m6.*t2.*t3.*t9.*t35.*4.0;
t1570 = t36.*t514.*2.0;
t1573 = t36.*t515.*2.0;
t1574 = t36.*t516.*2.0;
t1575 = t35.*t676;
t1576 = t35.*t677;
t1577 = t34.*t678;
t1578 = t34.*t679;
t1579 = Ixz5.*dQ1.*dQ4.*t2.*t5.*t8.*t10.*t34.*2.0;
t1580 = Ixz5.*dQ1.*dQ4.*t3.*t5.*t7.*t10.*t34.*2.0;
t1581 = t35.*t517.*2.0;
t1582 = t35.*t518.*2.0;
t1583 = t35.*t519.*2.0;
t1584 = t36.*t527.*2.0;
t1587 = t36.*t528.*2.0;
t1588 = t36.*t529.*2.0;
t1589 = t35.*t689;
t1590 = t35.*t690;
t1591 = t34.*t691;
t1592 = t34.*t692;
t1593 = Izx5.*dQ1.*dQ4.*t2.*t5.*t8.*t10.*t34.*2.0;
t1594 = Izx5.*dQ1.*dQ4.*t3.*t5.*t7.*t10.*t34.*2.0;
t1595 = t35.*t530.*2.0;
t1596 = t35.*t531.*2.0;
t1597 = t35.*t532.*2.0;
t1600 = t34.*t722;
t1601 = t34.*t723;
t1602 = Lxcm6.*Lycm6.*dQ1.*dQ5.*m6.*t2.*t8.*t10.*t36.*4.0;
t1603 = Lxcm6.*Lycm6.*dQ1.*dQ5.*m6.*t3.*t7.*t10.*t36.*4.0;
t1604 = Lxcm6.*Lycm6.*dQ2.*dQ5.*m6.*t4.*t9.*t10.*t36.*4.0;
t1605 = Lxcm6.*Lycm6.*dQ3.*dQ5.*m6.*t4.*t9.*t10.*t36.*4.0;
t1607 = Lxcm6.*Lycm6.*dQ4.*dQ6.*m6.*t5.*t9.*t10.*t36.*4.0;
t1610 = Lxcm5.*Lzcm5.*dQ1.*dQ4.*m5.*t4.*t7.*t8.*t35.*4.0;
t1613 = t36.*t539.*2.0;
t1614 = t36.*t540.*2.0;
t1615 = t35.*t542.*2.0;
t1616 = t35.*t546.*2.0;
t1617 = Lz5.*Lzcm6.*dQ1.*dQ5.*m6.*t7.*t8.*t9.*t35.*4.0;
t1618 = t36.*t551.*2.0;
t1619 = t36.*t553.*2.0;
t1640 = dQ1.*dQ4.*m6.*t2.*t8.*t17.*t34.*-2.0;
t1641 = dQ1.*dQ4.*m6.*t3.*t7.*t17.*t34.*-2.0;
t1642 = dQ1.*dQ4.*m6.*t2.*t8.*t17.*t36.*-2.0;
t1643 = dQ1.*dQ4.*m6.*t3.*t7.*t17.*t36.*-2.0;
t1652 = dQ5.*dQ6.*m6.*t5.*t9.*t17.*t36.*-2.0;
t1653 = dQ1.*dQ4.*m4.*t2.*t8.*t18.*t34.*-2.0;
t1654 = dQ1.*dQ4.*m4.*t3.*t7.*t18.*t34.*-2.0;
t1655 = dQ1.*dQ4.*m5.*t2.*t8.*t19.*t34.*-2.0;
t1656 = dQ1.*dQ4.*m5.*t3.*t7.*t19.*t34.*-2.0;
t1664 = dQ4.*dQ6.*m6.*t4.*t10.*t20.*t36.*-2.0;
t1757 = Lxcm6.*Lycm6.*dQ2.*dQ4.*m6.*t5.*t34.*t36.*8.0;
t1758 = Lxcm6.*Lycm6.*dQ3.*dQ4.*m6.*t5.*t34.*t36.*8.0;
t1761 = t34.*t36.*t130.*-2.0;
t1762 = t34.*t36.*t131.*-2.0;
t1765 = Iyy6.*dQ2.*dQ4.*t4.*t9.*t35.*t36.*-2.0;
t1766 = Iyy6.*dQ3.*dQ4.*t4.*t9.*t35.*t36.*-2.0;
t1767 = Iyy6.*dQ2.*dQ5.*t5.*t10.*t34.*t36.*-2.0;
t1768 = Iyy6.*dQ3.*dQ5.*t5.*t10.*t34.*t36.*-2.0;
t1769 = Iyy6.*dQ2.*dQ6.*t6.*t11.*t34.*t35.*-2.0;
t1770 = Iyy6.*dQ3.*dQ6.*t6.*t11.*t34.*t35.*-2.0;
t1771 = Lycm6.*Lz5.*dQ2.*dQ5.*m6.*t11.*t34.*t35.*-4.0;
t1772 = Lycm6.*Lz5.*dQ3.*dQ5.*m6.*t11.*t34.*t35.*-4.0;
t1773 = Lycm6.*Lzcm6.*dQ2.*dQ5.*m6.*t11.*t34.*t35.*-4.0;
t1774 = Lycm6.*Lzcm6.*dQ3.*dQ5.*m6.*t11.*t34.*t35.*-4.0;
t1781 = Lycm6.*Lz5.*dQ2.*dQ6.*m6.*t5.*t6.*t10.*t34.*-2.0;
t1782 = Lycm6.*Lz5.*dQ3.*dQ6.*m6.*t5.*t6.*t10.*t34.*-2.0;
t1783 = Lycm6.*Lzcm6.*dQ2.*dQ6.*m6.*t5.*t6.*t10.*t34.*-2.0;
t1784 = Lycm6.*Lzcm6.*dQ3.*dQ6.*m6.*t5.*t6.*t10.*t34.*-2.0;
t1787 = Ixy6.*dQ1.*dQ4.*t2.*t6.*t8.*t11.*t34.*-2.0;
t1788 = Ixy6.*dQ1.*dQ4.*t3.*t6.*t7.*t11.*t34.*-2.0;
t1792 = Iyx6.*dQ1.*dQ4.*t2.*t6.*t8.*t11.*t34.*-2.0;
t1793 = Iyx6.*dQ1.*dQ4.*t3.*t6.*t7.*t11.*t34.*-2.0;
t1796 = Lxcm5.*Lycm5.*dQ1.*dQ5.*m5.*t2.*t8.*t10.*t34.*-2.0;
t1797 = Lxcm5.*Lycm5.*dQ1.*dQ5.*m5.*t3.*t7.*t10.*t34.*-2.0;
t1798 = Lxcm6.*Lycm6.*dQ4.*dQ5.*m6.*t6.*t9.*t11.*t35.*-4.0;
t1800 = Lxcm6.*Lz5.*dQ2.*dQ6.*m6.*t5.*t10.*t11.*t34.*-2.0;
t1801 = Lxcm6.*Lz5.*dQ3.*dQ6.*m6.*t5.*t10.*t11.*t34.*-2.0;
t1802 = Lxcm6.*Lzcm6.*dQ2.*dQ6.*m6.*t5.*t10.*t11.*t34.*-2.0;
t1803 = Lxcm6.*Lzcm6.*dQ3.*dQ6.*m6.*t5.*t10.*t11.*t34.*-2.0;
t1804 = t35.*t937;
t1805 = dQ1.*dQ5.*m6.*t2.*t3.*t9.*t17.*t36.*2.0;
t1808 = t36.*t938;
t1809 = t36.*t939;
t1810 = dQ2.*dQ4.*m6.*t5.*t6.*t11.*t17.*t34.*4.0;
t1811 = dQ2.*dQ6.*m6.*t4.*t5.*t9.*t17.*t36.*4.0;
t1812 = dQ3.*dQ4.*m6.*t5.*t6.*t11.*t17.*t34.*4.0;
t1813 = dQ3.*dQ6.*m6.*t4.*t5.*t9.*t17.*t36.*4.0;
t1814 = t35.*t945;
t1815 = t36.*t945;
t1816 = dQ1.*dQ6.*m6.*t2.*t5.*t8.*t20.*t34.*2.0;
t1817 = dQ1.*dQ6.*m6.*t3.*t5.*t7.*t20.*t34.*2.0;
t1818 = dQ1.*dQ6.*m6.*t2.*t5.*t8.*t20.*t36.*2.0;
t1819 = dQ1.*dQ6.*m6.*t3.*t5.*t7.*t20.*t36.*2.0;
t1820 = dQ2.*dQ4.*m6.*t5.*t6.*t11.*t20.*t34.*4.0;
t1821 = dQ2.*dQ6.*m6.*t4.*t5.*t9.*t20.*t36.*4.0;
t1822 = dQ3.*dQ4.*m6.*t5.*t6.*t11.*t20.*t34.*4.0;
t1823 = dQ3.*dQ6.*m6.*t4.*t5.*t9.*t20.*t36.*4.0;
t1824 = dQ1.*dQ5.*m6.*t2.*t3.*t9.*t22.*t35.*2.0;
t1825 = dQ1.*dQ5.*m5.*t2.*t3.*t9.*t25.*t35.*2.0;
t1826 = dQ1.*dQ5.*m6.*t2.*t3.*t9.*t26.*t35.*2.0;
t1847 = dQ1.*dQ5.*m6.*t7.*t8.*t9.*t17.*t36.*2.0;
t1848 = t35.*t963;
t1850 = dQ1.*dQ5.*m6.*t7.*t8.*t9.*t22.*t35.*2.0;
t1851 = dQ1.*dQ5.*m5.*t7.*t8.*t9.*t25.*t35.*2.0;
t1852 = dQ1.*dQ5.*m6.*t7.*t8.*t9.*t26.*t35.*2.0;
t1857 = -t1624;
t1858 = -t1625;
t1859 = -t1626;
t1860 = -t1635;
t1861 = -t1636;
t1862 = -t1638;
t1863 = -t1666;
t1864 = -t1667;
t1865 = -t1668;
t1866 = -t1669;
t1867 = -t1670;
t1868 = -t1671;
t1871 = -t1681;
t1872 = -t1682;
t1873 = -t1685;
t1874 = -t1686;
t1875 = -t1689;
t1876 = -t1690;
t1877 = -t1692;
t1878 = -t1693;
t1884 = -t1701;
t1885 = -t1702;
t1886 = -t1703;
t1887 = -t1704;
t1888 = -t1705;
t1889 = -t1706;
t1890 = -t1707;
t1891 = -t1708;
t1892 = -t1709;
t1893 = -t1710;
t1894 = -t1711;
t1895 = -t1712;
t1896 = -t1713;
t1897 = -t1714;
t1898 = -t1715;
t1899 = -t1716;
t1900 = -t1717;
t1901 = -t1718;
t1902 = -t1719;
t1903 = -t1720;
t1904 = -t1723;
t1905 = -t1724;
t1906 = -t1727;
t1907 = -t1728;
t1908 = -t1729;
t1909 = -t1732;
t1910 = -t1737;
t1911 = -t1738;
t1912 = -t1739;
t1913 = -t1741;
t1914 = -t1742;
t1915 = -t1743;
t1916 = -t1746;
t1917 = -t1747;
t1918 = -t1748;
t1919 = -t1749;
t1920 = -t1750;
t1921 = -t1751;
t1922 = -t1752;
t1938 = -t1753;
t1941 = Lxcm6.*Lz5.*dQ1.*dQ4.*m6.*t2.*t3.*t4.*t6.*t35.*4.0;
t1942 = Lxcm6.*Lzcm6.*dQ1.*dQ4.*m6.*t2.*t3.*t4.*t6.*t35.*4.0;
t1943 = Ixx6.*dQ1.*dQ4.*t2.*t3.*t4.*t5.*t10.*t36.*2.0;
t1944 = t36.*t1032;
t1945 = t34.*t1042;
t1946 = t34.*t1043;
t1947 = Lycm6.*Lz5.*dQ1.*dQ4.*m6.*t2.*t3.*t4.*t11.*t35.*4.0;
t1948 = Lycm6.*Lz5.*dQ1.*dQ6.*m6.*t2.*t3.*t6.*t9.*t35.*2.0;
t1949 = t34.*t1048;
t1950 = t34.*t1049;
t1951 = Lycm6.*Lzcm6.*dQ1.*dQ4.*m6.*t2.*t3.*t4.*t11.*t35.*4.0;
t1952 = Lycm6.*Lzcm6.*dQ1.*dQ6.*m6.*t2.*t3.*t6.*t9.*t35.*2.0;
t1953 = Ixy6.*dQ1.*dQ4.*t2.*t4.*t5.*t8.*t9.*t36.*4.0;
t1954 = Ixy6.*dQ1.*dQ4.*t3.*t4.*t5.*t7.*t9.*t36.*4.0;
t1956 = t36.*t839.*2.0;
t1957 = Ixy6.*dQ1.*dQ6.*t2.*t5.*t6.*t8.*t11.*t34.*4.0;
t1958 = Ixy6.*dQ1.*dQ6.*t3.*t5.*t6.*t7.*t11.*t34.*4.0;
t1959 = Ixz6.*dQ1.*dQ4.*t2.*t5.*t6.*t8.*t10.*t34.*2.0;
t1960 = Ixz6.*dQ1.*dQ4.*t3.*t5.*t6.*t7.*t10.*t34.*2.0;
t1961 = t35.*t841.*2.0;
t1962 = t35.*t842.*2.0;
t1963 = Iyx6.*dQ1.*dQ4.*t2.*t4.*t5.*t8.*t9.*t36.*4.0;
t1964 = Iyx6.*dQ1.*dQ4.*t3.*t4.*t5.*t7.*t9.*t36.*4.0;
t1966 = t36.*t844.*2.0;
t1967 = Iyx6.*dQ1.*dQ6.*t2.*t5.*t6.*t8.*t11.*t34.*4.0;
t1968 = Iyx6.*dQ1.*dQ6.*t3.*t5.*t6.*t7.*t11.*t34.*4.0;
t1969 = Izx6.*dQ1.*dQ4.*t2.*t5.*t6.*t8.*t10.*t34.*2.0;
t1970 = Izx6.*dQ1.*dQ4.*t3.*t5.*t6.*t7.*t10.*t34.*2.0;
t1971 = t35.*t846.*2.0;
t1972 = t35.*t847.*2.0;
t1973 = dQ4.*dQ5.*m6.*t9.*t20.*t35.*t36.*-2.0;
t1974 = t35.*t1094;
t1975 = t35.*t1095;
t1976 = Lxcm6.*Lycm6.*dQ1.*dQ4.*m6.*t2.*t3.*t9.*t10.*t36.*4.0;
t1979 = Lxcm6.*Lycm6.*dQ1.*dQ6.*m6.*t2.*t4.*t8.*t9.*t36.*4.0;
t1980 = Lxcm6.*Lycm6.*dQ1.*dQ6.*m6.*t3.*t4.*t7.*t9.*t36.*4.0;
t1981 = t35.*t1098;
t1982 = t35.*t1099;
t1983 = t34.*t1100;
t1984 = t34.*t1101;
t1985 = t34.*t1121;
t1986 = t34.*t1122;
t1987 = Lxcm6.*Lz5.*dQ1.*dQ4.*m6.*t4.*t6.*t7.*t8.*t35.*4.0;
t1988 = Lxcm6.*Lz5.*dQ1.*dQ6.*m6.*t2.*t3.*t9.*t11.*t35.*2.0;
t1989 = Lxcm6.*Lz5.*dQ1.*dQ6.*m6.*t2.*t6.*t8.*t10.*t34.*2.0;
t1990 = Lxcm6.*Lz5.*dQ1.*dQ6.*m6.*t3.*t6.*t7.*t10.*t34.*2.0;
t1991 = Lxcm5.*Lzcm5.*dQ1.*dQ4.*m5.*t2.*t5.*t8.*t10.*t34.*4.0;
t1992 = Lxcm5.*Lzcm5.*dQ1.*dQ4.*m5.*t3.*t5.*t7.*t10.*t34.*4.0;
t1993 = Lxcm5.*Lzcm5.*dQ1.*dQ5.*m5.*t2.*t4.*t8.*t9.*t35.*4.0;
t1994 = Lxcm5.*Lzcm5.*dQ1.*dQ5.*m5.*t3.*t4.*t7.*t9.*t35.*4.0;
t1995 = t34.*t1131;
t1996 = t34.*t1132;
t1997 = Lxcm6.*Lzcm6.*dQ1.*dQ4.*m6.*t4.*t6.*t7.*t8.*t35.*4.0;
t1998 = Lxcm6.*Lzcm6.*dQ1.*dQ6.*m6.*t2.*t3.*t9.*t11.*t35.*2.0;
t1999 = Lxcm6.*Lzcm6.*dQ1.*dQ6.*m6.*t2.*t6.*t8.*t10.*t34.*2.0;
t2000 = Lxcm6.*Lzcm6.*dQ1.*dQ6.*m6.*t3.*t6.*t7.*t10.*t34.*2.0;
t2001 = Ixx6.*dQ1.*dQ4.*t4.*t5.*t7.*t8.*t10.*t36.*2.0;
t2002 = t34.*t1141;
t2003 = t34.*t1142;
t2007 = Iyz6.*dQ1.*dQ4.*t2.*t5.*t8.*t10.*t11.*t34.*2.0;
t2008 = Iyz6.*dQ1.*dQ4.*t3.*t5.*t7.*t10.*t11.*t34.*2.0;
t2009 = t35.*t857.*2.0;
t2010 = t35.*t858.*2.0;
t2011 = Izy6.*dQ1.*dQ4.*t2.*t5.*t8.*t10.*t11.*t34.*2.0;
t2012 = Izy6.*dQ1.*dQ4.*t3.*t5.*t7.*t10.*t11.*t34.*2.0;
t2013 = t35.*t861.*2.0;
t2014 = t35.*t862.*2.0;
t2015 = Lycm6.*Lz5.*dQ1.*dQ4.*m6.*t4.*t7.*t8.*t11.*t35.*4.0;
t2016 = Lycm6.*Lz5.*dQ1.*dQ6.*m6.*t2.*t8.*t10.*t11.*t34.*2.0;
t2017 = Lycm6.*Lz5.*dQ1.*dQ6.*m6.*t3.*t7.*t10.*t11.*t34.*2.0;
t2018 = Lycm6.*Lz5.*dQ1.*dQ6.*m6.*t6.*t7.*t8.*t9.*t35.*2.0;
t2019 = Lycm6.*Lzcm6.*dQ1.*dQ4.*m6.*t4.*t7.*t8.*t11.*t35.*4.0;
t2020 = Lycm6.*Lzcm6.*dQ1.*dQ6.*m6.*t2.*t8.*t10.*t11.*t34.*2.0;
t2021 = Lycm6.*Lzcm6.*dQ1.*dQ6.*m6.*t3.*t7.*t10.*t11.*t34.*2.0;
t2022 = Lycm6.*Lzcm6.*dQ1.*dQ6.*m6.*t6.*t7.*t8.*t9.*t35.*2.0;
t2023 = t35.*t1183;
t2024 = t36.*t864.*2.0;
t2025 = t35.*t1185;
t2026 = t36.*t866.*2.0;
t2027 = Lxcm6.*Lycm6.*dQ1.*dQ4.*m6.*t7.*t8.*t9.*t10.*t36.*4.0;
t2028 = Lxcm6.*Lz5.*dQ1.*dQ6.*m6.*t7.*t8.*t9.*t11.*t35.*2.0;
t2029 = Lxcm6.*Lzcm6.*dQ1.*dQ6.*m6.*t7.*t8.*t9.*t11.*t35.*2.0;
t2035 = dQ1.*dQ6.*m6.*t2.*t5.*t8.*t17.*t34.*-2.0;
t2036 = dQ1.*dQ6.*m6.*t3.*t5.*t7.*t17.*t34.*-2.0;
t2037 = dQ1.*dQ6.*m6.*t2.*t5.*t8.*t17.*t36.*-2.0;
t2038 = dQ1.*dQ6.*m6.*t3.*t5.*t7.*t17.*t36.*-2.0;
t2049 = t4.*t5.*t6.*t9.*t11.*t130.*4.0;
t2050 = t4.*t5.*t6.*t9.*t11.*t131.*4.0;
t2052 = t4.*t5.*t6.*t9.*t11.*t138.*4.0;
t2053 = t4.*t5.*t6.*t9.*t11.*t139.*4.0;
t2065 = dQ1.*dQ5.*m5.*t7.*t8.*t9.*t16.*t35.*-2.0;
t2066 = dQ1.*dQ5.*m6.*t7.*t8.*t9.*t20.*t35.*-2.0;
t2067 = dQ1.*dQ5.*m6.*t7.*t8.*t9.*t20.*t36.*-2.0;
t2080 = t34.*t36.*t239.*4.0;
t2081 = t34.*t36.*t240.*4.0;
t2083 = t34.*t36.*t243.*4.0;
t2084 = t34.*t36.*t244.*4.0;
t2091 = -t1881;
t2092 = -t1882;
t2093 = -t1883;
t2096 = -t1923;
t2097 = -t1928;
t2098 = -t1929;
t2099 = -t1930;
t2100 = -t1931;
t2101 = -t1932;
t2102 = -t1933;
t2108 = Ixy6.*dQ1.*dQ5.*t2.*t3.*t6.*t9.*t11.*t35.*-2.0;
t2114 = Iyx6.*dQ1.*dQ5.*t2.*t3.*t6.*t9.*t11.*t35.*-2.0;
t2119 = Lxcm6.*Lycm6.*dQ1.*dQ4.*m6.*t2.*t6.*t8.*t11.*t34.*-4.0;
t2120 = Lxcm6.*Lycm6.*dQ1.*dQ4.*m6.*t3.*t6.*t7.*t11.*t34.*-4.0;
t2123 = dQ1.*dQ6.*m6.*t2.*t3.*t4.*t10.*t17.*t36.*2.0;
t2125 = Iyy6.*dQ1.*dQ4.*t4.*t5.*t7.*t8.*t10.*t36.*-2.0;
t2126 = Iyy6.*dQ1.*dQ5.*t2.*t6.*t8.*t10.*t11.*t34.*-2.0;
t2127 = Iyy6.*dQ1.*dQ5.*t3.*t6.*t7.*t10.*t11.*t34.*-2.0;
t2146 = dQ1.*dQ6.*m6.*t4.*t7.*t8.*t10.*t17.*t36.*2.0;
t2147 = t36.*t1380;
t2148 = Lxcm6.*Lycm6.*dQ2.*dQ6.*m6.*t34.*t35.*t36.*-4.0;
t2149 = Lxcm6.*Lycm6.*dQ3.*dQ6.*m6.*t34.*t35.*t36.*-4.0;
t2150 = -t2032;
t2151 = -t2033;
t2152 = -t2046;
t2155 = -t2054;
t2156 = -t1836;
t2157 = -t1837;
t2158 = -t1838;
t2159 = -t1839;
t2160 = -t2055;
t2161 = -t2056;
t2162 = -t2057;
t2163 = -t2058;
t2164 = -t2059;
t2165 = -t2060;
t2166 = -t1842;
t2167 = -t1843;
t2168 = -t1844;
t2169 = -t1845;
t2170 = -t2069;
t2171 = -t2070;
t2172 = -t2071;
t2173 = -t2072;
t2174 = -t2073;
t2175 = -t2074;
t2192 = -t2075;
t2193 = t35.*t36.*t238.*-2.0;
t2198 = Lz5.*Lzcm6.*dQ1.*dQ4.*m6.*t2.*t8.*t34.*t35.*-4.0;
t2199 = Lz5.*Lzcm6.*dQ1.*dQ4.*m6.*t3.*t7.*t34.*t35.*-4.0;
t2204 = dQ1.*dQ4.*m5.*t2.*t8.*t16.*t34.*t35.*2.0;
t2205 = dQ1.*dQ4.*m5.*t3.*t7.*t16.*t34.*t35.*2.0;
t2214 = dQ1.*dQ4.*m6.*t2.*t8.*t20.*t34.*t35.*2.0;
t2215 = dQ1.*dQ4.*m6.*t3.*t7.*t20.*t34.*t35.*2.0;
t2230 = t35.*t36.*t294.*-2.0;
t2231 = t35.*t1747;
t2232 = Lxcm6.*Lycm6.*dQ1.*dQ6.*m6.*t5.*t7.*t8.*t9.*t10.*t36.*4.0;
t2237 = dQ1.*dQ6.*m6.*t2.*t3.*t4.*t10.*t20.*t36.*-2.0;
t2243 = t4.*t5.*t6.*t9.*t11.*t267.*2.0;
t2244 = t4.*t5.*t6.*t9.*t11.*t268.*2.0;
t2245 = t4.*t5.*t6.*t9.*t11.*t280.*2.0;
t2246 = t4.*t5.*t6.*t9.*t11.*t281.*2.0;
t2263 = -t2176;
t2264 = -t2177;
t2265 = -t2178;
t2266 = -t2179;
t2267 = -t2180;
t2268 = -t2181;
t2269 = -t2182;
t2270 = -t2197;
t2271 = dQ2.*dQ4.*m6.*t4.*t9.*t17.*t35.*t36.*-2.0;
t2272 = dQ3.*dQ4.*m6.*t4.*t9.*t17.*t35.*t36.*-2.0;
t2273 = dQ2.*dQ5.*m6.*t5.*t10.*t17.*t34.*t36.*-2.0;
t2274 = dQ3.*dQ5.*m6.*t5.*t10.*t17.*t34.*t36.*-2.0;
t2275 = dQ2.*dQ6.*m6.*t6.*t11.*t17.*t34.*t35.*-2.0;
t2276 = dQ3.*dQ6.*m6.*t6.*t11.*t17.*t34.*t35.*-2.0;
t2277 = dQ1.*dQ4.*m6.*t2.*t8.*t20.*t34.*t36.*-2.0;
t2278 = dQ1.*dQ4.*m6.*t3.*t7.*t20.*t34.*t36.*-2.0;
t2279 = dQ1.*dQ4.*m6.*t2.*t8.*t22.*t34.*t35.*-2.0;
t2280 = dQ1.*dQ4.*m6.*t3.*t7.*t22.*t34.*t35.*-2.0;
t2281 = dQ1.*dQ4.*m5.*t2.*t8.*t25.*t34.*t35.*-2.0;
t2282 = dQ1.*dQ4.*m5.*t3.*t7.*t25.*t34.*t35.*-2.0;
t2283 = dQ1.*dQ4.*m6.*t2.*t8.*t26.*t34.*t35.*-2.0;
t2284 = dQ1.*dQ4.*m6.*t3.*t7.*t26.*t34.*t35.*-2.0;
t2286 = Lxcm6.*Lycm6.*dQ1.*dQ6.*m6.*t2.*t3.*t5.*t9.*t10.*t36.*4.0;
t2287 = Lxcm6.*Lz5.*dQ1.*dQ4.*m6.*t2.*t5.*t6.*t8.*t10.*t34.*4.0;
t2288 = Lxcm6.*Lz5.*dQ1.*dQ4.*m6.*t3.*t5.*t6.*t7.*t10.*t34.*4.0;
t2289 = Lxcm6.*Lz5.*dQ1.*dQ5.*m6.*t2.*t4.*t6.*t8.*t9.*t35.*4.0;
t2290 = Lxcm6.*Lz5.*dQ1.*dQ5.*m6.*t3.*t4.*t6.*t7.*t9.*t35.*4.0;
t2291 = Lxcm6.*Lzcm6.*dQ1.*dQ4.*m6.*t2.*t5.*t6.*t8.*t10.*t34.*4.0;
t2292 = Lxcm6.*Lzcm6.*dQ1.*dQ4.*m6.*t3.*t5.*t6.*t7.*t10.*t34.*4.0;
t2293 = Lxcm6.*Lzcm6.*dQ1.*dQ5.*m6.*t2.*t4.*t6.*t8.*t9.*t35.*4.0;
t2294 = Lxcm6.*Lzcm6.*dQ1.*dQ5.*m6.*t3.*t4.*t6.*t7.*t9.*t35.*4.0;
t2295 = Ixx6.*dQ1.*dQ5.*t2.*t4.*t5.*t8.*t9.*t10.*t36.*2.0;
t2296 = Ixx6.*dQ1.*dQ5.*t3.*t4.*t5.*t7.*t9.*t10.*t36.*2.0;
t2297 = t35.*t1697;
t2298 = t35.*t1698;
t2303 = Lycm6.*Lz5.*dQ1.*dQ4.*m6.*t2.*t5.*t8.*t10.*t11.*t34.*4.0;
t2304 = Lycm6.*Lz5.*dQ1.*dQ4.*m6.*t3.*t5.*t7.*t10.*t11.*t34.*4.0;
t2305 = Lycm6.*Lz5.*dQ1.*dQ5.*m6.*t2.*t4.*t8.*t9.*t11.*t35.*4.0;
t2306 = Lycm6.*Lz5.*dQ1.*dQ5.*m6.*t3.*t4.*t7.*t9.*t11.*t35.*4.0;
t2307 = Lycm6.*Lzcm6.*dQ1.*dQ4.*m6.*t2.*t5.*t8.*t10.*t11.*t34.*4.0;
t2308 = Lycm6.*Lzcm6.*dQ1.*dQ4.*m6.*t3.*t5.*t7.*t10.*t11.*t34.*4.0;
t2309 = Lycm6.*Lzcm6.*dQ1.*dQ5.*m6.*t2.*t4.*t8.*t9.*t11.*t35.*4.0;
t2310 = Lycm6.*Lzcm6.*dQ1.*dQ5.*m6.*t3.*t4.*t7.*t9.*t11.*t35.*4.0;
t2311 = dQ1.*dQ4.*m6.*t4.*t5.*t7.*t8.*t10.*t17.*t36.*2.0;
t2314 = t36.*t1929;
t2315 = t34.*t1930;
t2316 = t34.*t1931;
t2319 = -t2238;
t2320 = -t2239;
t2321 = -t2240;
t2322 = -t2241;
t2323 = -t2242;
t2324 = -t2249;
t2325 = -t2250;
t2326 = -t2251;
t2327 = -t2252;
t2344 = Lxcm6.*Lycm6.*dQ1.*dQ5.*m6.*t2.*t8.*t10.*t34.*t36.*-4.0;
t2345 = Lxcm6.*Lycm6.*dQ1.*dQ5.*m6.*t3.*t7.*t10.*t34.*t36.*-4.0;
t2347 = dQ1.*dQ6.*m6.*t2.*t5.*t8.*t17.*t34.*t36.*4.0;
t2348 = dQ1.*dQ6.*m6.*t3.*t5.*t7.*t17.*t34.*t36.*4.0;
t2350 = dQ1.*dQ6.*m6.*t2.*t5.*t8.*t20.*t34.*t36.*4.0;
t2351 = dQ1.*dQ6.*m6.*t3.*t5.*t7.*t20.*t34.*t36.*4.0;
t2354 = Lxcm6.*Lycm6.*dQ1.*dQ5.*m6.*t2.*t3.*t6.*t9.*t11.*t35.*-4.0;
t2356 = Lxcm6.*Lycm6.*dQ1.*dQ4.*m6.*t2.*t4.*t5.*t8.*t9.*t36.*8.0;
t2357 = Lxcm6.*Lycm6.*dQ1.*dQ4.*m6.*t3.*t4.*t5.*t7.*t9.*t36.*8.0;
t2358 = Lxcm6.*Lycm6.*dQ1.*dQ6.*m6.*t2.*t5.*t6.*t8.*t11.*t34.*8.0;
t2359 = Lxcm6.*Lycm6.*dQ1.*dQ6.*m6.*t3.*t5.*t6.*t7.*t11.*t34.*8.0;
t2360 = dQ1.*dQ4.*m6.*t2.*t3.*t4.*t5.*t10.*t17.*t36.*2.0;
t2362 = Iyy6.*dQ1.*dQ5.*t2.*t4.*t5.*t8.*t9.*t10.*t36.*-2.0;
t2363 = Iyy6.*dQ1.*dQ5.*t3.*t4.*t5.*t7.*t9.*t10.*t36.*-2.0;
t2364 = Iyy6.*dQ1.*dQ6.*t2.*t4.*t6.*t8.*t9.*t11.*t35.*-2.0;
t2365 = Iyy6.*dQ1.*dQ6.*t3.*t4.*t6.*t7.*t9.*t11.*t35.*-2.0;
t2375 = dQ1.*dQ5.*m6.*t2.*t6.*t8.*t10.*t11.*t17.*t34.*-2.0;
t2376 = dQ1.*dQ5.*m6.*t3.*t6.*t7.*t10.*t11.*t17.*t34.*-2.0;
t2383 = -t2328;
t2384 = -t2329;
t2385 = -t2330;
t2386 = -t2335;
t2387 = dQ1.*dQ5.*m6.*t2.*t3.*t9.*t20.*t35.*t36.*-2.0;
t2390 = dQ1.*dQ5.*m6.*t7.*t8.*t9.*t17.*t35.*t36.*-2.0;
t2395 = dQ1.*dQ4.*m6.*t2.*t3.*t4.*t5.*t10.*t20.*t36.*-2.0;
t2398 = Lxcm6.*Lycm6.*dQ1.*dQ6.*m6.*t2.*t4.*t8.*t9.*t35.*t36.*-4.0;
t2399 = Lxcm6.*Lycm6.*dQ1.*dQ6.*m6.*t3.*t4.*t7.*t9.*t35.*t36.*-4.0;
t2400 = dQ1.*dQ5.*m6.*t2.*t4.*t5.*t8.*t9.*t10.*t17.*t36.*2.0;
t2401 = dQ1.*dQ5.*m6.*t3.*t4.*t5.*t7.*t9.*t10.*t17.*t36.*2.0;
t2404 = t36.*t2181;
t2405 = t36.*t2182;
t2406 = t35.*t2184;
t2407 = t35.*t2185;
t2414 = dQ1.*dQ6.*m6.*t2.*t4.*t6.*t8.*t9.*t11.*t17.*t35.*-2.0;
t2415 = dQ1.*dQ6.*m6.*t3.*t4.*t6.*t7.*t9.*t11.*t17.*t35.*-2.0;
t205 = -t158;
t206 = -t159;
t207 = -t95;
t208 = -t97;
t209 = -t98;
t210 = -t99;
t211 = -t160;
t212 = -t161;
t213 = -t162;
t214 = -t163;
t215 = -t101;
t216 = -t103;
t217 = -t104;
t218 = -t105;
t219 = -t164;
t220 = -t165;
t227 = -t108;
t228 = -t109;
t229 = -t110;
t230 = -t111;
t231 = -t112;
t232 = -t113;
t233 = -t114;
t234 = -t115;
t235 = -t116;
t236 = -t117;
t463 = -t329;
t464 = -t330;
t465 = -t335;
t466 = -t197;
t467 = -t198;
t468 = -t336;
t469 = -t337;
t470 = -t338;
t471 = -t339;
t472 = -t344;
t473 = -t199;
t474 = -t200;
t475 = -t345;
t476 = -t346;
t477 = -t347;
t478 = -t348;
t479 = -t350;
t480 = -t352;
t483 = -t355;
t484 = -t356;
t487 = -t357;
t488 = -t359;
t489 = -t360;
t490 = -t361;
t491 = -t362;
t492 = -t365;
t493 = -t366;
t494 = -t371;
t495 = -t372;
t496 = -t373;
t497 = -t374;
t564 = t35.*t94;
t565 = t35.*t96;
t566 = t35.*t100;
t567 = t35.*t102;
t698 = -t375;
out1 = ft_4({Ixx2,Ixx3,Ixx4,Ixx5,Ixx6,Ixy3,Ixy4,Ixy5,Ixy6,Ixz2,Ixz3,Ixz4,Ixz5,Ixz6,Iyx3,Iyx4,Iyx5,Iyx6,Iyy4,Iyy5,Iyy6,Iyz3,Iyz4,Iyz5,Iyz6,Izx2,Izx3,Izx4,Izx5,Izx6,Izy3,Izy4,Izy5,Izy6,Izz2,Izz3,Izz4,Izz5,Izz6,Lx2,Lx3,Lxcm2,Lxcm3,Lxcm4,Lxcm5,Lxcm6,Lycm3,Lycm4,Lycm5,Lycm6,Lz4,Lz5,Lzcm2,Lzcm3,Lzcm4,Lzcm5,Lzcm6,dQ1,dQ2,dQ3,dQ4,dQ5,dQ6,m2,m3,m4,m5,m6,t10,t100,t101,t102,t103,t1033,t1034,t1035,t1036,t1037,t1038,t1039,t104,t1041,t1046,t105,t106,t1060,t1061,t1062,t1063,t1064,t1065,t1066,t1067,t107,t1072,t1073,t1074,t1075,t1076,t1077,t1078,t1079,t1093,t1094,t1095,t1096,t1097,t1098,t1099,t11,t1100,t1101,t1103,t1104,t1105,t1106,t1107,t1108,t1109,t1110,t1111,t1112,t1113,t1114,t1115,t1116,t1117,t1118,t1120,t1127,t1139,t1140,t1145,t1146,t1147,t1148,t1149,t1150,t1154,t1155,t1158,t1159,t1167,t1169,t1170,t1173,t1174,t1175,t1177,t1178,t1179,t118,t1180,t1181,t1182,t1187,t119,t1191,t1192,t1195,t1196,t12,t120,t1201,t1202,t1203,t1204,t121,t1213,t1214,t1215,t1216,t1217,t1218,t1219,t122,t1220,t1221,t1222,t1223,t1224,t1225,t1226,t1227,t1228,t1229,t123,t1230,t1231,t1232,t1233,t1234,t1235,t1236,t1237,t1238,t1239,t124,t1240,t1241,t1242,t1243,t1244,t1245,t1246,t1247,t1248,t1249,t125,t1250,t1251,t1252,t1253,t1254,t1255,t1256,t1257,t1258,t1259,t126,t1261,t1262,t1263,t1264,t1265,t1266,t1268,t1269,t127,t1270,t1271,t1272,t1273,t1274,t1275,t1276,t1277,t1278,t1279,t128,t1280,t1281,t1283,t1285,t1286,t1287,t1288,t1289,t129,t1290,t1291,t1292,t1293,t1294,t1295,t1296,t1297,t1298,t1299,t13,t130,t1300,t1301,t1302,t1303,t1304,t1305,t1306,t1307,t1308,t1309,t131,t1310,t1311,t1312,t1313,t1314,t1315,t1316,t1317,t1318,t1319,t132,t1320,t1321,t1322,t1323,t1324,t1325,t1326,t1327,t1328,t1329,t1330,t1331,t1332,t1333,t1334,t1335,t1336,t1337,t1338,t1339,t134,t1340,t1341,t1342,t1343,t1344,t1345,t1346,t1347,t1348,t1349,t1350,t1351,t1352,t1353,t1354,t1355,t1356,t1357,t1358,t1359,t136,t1360,t1361,t1362,t1363,t1364,t1365,t1366,t1367,t1368,t1369,t137,t1370,t1371,t1372,t1373,t1374,t1375,t1376,t1377,t1378,t1379,t138,t1387,t139,t1392,t1393,t1394,t1395,t1396,t1397,t1398,t1399,t14,t140,t1400,t1401,t1402,t1403,t1404,t1405,t1406,t1407,t1408,t1409,t141,t1410,t1411,t1412,t1413,t1414,t1415,t1416,t1417,t1418,t1419,t142,t143,t144,t1443,t1449,t145,t1457,t1458,t1459,t146,t1460,t1461,t1462,t1463,t1464,t1465,t1466,t1467,t1468,t1469,t147,t1470,t1471,t1472,t1473,t1474,t1475,t148,t1481,t1482,t1483,t1484,t1485,t1486,t1487,t1488,t1489,t149,t1490,t1491,t1492,t1493,t1495,t1496,t1497,t1498,t1499,t15,t150,t1500,t1501,t1502,t1503,t1504,t1505,t1506,t1507,t1508,t1509,t151,t1510,t1511,t1512,t1513,t1514,t1518,t1519,t152,t1520,t1521,t1522,t1527,t1528,t153,t1537,t1538,t154,t155,t1555,t1556,t1557,t1558,t1559,t156,t1560,t1561,t1562,t1565,t1566,t1569,t157,t1570,t1573,t1574,t1575,t1576,t1577,t1578,t1579,t1580,t1581,t1582,t1583,t1584,t1587,t1588,t1589,t1590,t1591,t1592,t1593,t1594,t1595,t1596,t1597,t16,t160,t1600,t1601,t1602,t1603,t1604,t1605,t1607,t161,t1610,t1613,t1614,t1615,t1616,t1617,t1618,t1619,t1627,t1628,t1629,t1630,t1631,t1632,t1633,t1634,t1637,t1639,t164,t1640,t1641,t1642,t1643,t165,t1652,t1653,t1654,t1655,t1656,t1664,t1672,t1673,t1674,t1675,t1676,t1677,t1678,t1679,t1680,t1683,t1684,t1687,t1688,t1691,t1694,t1695,t1696,t1697,t1698,t1699,t17,t170,t1700,t171,t172,t1721,t1722,t1725,t1726,t173,t1730,t1731,t1733,t1734,t1735,t1736,t174,t1740,t1744,t1745,t1754,t1755,t1756,t1757,t1758,t1761,t1762,t1765,t1766,t1767,t1768,t1769,t177,t1770,t1771,t1772,t1773,t1774,t178,t1781,t1782,t1783,t1784,t1787,t1788,t179,t1792,t1793,t1796,t1797,t1798,t18,t180,t1800,t1801,t1802,t1803,t1804,t1805,t1808,t1809,t1810,t1811,t1812,t1813,t1814,t1815,t1816,t1817,t1818,t1819,t1820,t1821,t1822,t1823,t1824,t1825,t1826,t183,t184,t1847,t1848,t185,t1850,t1851,t1852,t1857,t1858,t1859,t186,t1860,t1861,t1862,t1863,t1864,t1865,t1866,t1867,t1868,t1869,t187,t1870,t1871,t1872,t1873,t1874,t1875,t1876,t1877,t1878,t1879,t188,t1880,t1884,t1885,t1886,t1887,t1888,t1889,t1890,t1891,t1892,t1893,t1894,t1895,t1896,t1897,t1898,t1899,t19,t1900,t1901,t1902,t1903,t1904,t1905,t1906,t1907,t1908,t1909,t1910,t1911,t1912,t1913,t1914,t1915,t1916,t1917,t1918,t1919,t1920,t1921,t1922,t1924,t1925,t1926,t1927,t1934,t1935,t1936,t1937,t1938,t1941,t1942,t1943,t1944,t1945,t1946,t1947,t1948,t1949,t1950,t1951,t1952,t1953,t1954,t1956,t1957,t1958,t1959,t1960,t1961,t1962,t1963,t1964,t1966,t1967,t1968,t1969,t197,t1970,t1971,t1972,t1973,t1974,t1975,t1976,t1979,t198,t1980,t1981,t1982,t1983,t1984,t1985,t1986,t1987,t1988,t1989,t199,t1990,t1991,t1992,t1993,t1994,t1995,t1996,t1997,t1998,t1999,t2,t20,t200,t2000,t2001,t2002,t2003,t2007,t2008,t2009,t201,t2010,t2011,t2012,t2013,t2014,t2015,t2016,t2017,t2018,t2019,t202,t2020,t2021,t2022,t2023,t2024,t2025,t2026,t2027,t2028,t2029,t203,t2035,t2036,t2037,t2038,t204,t2047,t2048,t2049,t205,t2050,t2051,t2052,t2053,t206,t2061,t2062,t2063,t2064,t2065,t2066,t2067,t2068,t207,t2076,t2077,t2078,t208,t2080,t2081,t2083,t2084,t209,t2091,t2092,t2093,t2096,t2097,t2098,t2099,t21,t210,t2100,t2101,t2102,t2108,t211,t2114,t2119,t212,t2120,t2123,t2125,t2126,t2127,t213,t214,t2146,t2147,t2148,t2149,t215,t2150,t2151,t2152,t2155,t2156,t2157,t2158,t2159,t216,t2160,t2161,t2162,t2163,t2164,t2165,t2166,t2167,t2168,t2169,t217,t2170,t2171,t2172,t2173,t2174,t2175,t218,t2183,t2184,t2185,t2186,t2187,t2188,t2189,t219,t2190,t2191,t2192,t2193,t2196,t2198,t2199,t22,t220,t2204,t2205,t2214,t2215,t222,t2230,t2231,t2232,t2237,t2243,t2244,t2245,t2246,t2248,t225,t2263,t2264,t2265,t2266,t2267,t2268,t2269,t227,t2270,t2271,t2272,t2273,t2274,t2275,t2276,t2277,t2278,t2279,t228,t2280,t2281,t2282,t2283,t2284,t2286,t2287,t2288,t2289,t229,t2290,t2291,t2292,t2293,t2294,t2295,t2296,t2297,t2298,t23,t230,t2303,t2304,t2305,t2306,t2307,t2308,t2309,t231,t2310,t2311,t2314,t2315,t2316,t2319,t232,t2320,t2321,t2322,t2323,t2324,t2325,t2326,t2327,t233,t2331,t2332,t2333,t2334,t234,t2344,t2345,t2347,t2348,t235,t2350,t2351,t2354,t2356,t2357,t2358,t2359,t236,t2360,t2362,t2363,t2364,t2365,t237,t2375,t2376,t2377,t2378,t238,t2383,t2384,t2385,t2386,t2387,t239,t2390,t2395,t2398,t2399,t24,t240,t2400,t2401,t2404,t2405,t2406,t2407,t2414,t2415,t242,t243,t244,t245,t246,t25,t250,t251,t252,t253,t254,t258,t259,t26,t260,t263,t264,t265,t266,t267,t269,t270,t271,t272,t273,t274,t276,t277,t278,t279,t280,t282,t283,t284,t285,t286,t287,t289,t290,t292,t293,t297,t298,t299,t3,t300,t301,t302,t303,t304,t305,t306,t307,t308,t309,t310,t311,t312,t313,t314,t315,t316,t317,t318,t319,t32,t320,t321,t322,t323,t324,t325,t326,t327,t328,t33,t331,t332,t333,t334,t336,t337,t34,t340,t341,t342,t343,t345,t346,t349,t35,t350,t351,t352,t355,t356,t358,t359,t36,t363,t364,t367,t368,t369,t37,t370,t376,t377,t378,t379,t38,t380,t381,t382,t383,t384,t385,t386,t387,t388,t389,t39,t390,t391,t392,t393,t394,t395,t396,t397,t398,t4,t40,t402,t403,t404,t405,t406,t407,t41,t413,t414,t415,t416,t417,t418,t419,t42,t43,t430,t431,t432,t433,t434,t435,t436,t437,t438,t44,t442,t443,t444,t445,t446,t447,t45,t454,t455,t456,t457,t458,t459,t46,t460,t461,t462,t463,t464,t465,t466,t467,t468,t469,t47,t470,t471,t472,t473,t474,t475,t476,t477,t478,t479,t48,t480,t481,t482,t483,t484,t485,t486,t487,t488,t489,t49,t490,t491,t492,t493,t494,t495,t496,t497,t498,t5,t50,t500,t501,t502,t506,t507,t508,t51,t512,t514,t515,t516,t52,t520,t527,t528,t529,t53,t533,t54,t540,t542,t543,t544,t546,t547,t548,t55,t550,t552,t554,t555,t556,t557,t558,t559,t56,t560,t561,t562,t563,t564,t565,t566,t567,t568,t569,t57,t570,t571,t572,t573,t574,t575,t576,t577,t578,t579,t58,t580,t581,t582,t583,t584,t585,t586,t587,t588,t589,t59,t590,t591,t592,t593,t594,t595,t596,t597,t598,t599,t6,t60,t600,t601,t602,t603,t604,t605,t606,t607,t608,t609,t61,t610,t611,t612,t613,t614,t615,t616,t617,t618,t619,t62,t620,t621,t622,t623,t624,t625,t626,t627,t628,t629,t63,t630,t631,t632,t633,t634,t635,t636,t637,t638,t639,t64,t640,t641,t642,t643,t648,t650,t651,t658,t659,t660,t661,t662,t663,t664,t669,t67,t670,t671,t674,t675,t676,t677,t68,t681,t684,t687,t688,t689,t69,t690,t694,t697,t698,t7,t70,t71,t716,t717,t718,t719,t72,t720,t721,t724,t725,t728,t729,t73,t730,t731,t732,t733,t734,t735,t737,t738,t739,t74,t75,t757,t758,t759,t760,t761,t762,t763,t766,t767,t770,t771,t772,t773,t774,t775,t776,t777,t778,t779,t78,t780,t781,t782,t783,t784,t785,t786,t787,t788,t789,t79,t790,t791,t792,t793,t794,t795,t796,t797,t798,t799,t8,t80,t800,t801,t802,t803,t804,t805,t806,t807,t808,t809,t81,t810,t811,t812,t813,t814,t815,t816,t817,t818,t819,t82,t820,t821,t822,t823,t824,t825,t826,t827,t83,t831,t832,t833,t834,t839,t84,t840,t843,t844,t845,t848,t849,t85,t850,t851,t852,t853,t854,t855,t857,t858,t86,t861,t862,t868,t869,t87,t870,t871,t872,t873,t874,t875,t876,t877,t878,t879,t88,t880,t881,t882,t883,t884,t885,t886,t887,t888,t889,t89,t890,t891,t892,t893,t894,t895,t896,t897,t898,t899,t9,t90,t900,t901,t902,t903,t904,t905,t906,t907,t908,t909,t91,t910,t911,t912,t913,t914,t915,t916,t917,t918,t919,t92,t920,t921,t922,t923,t924,t925,t926,t927,t928,t929,t93,t930,t931,t932,t933,t934,t935,t936,t938,t939,t94,t940,t941,t942,t943,t948,t949,t95,t950,t951,t952,t953,t954,t955,t956,t957,t958,t959,t96,t960,t961,t962,t963,t968,t969,t97,t970,t971,t972,t973,t974,t975,t976,t977,t978,t979,t98,t980,t981,t982,t983,t984,t985,t986,t987,t99,t991,t992,t995,t996});
end
function out1 = ft_4(ct)
[Ixx2,Ixx3,Ixx4,Ixx5,Ixx6,Ixy3,Ixy4,Ixy5,Ixy6,Ixz2,Ixz3,Ixz4,Ixz5,Ixz6,Iyx3,Iyx4,Iyx5,Iyx6,Iyy4,Iyy5,Iyy6,Iyz3,Iyz4,Iyz5,Iyz6,Izx2,Izx3,Izx4,Izx5,Izx6,Izy3,Izy4,Izy5,Izy6,Izz2,Izz3,Izz4,Izz5,Izz6,Lx2,Lx3,Lxcm2,Lxcm3,Lxcm4,Lxcm5,Lxcm6,Lycm3,Lycm4,Lycm5,Lycm6,Lz4,Lz5,Lzcm2,Lzcm3,Lzcm4,Lzcm5,Lzcm6,dQ1,dQ2,dQ3,dQ4,dQ5,dQ6,m2,m3,m4,m5,m6,t10,t100,t101,t102,t103,t1033,t1034,t1035,t1036,t1037,t1038,t1039,t104,t1041,t1046,t105,t106,t1060,t1061,t1062,t1063,t1064,t1065,t1066,t1067,t107,t1072,t1073,t1074,t1075,t1076,t1077,t1078,t1079,t1093,t1094,t1095,t1096,t1097,t1098,t1099,t11,t1100,t1101,t1103,t1104,t1105,t1106,t1107,t1108,t1109,t1110,t1111,t1112,t1113,t1114,t1115,t1116,t1117,t1118,t1120,t1127,t1139,t1140,t1145,t1146,t1147,t1148,t1149,t1150,t1154,t1155,t1158,t1159,t1167,t1169,t1170,t1173,t1174,t1175,t1177,t1178,t1179,t118,t1180,t1181,t1182,t1187,t119,t1191,t1192,t1195,t1196,t12,t120,t1201,t1202,t1203,t1204,t121,t1213,t1214,t1215,t1216,t1217,t1218,t1219,t122,t1220,t1221,t1222,t1223,t1224,t1225,t1226,t1227,t1228,t1229,t123,t1230,t1231,t1232,t1233,t1234,t1235,t1236,t1237,t1238,t1239,t124,t1240,t1241,t1242,t1243,t1244,t1245,t1246,t1247,t1248,t1249,t125,t1250,t1251,t1252,t1253,t1254,t1255,t1256,t1257,t1258,t1259,t126,t1261,t1262,t1263,t1264,t1265,t1266,t1268,t1269,t127,t1270,t1271,t1272,t1273,t1274,t1275,t1276,t1277,t1278,t1279,t128,t1280,t1281,t1283,t1285,t1286,t1287,t1288,t1289,t129,t1290,t1291,t1292,t1293,t1294,t1295,t1296,t1297,t1298,t1299,t13,t130,t1300,t1301,t1302,t1303,t1304,t1305,t1306,t1307,t1308,t1309,t131,t1310,t1311,t1312,t1313,t1314,t1315,t1316,t1317,t1318,t1319,t132,t1320,t1321,t1322,t1323,t1324,t1325,t1326,t1327,t1328,t1329,t1330,t1331,t1332,t1333,t1334,t1335,t1336,t1337,t1338,t1339,t134,t1340,t1341,t1342,t1343,t1344,t1345,t1346,t1347,t1348,t1349,t1350,t1351,t1352,t1353,t1354,t1355,t1356,t1357,t1358,t1359,t136,t1360,t1361,t1362,t1363,t1364,t1365,t1366,t1367,t1368,t1369,t137,t1370,t1371,t1372,t1373,t1374,t1375,t1376,t1377,t1378,t1379,t138,t1387,t139,t1392,t1393,t1394,t1395,t1396,t1397,t1398,t1399,t14,t140,t1400,t1401,t1402,t1403,t1404,t1405,t1406,t1407,t1408,t1409,t141,t1410,t1411,t1412,t1413,t1414,t1415,t1416,t1417,t1418,t1419,t142,t143,t144,t1443,t1449,t145,t1457,t1458,t1459,t146,t1460,t1461,t1462,t1463,t1464,t1465,t1466,t1467,t1468,t1469,t147,t1470,t1471,t1472,t1473,t1474,t1475,t148,t1481,t1482,t1483,t1484,t1485,t1486,t1487,t1488,t1489,t149,t1490,t1491,t1492,t1493,t1495,t1496,t1497,t1498,t1499,t15,t150,t1500,t1501,t1502,t1503,t1504,t1505,t1506,t1507,t1508,t1509,t151,t1510,t1511,t1512,t1513,t1514,t1518,t1519,t152,t1520,t1521,t1522,t1527,t1528,t153,t1537,t1538,t154,t155,t1555,t1556,t1557,t1558,t1559,t156,t1560,t1561,t1562,t1565,t1566,t1569,t157,t1570,t1573,t1574,t1575,t1576,t1577,t1578,t1579,t1580,t1581,t1582,t1583,t1584,t1587,t1588,t1589,t1590,t1591,t1592,t1593,t1594,t1595,t1596,t1597,t16,t160,t1600,t1601,t1602,t1603,t1604,t1605,t1607,t161,t1610,t1613,t1614,t1615,t1616,t1617,t1618,t1619,t1627,t1628,t1629,t1630,t1631,t1632,t1633,t1634,t1637,t1639,t164,t1640,t1641,t1642,t1643,t165,t1652,t1653,t1654,t1655,t1656,t1664,t1672,t1673,t1674,t1675,t1676,t1677,t1678,t1679,t1680,t1683,t1684,t1687,t1688,t1691,t1694,t1695,t1696,t1697,t1698,t1699,t17,t170,t1700,t171,t172,t1721,t1722,t1725,t1726,t173,t1730,t1731,t1733,t1734,t1735,t1736,t174,t1740,t1744,t1745,t1754,t1755,t1756,t1757,t1758,t1761,t1762,t1765,t1766,t1767,t1768,t1769,t177,t1770,t1771,t1772,t1773,t1774,t178,t1781,t1782,t1783,t1784,t1787,t1788,t179,t1792,t1793,t1796,t1797,t1798,t18,t180,t1800,t1801,t1802,t1803,t1804,t1805,t1808,t1809,t1810,t1811,t1812,t1813,t1814,t1815,t1816,t1817,t1818,t1819,t1820,t1821,t1822,t1823,t1824,t1825,t1826,t183,t184,t1847,t1848,t185,t1850,t1851,t1852,t1857,t1858,t1859,t186,t1860,t1861,t1862,t1863,t1864,t1865,t1866,t1867,t1868,t1869,t187,t1870,t1871,t1872,t1873,t1874,t1875,t1876,t1877,t1878,t1879,t188,t1880,t1884,t1885,t1886,t1887,t1888,t1889,t1890,t1891,t1892,t1893,t1894,t1895,t1896,t1897,t1898,t1899,t19,t1900,t1901,t1902,t1903,t1904,t1905,t1906,t1907,t1908,t1909,t1910,t1911,t1912,t1913,t1914,t1915,t1916,t1917,t1918,t1919,t1920,t1921,t1922,t1924,t1925,t1926,t1927,t1934,t1935,t1936,t1937,t1938,t1941,t1942,t1943,t1944,t1945,t1946,t1947,t1948,t1949,t1950,t1951,t1952,t1953,t1954,t1956,t1957,t1958,t1959,t1960,t1961,t1962,t1963,t1964,t1966,t1967,t1968,t1969,t197,t1970,t1971,t1972,t1973,t1974,t1975,t1976,t1979,t198,t1980,t1981,t1982,t1983,t1984,t1985,t1986,t1987,t1988,t1989,t199,t1990,t1991,t1992,t1993,t1994,t1995,t1996,t1997,t1998,t1999,t2,t20,t200,t2000,t2001,t2002,t2003,t2007,t2008,t2009,t201,t2010,t2011,t2012,t2013,t2014,t2015,t2016,t2017,t2018,t2019,t202,t2020,t2021,t2022,t2023,t2024,t2025,t2026,t2027,t2028,t2029,t203,t2035,t2036,t2037,t2038,t204,t2047,t2048,t2049,t205,t2050,t2051,t2052,t2053,t206,t2061,t2062,t2063,t2064,t2065,t2066,t2067,t2068,t207,t2076,t2077,t2078,t208,t2080,t2081,t2083,t2084,t209,t2091,t2092,t2093,t2096,t2097,t2098,t2099,t21,t210,t2100,t2101,t2102,t2108,t211,t2114,t2119,t212,t2120,t2123,t2125,t2126,t2127,t213,t214,t2146,t2147,t2148,t2149,t215,t2150,t2151,t2152,t2155,t2156,t2157,t2158,t2159,t216,t2160,t2161,t2162,t2163,t2164,t2165,t2166,t2167,t2168,t2169,t217,t2170,t2171,t2172,t2173,t2174,t2175,t218,t2183,t2184,t2185,t2186,t2187,t2188,t2189,t219,t2190,t2191,t2192,t2193,t2196,t2198,t2199,t22,t220,t2204,t2205,t2214,t2215,t222,t2230,t2231,t2232,t2237,t2243,t2244,t2245,t2246,t2248,t225,t2263,t2264,t2265,t2266,t2267,t2268,t2269,t227,t2270,t2271,t2272,t2273,t2274,t2275,t2276,t2277,t2278,t2279,t228,t2280,t2281,t2282,t2283,t2284,t2286,t2287,t2288,t2289,t229,t2290,t2291,t2292,t2293,t2294,t2295,t2296,t2297,t2298,t23,t230,t2303,t2304,t2305,t2306,t2307,t2308,t2309,t231,t2310,t2311,t2314,t2315,t2316,t2319,t232,t2320,t2321,t2322,t2323,t2324,t2325,t2326,t2327,t233,t2331,t2332,t2333,t2334,t234,t2344,t2345,t2347,t2348,t235,t2350,t2351,t2354,t2356,t2357,t2358,t2359,t236,t2360,t2362,t2363,t2364,t2365,t237,t2375,t2376,t2377,t2378,t238,t2383,t2384,t2385,t2386,t2387,t239,t2390,t2395,t2398,t2399,t24,t240,t2400,t2401,t2404,t2405,t2406,t2407,t2414,t2415,t242,t243,t244,t245,t246,t25,t250,t251,t252,t253,t254,t258,t259,t26,t260,t263,t264,t265,t266,t267,t269,t270,t271,t272,t273,t274,t276,t277,t278,t279,t280,t282,t283,t284,t285,t286,t287,t289,t290,t292,t293,t297,t298,t299,t3,t300,t301,t302,t303,t304,t305,t306,t307,t308,t309,t310,t311,t312,t313,t314,t315,t316,t317,t318,t319,t32,t320,t321,t322,t323,t324,t325,t326,t327,t328,t33,t331,t332,t333,t334,t336,t337,t34,t340,t341,t342,t343,t345,t346,t349,t35,t350,t351,t352,t355,t356,t358,t359,t36,t363,t364,t367,t368,t369,t37,t370,t376,t377,t378,t379,t38,t380,t381,t382,t383,t384,t385,t386,t387,t388,t389,t39,t390,t391,t392,t393,t394,t395,t396,t397,t398,t4,t40,t402,t403,t404,t405,t406,t407,t41,t413,t414,t415,t416,t417,t418,t419,t42,t43,t430,t431,t432,t433,t434,t435,t436,t437,t438,t44,t442,t443,t444,t445,t446,t447,t45,t454,t455,t456,t457,t458,t459,t46,t460,t461,t462,t463,t464,t465,t466,t467,t468,t469,t47,t470,t471,t472,t473,t474,t475,t476,t477,t478,t479,t48,t480,t481,t482,t483,t484,t485,t486,t487,t488,t489,t49,t490,t491,t492,t493,t494,t495,t496,t497,t498,t5,t50,t500,t501,t502,t506,t507,t508,t51,t512,t514,t515,t516,t52,t520,t527,t528,t529,t53,t533,t54,t540,t542,t543,t544,t546,t547,t548,t55,t550,t552,t554,t555,t556,t557,t558,t559,t56,t560,t561,t562,t563,t564,t565,t566,t567,t568,t569,t57,t570,t571,t572,t573,t574,t575,t576,t577,t578,t579,t58,t580,t581,t582,t583,t584,t585,t586,t587,t588,t589,t59,t590,t591,t592,t593,t594,t595,t596,t597,t598,t599,t6,t60,t600,t601,t602,t603,t604,t605,t606,t607,t608,t609,t61,t610,t611,t612,t613,t614,t615,t616,t617,t618,t619,t62,t620,t621,t622,t623,t624,t625,t626,t627,t628,t629,t63,t630,t631,t632,t633,t634,t635,t636,t637,t638,t639,t64,t640,t641,t642,t643,t648,t650,t651,t658,t659,t660,t661,t662,t663,t664,t669,t67,t670,t671,t674,t675,t676,t677,t68,t681,t684,t687,t688,t689,t69,t690,t694,t697,t698,t7,t70,t71,t716,t717,t718,t719,t72,t720,t721,t724,t725,t728,t729,t73,t730,t731,t732,t733,t734,t735,t737,t738,t739,t74,t75,t757,t758,t759,t760,t761,t762,t763,t766,t767,t770,t771,t772,t773,t774,t775,t776,t777,t778,t779,t78,t780,t781,t782,t783,t784,t785,t786,t787,t788,t789,t79,t790,t791,t792,t793,t794,t795,t796,t797,t798,t799,t8,t80,t800,t801,t802,t803,t804,t805,t806,t807,t808,t809,t81,t810,t811,t812,t813,t814,t815,t816,t817,t818,t819,t82,t820,t821,t822,t823,t824,t825,t826,t827,t83,t831,t832,t833,t834,t839,t84,t840,t843,t844,t845,t848,t849,t85,t850,t851,t852,t853,t854,t855,t857,t858,t86,t861,t862,t868,t869,t87,t870,t871,t872,t873,t874,t875,t876,t877,t878,t879,t88,t880,t881,t882,t883,t884,t885,t886,t887,t888,t889,t89,t890,t891,t892,t893,t894,t895,t896,t897,t898,t899,t9,t90,t900,t901,t902,t903,t904,t905,t906,t907,t908,t909,t91,t910,t911,t912,t913,t914,t915,t916,t917,t918,t919,t92,t920,t921,t922,t923,t924,t925,t926,t927,t928,t929,t93,t930,t931,t932,t933,t934,t935,t936,t938,t939,t94,t940,t941,t942,t943,t948,t949,t95,t950,t951,t952,t953,t954,t955,t956,t957,t958,t959,t96,t960,t961,t962,t963,t968,t969,t97,t970,t971,t972,t973,t974,t975,t976,t977,t978,t979,t98,t980,t981,t982,t983,t984,t985,t986,t987,t99,t991,t992,t995,t996] = ct{:};
t699 = -t376;
t700 = -t387;
t701 = -t388;
t702 = -t389;
t703 = -t390;
t704 = -t391;
t705 = -t392;
t706 = -t393;
t707 = -t394;
t708 = -t395;
t709 = -t396;
t710 = -t397;
t711 = -t398;
t745 = t36.*t94.*2.0;
t746 = t36.*t95.*2.0;
t747 = t36.*t96.*2.0;
t748 = t36.*t97.*2.0;
t749 = t35.*t98.*2.0;
t750 = t35.*t99.*2.0;
t751 = t36.*t100.*2.0;
t752 = t36.*t101.*2.0;
t753 = t36.*t102.*2.0;
t754 = t36.*t103.*2.0;
t755 = t35.*t104.*2.0;
t756 = t35.*t105.*2.0;
t828 = -t633;
t829 = -t634;
t830 = -t639;
t835 = -t640;
t836 = -t641;
t837 = -t642;
t838 = -t643;
t988 = -t757;
t989 = -t758;
t990 = -t763;
t993 = -t766;
t994 = -t767;
t997 = -t770;
t998 = -t771;
t1001 = -t772;
t1002 = -t773;
t1003 = -t784;
t1004 = -t786;
t1005 = -t787;
t1006 = -t789;
t1007 = -t790;
t1008 = -t796;
t1009 = -t797;
t1010 = -t799;
t1011 = -t802;
t1012 = -t805;
t1013 = -t808;
t1014 = -t811;
t1015 = -t812;
t1016 = -t813;
t1017 = -t814;
t1018 = -t815;
t1019 = -t816;
t1020 = -t817;
t1021 = -t818;
t1022 = -t819;
t1023 = -t820;
t1024 = -t821;
t1025 = -t822;
t1026 = -t823;
t1027 = -t824;
t1028 = -t825;
t1029 = -t826;
t1030 = -t827;
t1082 = -t850;
t1083 = -t853;
t1084 = -t854;
t1085 = -t855;
t1193 = t35.*t197.*2.0;
t1194 = t35.*t198.*2.0;
t1197 = t35.*t199.*2.0;
t1198 = t35.*t200.*2.0;
t1199 = t35.*t349;
t1200 = t35.*t351;
t1205 = t34.*t355;
t1206 = t34.*t356;
t1208 = t36.*t359;
t1209 = t35.*t201.*2.0;
t1210 = t35.*t202.*2.0;
t1211 = t35.*t203.*2.0;
t1212 = t35.*t204.*2.0;
t1381 = -t1191;
t1382 = -t1192;
t1383 = -t1195;
t1384 = -t1196;
t1385 = -t1201;
t1386 = -t1203;
t1420 = -t1220;
t1421 = -t1221;
t1422 = -t1222;
t1423 = -t1232;
t1424 = -t1233;
t1425 = -t1234;
t1426 = -t1235;
t1427 = -t1236;
t1428 = -t1237;
t1429 = -t1238;
t1430 = -t1239;
t1431 = -t1240;
t1432 = -t1241;
t1433 = -t970;
t1434 = -t971;
t1435 = -t974;
t1436 = -t975;
t1437 = -t1244;
t1438 = -t1245;
t1439 = -t1247;
t1440 = -t1248;
t1441 = -t976;
t1442 = -t977;
t1444 = -t1261;
t1445 = -t980;
t1446 = -t981;
t1447 = -t982;
t1448 = -t983;
t1450 = -t1268;
t1451 = -t986;
t1452 = -t987;
t1453 = -t1270;
t1454 = -t1271;
t1455 = -t1273;
t1456 = -t1274;
t1515 = -t1277;
t1516 = -t1280;
t1517 = -t1281;
t1523 = t34.*t766;
t1524 = t34.*t767;
t1525 = t34.*t770;
t1526 = t34.*t771;
t1531 = t35.*t781;
t1532 = t35.*t783;
t1533 = t34.*t784;
t1534 = t34.*t786;
t1535 = t35.*t785;
t1536 = t35.*t788;
t1539 = t34.*t796;
t1540 = t34.*t797;
t1547 = t35.*t816;
t1548 = t35.*t817;
t1549 = t35.*t818;
t1550 = t35.*t819;
t1644 = -t1463;
t1645 = -t1464;
t1646 = -t1465;
t1647 = -t1466;
t1648 = -t1467;
t1649 = -t1468;
t1650 = -t1470;
t1651 = -t1473;
t1657 = -t1483;
t1658 = -t1485;
t1659 = -t1486;
t1660 = -t1488;
t1661 = -t1489;
t1662 = -t1491;
t1663 = -t1492;
t1665 = -t1495;
t1759 = -t1527;
t1760 = -t1528;
t1763 = -t1537;
t1764 = -t1538;
t1775 = t35.*t850;
t1777 = -t1556;
t1778 = -t1557;
t1779 = -t1558;
t1780 = -t1559;
t1785 = -t1569;
t1786 = -t1570;
t1789 = -t1573;
t1790 = -t1574;
t1791 = -t1584;
t1794 = -t1587;
t1795 = -t1588;
t1799 = -t1607;
t1827 = -t1614;
t1828 = -t1615;
t1829 = -t1412;
t1830 = -t1413;
t1831 = -t1414;
t1832 = -t1616;
t1833 = -t1415;
t1834 = -t1416;
t1835 = -t1417;
t1840 = -t1418;
t1841 = -t1419;
t1939 = -t1757;
t1940 = -t1758;
t2034 = -t1805;
t2039 = -t1810;
t2040 = -t1811;
t2041 = -t1812;
t2042 = -t1813;
t2043 = -t1824;
t2044 = -t1825;
t2045 = -t1826;
t2082 = t36.*t1232;
t2087 = t36.*t978.*2.0;
t2088 = t36.*t979.*2.0;
t2089 = t36.*t984.*2.0;
t2090 = t36.*t985.*2.0;
t2094 = t35.*t1277;
t2103 = -t1941;
t2104 = -t1942;
t2105 = -t1943;
t2106 = -t1953;
t2107 = -t1954;
t2109 = -t1956;
t2110 = -t1957;
t2111 = -t1958;
t2112 = -t1963;
t2113 = -t1964;
t2115 = -t1966;
t2116 = -t1967;
t2117 = -t1968;
t2118 = -t1976;
t2121 = -t1979;
t2122 = -t1980;
t2128 = -t2007;
t2129 = -t2008;
t2130 = -t2009;
t2131 = -t2010;
t2132 = -t2011;
t2133 = -t2012;
t2134 = -t2013;
t2135 = -t2014;
t2136 = -t2015;
t2137 = -t2016;
t2138 = -t2017;
t2139 = -t2018;
t2140 = -t2019;
t2141 = -t2020;
t2142 = -t2021;
t2143 = -t2022;
t2144 = -t2028;
t2145 = -t2029;
t2153 = -t2052;
t2154 = -t2053;
t2194 = -t2080;
t2195 = -t2081;
t2206 = t36.*t1459;
t2207 = t36.*t1460;
t2218 = t36.*t1483;
t2219 = t36.*t1485;
t2220 = t36.*t1486;
t2221 = t36.*t1488;
t2222 = t35.*t1490;
t2223 = t35.*t1493;
t2247 = -t2146;
t2255 = t36.*t1398.*2.0;
t2256 = t36.*t1399.*2.0;
t2259 = t36.*t1405.*2.0;
t2260 = t36.*t1406.*2.0;
t2317 = t35.*t1761;
t2318 = t35.*t1762;
t2336 = t35.*t1787;
t2337 = t35.*t1788;
t2340 = t35.*t1792;
t2341 = t35.*t1793;
t2346 = t35.*t1805;
t2353 = t36.*t1848;
t2355 = -t2286;
t2366 = -t2303;
t2367 = -t2304;
t2368 = -t2305;
t2369 = -t2306;
t2370 = -t2307;
t2371 = -t2308;
t2372 = -t2309;
t2373 = -t2310;
t2374 = -t2311;
t2388 = -t2350;
t2389 = -t2351;
t2391 = -t2356;
t2392 = -t2357;
t2393 = -t2358;
t2394 = -t2359;
t2396 = t35.*t2119;
t2397 = t35.*t2120;
t2412 = -t2400;
t2413 = -t2401;
t2416 = t35.*t2277;
t2417 = t35.*t2278;
t964 = -t745;
t965 = -t747;
t966 = -t751;
t967 = -t753;
t1388 = -t1209;
t1389 = -t1210;
t1390 = -t1211;
t1391 = -t1212;
t1620 = t36.*t564.*2.0;
t1621 = t36.*t565.*2.0;
t1622 = t36.*t566.*2.0;
t1623 = t36.*t567.*2.0;
t2200 = -t2087;
t2201 = -t2088;
t2202 = -t2089;
t2203 = -t2090;
t2235 = t35.*t1539;
t2236 = t35.*t1540;
t2338 = -t2255;
t2339 = -t2256;
t2342 = -t2259;
t2343 = -t2260;
t2408 = t35.*t2206;
t2409 = t35.*t2207;
t1853 = -t1620;
t1854 = -t1621;
t1855 = -t1622;
t1856 = -t1623;
et1 = -Ixy6.*dQ1.*dQ6-Ixz2.*dQ1.*dQ2+Ixz3.*dQ1.*dQ2+Ixz3.*dQ1.*dQ3-Ixz5.*dQ1.*dQ5-Iyx6.*dQ1.*dQ6-Izx2.*dQ1.*dQ2+Izx3.*dQ1.*dQ2+Izx3.*dQ1.*dQ3-Izx5.*dQ1.*dQ5+Ixx2.*dQ1.*dQ2.*t37-Ixx3.*dQ1.*dQ2.*t37-Ixx3.*dQ1.*dQ2.*t38-Ixx3.*dQ1.*dQ3.*t37-Ixx3.*dQ1.*dQ3.*t38+Ixx5.*dQ1.*dQ2.*t37+Ixx5.*dQ1.*dQ2.*t38+Ixx5.*dQ1.*dQ3.*t37-Ixx6.*dQ1.*dQ2.*t37+Ixx5.*dQ1.*dQ3.*t38-Ixx6.*dQ1.*dQ2.*t38-Ixx6.*dQ1.*dQ3.*t37-Ixx6.*dQ1.*dQ3.*t38+Ixx5.*dQ1.*dQ5.*t40-Ixx6.*dQ1.*dQ6.*t41-Ixy4.*dQ1.*dQ4.*t32-Ixy4.*dQ1.*dQ4.*t33+Ixy6.*dQ1.*dQ6.*t32.*2.0+Ixy6.*dQ1.*dQ6.*t33.*2.0+Ixy6.*dQ1.*dQ6.*t35+Ixy6.*dQ1.*dQ6.*t36.*2.0+Ixz4.*dQ1.*dQ2.*t4+Ixz4.*dQ1.*dQ3.*t4-Ixz5.*dQ1.*dQ2.*t4;
et2 = -Ixz5.*dQ1.*dQ3.*t4-Ixz6.*dQ1.*dQ5.*t6+Ixz2.*dQ1.*dQ2.*t32.*2.0-Ixz3.*dQ1.*dQ2.*t32.*2.0-Ixz3.*dQ1.*dQ2.*t33.*2.0-Ixz3.*dQ1.*dQ3.*t32.*2.0-Ixz3.*dQ1.*dQ3.*t33.*2.0+Ixz5.*dQ1.*dQ5.*t32+Ixz5.*dQ1.*dQ5.*t33+Ixz5.*dQ1.*dQ5.*t35.*2.0-Iyx4.*dQ1.*dQ4.*t32-Iyx4.*dQ1.*dQ4.*t33+Iyx6.*dQ1.*dQ6.*t32.*2.0+Iyx6.*dQ1.*dQ6.*t33.*2.0+Iyx6.*dQ1.*dQ6.*t35+Iyx6.*dQ1.*dQ6.*t36.*2.0-Iyy4.*dQ1.*dQ2.*t37-Iyy4.*dQ1.*dQ2.*t38-Iyy4.*dQ1.*dQ3.*t37-Iyy5.*dQ1.*dQ2.*t37-Iyy4.*dQ1.*dQ3.*t38-Iyy5.*dQ1.*dQ2.*t38-Iyy5.*dQ1.*dQ3.*t37+Iyy6.*dQ1.*dQ2.*t37-Iyy5.*dQ1.*dQ3.*t38+Iyy6.*dQ1.*dQ2.*t38+Iyy6.*dQ1.*dQ3.*t37+Iyy6.*dQ1.*dQ3.*t38+Iyy6.*dQ1.*dQ5.*t40+Iyy6.*dQ1.*dQ6.*t41-Iyz4.*dQ1.*dQ2.*t9;
et3 = -Iyz4.*dQ1.*dQ3.*t9+Iyz6.*dQ1.*dQ5.*t11+Izx4.*dQ1.*dQ2.*t4+Izx4.*dQ1.*dQ3.*t4-Izx5.*dQ1.*dQ2.*t4-Izx5.*dQ1.*dQ3.*t4-Izx6.*dQ1.*dQ5.*t6+Izx2.*dQ1.*dQ2.*t32.*2.0-Izx3.*dQ1.*dQ2.*t32.*2.0-Izx3.*dQ1.*dQ2.*t33.*2.0-Izx3.*dQ1.*dQ3.*t32.*2.0-Izx3.*dQ1.*dQ3.*t33.*2.0+Izx5.*dQ1.*dQ5.*t32+Izx5.*dQ1.*dQ5.*t33+Izx5.*dQ1.*dQ5.*t35.*2.0-Izy4.*dQ1.*dQ2.*t9-Izy4.*dQ1.*dQ3.*t9+Izy6.*dQ1.*dQ5.*t11-Izz2.*dQ1.*dQ2.*t37+Izz3.*dQ1.*dQ2.*t37+Izz3.*dQ1.*dQ2.*t38+Izz3.*dQ1.*dQ3.*t37+Izz4.*dQ1.*dQ2.*t37+Izz3.*dQ1.*dQ3.*t38+Izz4.*dQ1.*dQ2.*t38+Izz4.*dQ1.*dQ3.*t37+Izz4.*dQ1.*dQ3.*t38-Izz5.*dQ1.*dQ5.*t40-Izz6.*dQ1.*dQ5.*t40-Lxcm6.*Lycm6.*dQ1.*dQ6.*m6.*2.0+Lx3.*Lz4.*dQ1.*dQ2.*m5.*2.0+Lx3.*Lz4.*dQ1.*dQ2.*m6.*2.0;
et4 = Lx3.*Lz4.*dQ1.*dQ3.*m5.*2.0+Lx3.*Lz4.*dQ1.*dQ3.*m6.*2.0+Lx3.*Lzcm4.*dQ1.*dQ2.*m4.*2.0+Lx3.*Lzcm4.*dQ1.*dQ3.*m4.*2.0-Lxcm2.*Lzcm2.*dQ1.*dQ2.*m2.*2.0+Lxcm3.*Lzcm3.*dQ1.*dQ2.*m3.*2.0+Lxcm3.*Lzcm3.*dQ1.*dQ3.*m3.*2.0-Lxcm5.*Lzcm5.*dQ1.*dQ5.*m5.*2.0+Ixx4.*dQ2.*dQ4.*t2.*t8+Ixx4.*dQ2.*dQ4.*t3.*t7+Ixx4.*dQ3.*dQ4.*t2.*t8+Ixx4.*dQ3.*dQ4.*t3.*t7-Ixx5.*dQ2.*dQ4.*t2.*t8-Ixx5.*dQ2.*dQ4.*t3.*t7-Ixx5.*dQ3.*dQ4.*t2.*t8-Ixx5.*dQ3.*dQ4.*t3.*t7-Ixx6.*dQ2.*dQ4.*t2.*t8-Ixx6.*dQ2.*dQ4.*t3.*t7-Ixx6.*dQ3.*dQ4.*t2.*t8-Ixx6.*dQ3.*dQ4.*t3.*t7+Ixy3.*dQ2.*dQ3.*t2.*t3-Ixy4.*dQ2.*dQ3.*t2.*t3-Ixy6.*dQ4.*dQ6.*t2.*t3-Ixy3.*dQ2.*dQ3.*t7.*t8+Ixy4.*dQ2.*dQ3.*t7.*t8+Ixy5.*dQ1.*dQ2.*t9.*t10+Ixy5.*dQ1.*dQ3.*t9.*t10;
et5 = -Ixy6.*dQ1.*dQ2.*t9.*t10-Ixy6.*dQ1.*dQ3.*t9.*t10+Ixy6.*dQ4.*dQ6.*t7.*t8-Ixy5.*dQ1.*dQ4.*t5.*t32-Ixy5.*dQ1.*dQ4.*t5.*t33+Ixy6.*dQ1.*dQ4.*t5.*t32+Ixy6.*dQ1.*dQ4.*t5.*t33+Ixy4.*dQ1.*dQ4.*t32.*t33.*2.0+Ixy4.*dQ1.*dQ4.*t32.*t34.*2.0+Ixy4.*dQ1.*dQ4.*t33.*t34.*2.0-Ixy6.*dQ1.*dQ6.*t32.*t33.*4.0-Ixy6.*dQ1.*dQ6.*t32.*t34-Ixy6.*dQ1.*dQ6.*t32.*t35-Ixy6.*dQ1.*dQ6.*t33.*t34-Ixy6.*dQ1.*dQ6.*t32.*t36.*4.0-Ixy6.*dQ1.*dQ6.*t33.*t35-Ixy6.*dQ1.*dQ6.*t33.*t36.*4.0-Ixy6.*dQ1.*dQ6.*t35.*t36.*2.0-Ixz5.*dQ4.*dQ5.*t2.*t3-Ixz6.*dQ1.*dQ2.*t4.*t6-Ixz6.*dQ1.*dQ3.*t4.*t6+Ixz5.*dQ4.*dQ5.*t7.*t8-Ixz4.*dQ1.*dQ2.*t4.*t32.*2.0-Ixz4.*dQ1.*dQ2.*t4.*t33.*2.0-Ixz4.*dQ1.*dQ3.*t4.*t32.*2.0+Ixz5.*dQ1.*dQ2.*t4.*t32.*2.0;
et6 = Ixz4.*dQ1.*dQ3.*t4.*t33.*-2.0+Ixz5.*dQ1.*dQ2.*t4.*t33.*2.0+Ixz5.*dQ1.*dQ3.*t4.*t32.*2.0+Ixz5.*dQ1.*dQ3.*t4.*t33.*2.0+Ixz5.*dQ1.*dQ2.*t4.*t35.*2.0+Ixz5.*dQ1.*dQ3.*t4.*t35.*2.0+Ixz6.*dQ1.*dQ5.*t6.*t32+Ixz6.*dQ1.*dQ5.*t6.*t33+Ixz6.*dQ1.*dQ5.*t6.*t35.*2.0+Ixz3.*dQ1.*dQ2.*t32.*t33.*4.0+Ixz3.*dQ1.*dQ3.*t32.*t33.*4.0-Ixz5.*dQ1.*dQ5.*t32.*t33.*2.0+Ixz5.*dQ1.*dQ5.*t32.*t34-Ixz5.*dQ1.*dQ5.*t32.*t35.*2.0+Ixz5.*dQ1.*dQ5.*t33.*t34-Ixz5.*dQ1.*dQ5.*t33.*t35.*2.0+Iyx3.*dQ2.*dQ3.*t2.*t3-Iyx4.*dQ2.*dQ3.*t2.*t3-Iyx6.*dQ4.*dQ6.*t2.*t3-Iyx3.*dQ2.*dQ3.*t7.*t8+Iyx4.*dQ2.*dQ3.*t7.*t8+Iyx5.*dQ1.*dQ2.*t9.*t10+Iyx5.*dQ1.*dQ3.*t9.*t10-Iyx6.*dQ1.*dQ2.*t9.*t10-Iyx6.*dQ1.*dQ3.*t9.*t10+Iyx6.*dQ4.*dQ6.*t7.*t8-Iyx5.*dQ1.*dQ4.*t5.*t32-Iyx5.*dQ1.*dQ4.*t5.*t33;
et7 = Iyx6.*dQ1.*dQ4.*t5.*t32+Iyx6.*dQ1.*dQ4.*t5.*t33+Iyx4.*dQ1.*dQ4.*t32.*t33.*2.0+Iyx4.*dQ1.*dQ4.*t32.*t34.*2.0+Iyx4.*dQ1.*dQ4.*t33.*t34.*2.0-Iyx6.*dQ1.*dQ6.*t32.*t33.*4.0-Iyx6.*dQ1.*dQ6.*t32.*t34-Iyx6.*dQ1.*dQ6.*t32.*t35-Iyx6.*dQ1.*dQ6.*t33.*t34-Iyx6.*dQ1.*dQ6.*t32.*t36.*4.0-Iyx6.*dQ1.*dQ6.*t33.*t35-Iyx6.*dQ1.*dQ6.*t33.*t36.*4.0-Iyx6.*dQ1.*dQ6.*t35.*t36.*2.0-Iyy4.*dQ2.*dQ4.*t2.*t8-Iyy4.*dQ2.*dQ4.*t3.*t7-Iyy4.*dQ3.*dQ4.*t2.*t8-Iyy4.*dQ3.*dQ4.*t3.*t7-Iyy5.*dQ2.*dQ4.*t2.*t8-Iyy5.*dQ2.*dQ4.*t3.*t7-Iyy5.*dQ3.*dQ4.*t2.*t8-Iyy5.*dQ3.*dQ4.*t3.*t7-Iyy6.*dQ2.*dQ4.*t2.*t8-Iyy6.*dQ2.*dQ4.*t3.*t7-Iyy6.*dQ3.*dQ4.*t2.*t8-Iyy6.*dQ3.*dQ4.*t3.*t7+Iyz3.*dQ2.*dQ3.*t2.*t8;
et8 = Iyz3.*dQ2.*dQ3.*t3.*t7-Iyz5.*dQ1.*dQ2.*t5.*t9-Iyz5.*dQ1.*dQ3.*t5.*t9+Iyz6.*dQ1.*dQ2.*t4.*t11+Iyz6.*dQ1.*dQ3.*t4.*t11+Iyz4.*dQ1.*dQ2.*t9.*t32.*2.0+Iyz4.*dQ1.*dQ2.*t9.*t33.*2.0+Iyz4.*dQ1.*dQ3.*t9.*t32.*2.0+Iyz4.*dQ1.*dQ3.*t9.*t33.*2.0-Iyz5.*dQ1.*dQ4.*t10.*t32-Iyz5.*dQ1.*dQ4.*t10.*t33-Iyz6.*dQ1.*dQ5.*t11.*t32-Iyz6.*dQ1.*dQ5.*t11.*t33-Iyz6.*dQ1.*dQ5.*t11.*t35.*2.0-Izx5.*dQ4.*dQ5.*t2.*t3-Izx6.*dQ1.*dQ2.*t4.*t6-Izx6.*dQ1.*dQ3.*t4.*t6+Izx5.*dQ4.*dQ5.*t7.*t8-Izx4.*dQ1.*dQ2.*t4.*t32.*2.0-Izx4.*dQ1.*dQ2.*t4.*t33.*2.0-Izx4.*dQ1.*dQ3.*t4.*t32.*2.0+Izx5.*dQ1.*dQ2.*t4.*t32.*2.0-Izx4.*dQ1.*dQ3.*t4.*t33.*2.0+Izx5.*dQ1.*dQ2.*t4.*t33.*2.0+Izx5.*dQ1.*dQ3.*t4.*t32.*2.0+Izx5.*dQ1.*dQ3.*t4.*t33.*2.0+Izx5.*dQ1.*dQ2.*t4.*t35.*2.0;
et9 = Izx5.*dQ1.*dQ3.*t4.*t35.*2.0+Izx6.*dQ1.*dQ5.*t6.*t32+Izx6.*dQ1.*dQ5.*t6.*t33+Izx6.*dQ1.*dQ5.*t6.*t35.*2.0+Izx3.*dQ1.*dQ2.*t32.*t33.*4.0+Izx3.*dQ1.*dQ3.*t32.*t33.*4.0-Izx5.*dQ1.*dQ5.*t32.*t33.*2.0+Izx5.*dQ1.*dQ5.*t32.*t34-Izx5.*dQ1.*dQ5.*t32.*t35.*2.0+Izx5.*dQ1.*dQ5.*t33.*t34-Izx5.*dQ1.*dQ5.*t33.*t35.*2.0+Izy3.*dQ2.*dQ3.*t2.*t8+Izy3.*dQ2.*dQ3.*t3.*t7-Izy5.*dQ1.*dQ2.*t5.*t9-Izy5.*dQ1.*dQ3.*t5.*t9+Izy6.*dQ1.*dQ2.*t4.*t11+Izy6.*dQ1.*dQ3.*t4.*t11+Izy4.*dQ1.*dQ2.*t9.*t32.*2.0+Izy4.*dQ1.*dQ2.*t9.*t33.*2.0+Izy4.*dQ1.*dQ3.*t9.*t32.*2.0+Izy4.*dQ1.*dQ3.*t9.*t33.*2.0-Izy5.*dQ1.*dQ4.*t10.*t32-Izy5.*dQ1.*dQ4.*t10.*t33-Izy6.*dQ1.*dQ5.*t11.*t32-Izy6.*dQ1.*dQ5.*t11.*t33-Izy6.*dQ1.*dQ5.*t11.*t35.*2.0-Izz4.*dQ2.*dQ4.*t2.*t8-Izz4.*dQ2.*dQ4.*t3.*t7;
et10 = -Izz4.*dQ3.*dQ4.*t2.*t8-Izz4.*dQ3.*dQ4.*t3.*t7+Izz5.*dQ2.*dQ4.*t2.*t8+Izz5.*dQ2.*dQ4.*t3.*t7+Izz5.*dQ3.*dQ4.*t2.*t8+Izz5.*dQ3.*dQ4.*t3.*t7+Izz6.*dQ2.*dQ4.*t2.*t8+Izz6.*dQ2.*dQ4.*t3.*t7+Izz6.*dQ3.*dQ4.*t2.*t8+Izz6.*dQ3.*dQ4.*t3.*t7-dQ1.*dQ2.*m3.*t12.*t37-dQ1.*dQ2.*m4.*t12.*t37+dQ1.*dQ2.*m3.*t14.*t37+dQ1.*dQ2.*m4.*t13.*t37-dQ1.*dQ2.*m5.*t12.*t37+dQ1.*dQ2.*m3.*t14.*t38+dQ1.*dQ2.*m4.*t13.*t38+dQ1.*dQ2.*m5.*t13.*t37-dQ1.*dQ2.*m6.*t12.*t37+dQ1.*dQ3.*m3.*t14.*t37+dQ1.*dQ3.*m4.*t13.*t37+dQ1.*dQ2.*m5.*t13.*t38+dQ1.*dQ2.*m6.*t13.*t37+dQ1.*dQ3.*m3.*t14.*t38+dQ1.*dQ3.*m4.*t13.*t38+dQ1.*dQ3.*m5.*t13.*t37+dQ1.*dQ2.*m6.*t13.*t38+dQ1.*dQ3.*m5.*t13.*t38+dQ1.*dQ3.*m6.*t13.*t37-dQ1.*dQ2.*m5.*t16.*t37+dQ1.*dQ3.*m6.*t13.*t38;
et11 = dQ1.*dQ2.*m4.*t18.*t37-dQ1.*dQ2.*m5.*t16.*t38-dQ1.*dQ3.*m5.*t16.*t37+dQ1.*dQ2.*m4.*t18.*t38+dQ1.*dQ2.*m6.*t17.*t37+dQ1.*dQ3.*m4.*t18.*t37-dQ1.*dQ3.*m5.*t16.*t38+dQ1.*dQ2.*m5.*t19.*t37+dQ1.*dQ2.*m6.*t17.*t38+dQ1.*dQ3.*m4.*t18.*t38+dQ1.*dQ3.*m6.*t17.*t37+dQ1.*dQ2.*m5.*t19.*t38+dQ1.*dQ3.*m5.*t19.*t37+dQ1.*dQ3.*m6.*t17.*t38-dQ1.*dQ2.*m3.*t23.*t37-dQ1.*dQ2.*m5.*t21.*t37-dQ1.*dQ2.*m6.*t20.*t37+dQ1.*dQ3.*m5.*t19.*t38-dQ1.*dQ2.*m3.*t23.*t38-dQ1.*dQ2.*m5.*t21.*t38-dQ1.*dQ2.*m6.*t20.*t38-dQ1.*dQ2.*m6.*t21.*t37-dQ1.*dQ3.*m3.*t23.*t37-dQ1.*dQ3.*m5.*t21.*t37-dQ1.*dQ3.*m6.*t20.*t37-dQ1.*dQ5.*m5.*t16.*t40-dQ1.*dQ2.*m4.*t24.*t37-dQ1.*dQ2.*m6.*t21.*t38;
